simulink model "simulator_prototype_v2"  (R2021b)
(part 8 of 12)

tau_c = ft_11({t1005,t1022,t1089,t1104,t1105,t1108,t1115,t1121,t1158,t1159,t1196,t1205,t1207,t1208,t1210,t1212,t1217,t1218,t1221,t123,t1230,t1235,t1237,t1238,t1288,t1289,t1302,t1303,t1319,t1320,t1336,t1348,t1350,t1351,t1360,t1369,t1378,t1396,t14,t140,t1425,t1435,t1456,t1477,t1488,t15,t1513,t1539,t1544,t1547,t1548,t1553,t1554,t1559,t1564,t1576,t1577,t1578,t1579,t1584,t1585,t1586,t1587,t1591,t1599,t16,t1600,t1602,t1604,t1605,t1606,t1607,t1608,t1609,t1613,t1614,t1615,t1616,t1626,t1627,t1628,t1629,t1631,t1637,t1640,t1641,t1648,t1649,t1659,t1660,t1661,t1666,t1667,t1683,t1686,t1690,t1692,t17,t1700,t1701,t1704,t1705,t1712,t1717,t1738,t1741,t1742,t1750,t1752,t1753,t1754,t1758,t1759,t1775,t1776,t18,t1861,t1874,t1879,t188,t1881,t189,t1896,t19,t1901,t1941,t1959,t1973,t1993,t1994,t2,t20,t201,t202,t2023,t2053,t2060,t2089,t2090,t2098,t2099,t21,t2117,t2120,t2122,t2123,t2125,t2137,t2139,t2140,t2142,t2147,t2149,t2150,t2151,t2152,t2154,t2155,t2159,t2164,t2165,t2166,t2167,t2168,t2174,t2183,t2187,t2193,t2194,t2195,t2199,t22,t2203,t2215,t2219,t2222,t2223,t2239,t2240,t2256,t2257,t2291,t2292,t2293,t2294,t2295,t2297,t2298,t2299,t23,t2301,t2302,t2303,t2304,t2306,t2307,t2308,t2311,t2317,t2320,t2323,t2325,t2326,t2329,t2337,t2338,t2339,t2341,t2343,t2344,t2352,t2353,t2355,t2359,t236,t2360,t2361,t2362,t2363,t2364,t2365,t2366,t2367,t2368,t2369,t237,t2370,t2371,t2378,t2379,t238,t2380,t2384,t2388,t2389,t2391,t2394,t2395,t2397,t2398,t24,t2400,t2401,t2403,t2404,t2405,t241,t2414,t2419,t2421,t2423,t2438,t244,t2448,t2449,t2461,t2471,t2472,t2492,t2493,t2494,t25,t2502,t2510,t2519,t2527,t2530,t2534,t2555,t2556,t2572,t2575,t2583,t2598,t26,t2605,t2606,t2612,t2613,t2618,t2619,t262,t2638,t264,t2651,t2652,t2670,t2671,t2673,t2674,t2675,t2676,t2678,t2680,t2683,t2684,t2685,t2686,t2687,t2689,t2690,t2692,t2693,t2694,t2695,t2696,t2697,t2698,t27,t2700,t2701,t2704,t2705,t2707,t2708,t2709,t2711,t2712,t2713,t2715,t2716,t2717,t2719,t2720,t2721,t2736,t2740,t2744,t2745,t2747,t2748,t2749,t2750,t2754,t2759,t2773,t2774,t2777,t2778,t2779,t2781,t2785,t2786,t2787,t2788,t2797,t28,t2801,t2804,t2813,t2814,t2820,t2831,t2834,t2835,t2838,t2850,t2851,t2937,t2942,t2945,t2946,t2950,t2951,t2953,t2954,t2955,t2956,t2957,t2963,t2964,t2975,t2978,t2979,t2984,t2987,t2990,t2991,t2993,t2994,t2998,t3,t30,t3003,t3004,t3008,t3009,t3015,t3017,t3022,t3027,t3029,t3030,t3036,t3043,t3044,t3045,t3047,t3049,t3050,t3051,t3054,t3055,t3056,t3057,t3063,t3064,t3066,t3067,t3068,t3072,t3073,t3079,t3080,t3081,t3085,t3086,t3087,t3088,t3096,t3097,t31,t3109,t3117,t3118,t3121,t3122,t3128,t3129,t313,t3130,t3131,t3132,t3133,t3134,t3135,t3139,t314,t3140,t3141,t3142,t3144,t3147,t3149,t3152,t3153,t3155,t3156,t3157,t3158,t3159,t3160,t3161,t3162,t3163,t3164,t3166,t3170,t3171,t3172,t3179,t3180,t3184,t3186,t3187,t3188,t3189,t3190,t3191,t3193,t3194,t3196,t3197,t3198,t3199,t32,t3200,t3201,t3204,t3206,t3209,t321,t3210,t3212,t3214,t3218,t3223,t3224,t3225,t3226,t3227,t3228,t3229,t3230,t3231,t3232,t3235,t3245,t3246,t3247,t3249,t3250,t3252,t3253,t3254,t3256,t3258,t3259,t326,t3260,t3261,t3262,t3263,t3264,t3265,t3266,t3269,t3270,t3271,t3272,t3275,t3276,t3277,t328,t3280,t3281,t3283,t3284,t3287,t329,t3290,t3291,t3292,t3293,t3295,t3296,t3297,t3298,t33,t3300,t3302,t3303,t3305,t3306,t3307,t3308,t3309,t331,t3313,t3316,t3318,t3319,t332,t3322,t3323,t3324,t3325,t3326,t3327,t3328,t333,t3330,t3331,t3333,t3334,t3335,t3336,t3337,t3338,t3340,t3341,t3342,t3343,t3344,t3345,t3347,t3348,t3349,t335,t3351,t3353,t3354,t3355,t3357,t3358,t3359,t3360,t3367,t3369,t3373,t3376,t3377,t3379,t338,t3382,t3384,t3385,t3386,t3389,t339,t3392,t3395,t3399,t34,t3405,t3408,t3409,t3410,t3412,t3415,t3417,t3419,t3420,t3421,t3422,t3423,t3424,t3427,t3428,t3429,t3430,t3432,t3433,t3434,t3435,t3436,t3437,t3438,t3440,t3441,t3442,t3443,t3444,t3445,t3446,t3447,t3449,t3450,t3451,t3453,t3455,t3456,t3457,t3458,t346,t3465,t3468,t3470,t3473,t3475,t3477,t3479,t3480,t3481,t3483,t3484,t3489,t3491,t3493,t3498,t35,t350,t3500,t3503,t3505,t3508,t3509,t351,t3510,t3512,t3513,t3515,t3518,t3522,t3524,t3526,t3527,t3528,t3530,t3531,t3532,t3533,t3535,t3539,t354,t3542,t3543,t3544,t3547,t3549,t3550,t3558,t3559,t356,t3560,t3561,t3562,t3563,t3564,t3565,t3567,t3569,t3570,t3571,t3572,t3573,t3576,t3577,t3578,t3579,t358,t3580,t3581,t3582,t3584,t3585,t3586,t3587,t3588,t3589,t359,t3590,t3591,t3593,t3595,t3596,t3597,t3598,t36,t360,t3600,t3603,t3605,t3607,t3609,t3610,t3611,t3612,t3613,t3614,t3615,t3616,t3617,t3618,t3619,t362,t3620,t3621,t3622,t3623,t3624,t3625,t3626,t3627,t3628,t3629,t363,t3630,t3631,t3632,t3633,t3634,t3635,t3636,t3637,t3638,t3639,t364,t3640,t3641,t3643,t3645,t3646,t3647,t3648,t3649,t365,t3650,t3651,t3652,t3653,t3654,t3656,t3657,t3658,t3659,t366,t3660,t3662,t3663,t3664,t3665,t3667,t3669,t3670,t3672,t3673,t3674,t3676,t3677,t3678,t3679,t3680,t3681,t3682,t3683,t3684,t3685,t3686,t3687,t3688,t3689,t3690,t3693,t3694,t3696,t3698,t3699,t3700,t3703,t3705,t3706,t3708,t3709,t371,t3711,t3712,t3713,t3714,t3715,t3716,t3718,t372,t3720,t3723,t3724,t3726,t3728,t3729,t3730,t3731,t3732,t3734,t3735,t3736,t3737,t3741,t3744,t3745,t3746,t3748,t3749,t3751,t3753,t3755,t3756,t3757,t3758,t3759,t3760,t3762,t3763,t3764,t3765,t3766,t3767,t3768,t3769,t3770,t3771,t3772,t3774,t3775,t3776,t3778,t3779,t378,t3782,t3783,t3784,t3788,t3789,t3790,t3791,t3793,t3794,t3795,t3797,t3798,t3799,t38,t380,t3801,t3803,t3804,t3805,t3806,t3811,t3814,t3815,t3816,t3817,t3819,t382,t3821,t3822,t3826,t3827,t3828,t3830,t3833,t3834,t3837,t3838,t3841,t3844,t3845,t3847,t3849,t3850,t3856,t3859,t3860,t3861,t3862,t3863,t3865,t3866,t3868,t3869,t387,t3870,t3871,t3872,t3875,t3876,t3877,t3880,t3882,t3886,t3891,t3892,t3893,t3898,t39,t3901,t3904,t3906,t3908,t3910,t3916,t3918,t3920,t3921,t3922,t3925,t3926,t3927,t3928,t3933,t3934,t3936,t3937,t3939,t3940,t3941,t3942,t3943,t3945,t3946,t3949,t3951,t3953,t3954,t3957,t3958,t3959,t3962,t3963,t3964,t3965,t3967,t3968,t3974,t3976,t3977,t3978,t3980,t3981,t3982,t3983,t3984,t3985,t3992,t3996,t3997,t4,t4002,t4007,t4008,t4009,t4010,t4011,t4012,t4021,t4022,t4025,t4026,t4027,t4028,t4033,t4048,t4052,t4053,t4054,t4058,t4059,t4060,t4061,t4062,t4063,t4065,t4067,t4069,t4070,t4071,t4072,t4073,t4074,t4078,t4079,t4080,t4083,t4084,t410,t4106,t4108,t4109,t4111,t4113,t4118,t4119,t4120,t4121,t4122,t4125,t4127,t4133,t4134,t4141,t4142,t4149,t4150,t4151,t4152,t4154,t4155,t4157,t4160,t4162,t4163,t4166,t4168,t4170,t4173,t4175,t4178,t4179,t4184,t4189,t4190,t4196,t4197,t42,t4200,t4201,t4202,t4203,t4205,t4207,t4208,t4217,t4219,t4220,t4221,t4224,t4227,t4228,t4230,t4231,t4233,t4234,t4235,t4236,t4237,t4238,t4239,t4240,t4242,t4243,t4244,t4245,t4246,t4247,t4249,t4250,t4251,t4252,t4253,t4254,t4255,t4256,t4257,t4259,t4260,t4261,t4262,t4263,t4264,t4266,t4267,t4268,t4274,t4275,t4277,t4278,t4279,t4280,t4281,t4285,t4286,t4287,t4288,t429,t4291,t4292,t4295,t4296,t4297,t4298,t4299,t43,t4304,t4306,t4307,t4308,t4310,t4311,t4313,t4314,t4321,t4322,t4323,t4324,t4326,t4353,t4354,t4355,t4356,t4357,t4359,t4362,t4363,t4367,t4369,t4370,t4373,t4374,t4375,t4376,t4377,t4378,t4379,t4381,t4382,t4383,t4385,t4386,t4387,t4388,t4390,t4395,t4396,t4400,t4402,t4403,t4404,t4405,t4406,t4407,t4409,t4410,t4411,t4412,t4413,t4415,t4421,t4424,t4427,t4428,t4429,t4430,t4431,t4432,t4434,t4435,t4436,t4437,t4438,t4439,t4440,t4441,t4442,t4443,t4444,t4447,t4453,t4458,t4460,t4461,t4464,t4470,t4473,t4474,t4475,t4480,t4481,t4483,t4484,t4486,t4487,t4488,t4489,t4491,t4492,t4496,t4498,t4499,t4500,t4501,t4502,t4504,t4507,t4508,t4510,t4511,t4513,t4514,t4515,t4516,t4517,t4520,t4521,t4522,t4525,t4526,t4528,t4530,t4531,t4532,t4533,t4535,t4536,t4539,t4542,t4543,t4545,t4546,t4549,t4550,t4551,t4552,t4555,t4560,t4562,t4563,t4571,t4572,t4574,t4579,t4581,t4582,t4583,t4584,t4585,t4586,t4587,t4588,t4589,t4591,t4593,t4594,t4595,t4597,t4599,t46,t4602,t4604,t4606,t4607,t4609,t4610,t4611,t4612,t4613,t4614,t4615,t4617,t4618,t4619,t4620,t4621,t4622,t4623,t4624,t4627,t4628,t4629,t4631,t4633,t4640,t4641,t4642,t4644,t4645,t4647,t4649,t4650,t4651,t4652,t4655,t4657,t4658,t4661,t4663,t4664,t4665,t4666,t4667,t4669,t4670,t4672,t4673,t4676,t4678,t4679,t4680,t4682,t4683,t4684,t4685,t4686,t4688,t4699,t47,t4702,t4703,t4704,t4705,t4706,t4708,t4709,t4710,t4711,t4716,t4718,t4719,t4720,t4721,t4723,t4725,t4726,t4727,t4728,t4729,t4732,t4733,t4734,t4735,t4736,t4737,t4738,t4740,t4741,t4742,t4744,t4746,t4749,t4756,t4758,t4759,t4760,t4762,t4764,t4768,t4769,t4770,t4772,t4777,t4780,t4785,t4786,t4787,t4788,t4789,t4790,t4791,t4792,t4795,t4798,t4799,t4800,t4801,t4805,t4809,t4814,t4816,t4817,t4818,t4819,t4822,t4823,t4824,t4826,t4828,t4829,t4832,t4833,t4836,t4839,t4840,t4842,t4843,t4845,t4846,t4847,t4849,t4852,t4856,t4857,t4860,t4863,t4864,t4865,t4866,t4867,t4868,t4869,t4870,t4871,t4872,t4873,t4874,t4875,t4876,t4877,t4880,t4881,t4882,t4883,t4884,t4885,t4886,t4887,t4888,t4890,t4892,t4893,t4894,t4897,t4898,t4899,t4900,t4902,t4905,t4911,t4917,t4921,t4922,t4925,t4927,t4931,t4950,t4952,t4953,t4954,t4961,t4962,t4963,t4965,t4968,t4969,t4973,t4974,t4975,t4976,t4977,t4982,t4983,t4984,t4985,t4986,t4987,t4992,t4994,t4995,t4996,t4998,t5,t50,t5000,t5001,t5002,t5005,t5007,t5010,t5012,t5013,t5014,t5015,t5017,t5021,t5022,t5023,t5025,t5026,t5027,t5028,t5030,t5031,t5032,t5033,t5034,t5035,t5036,t5038,t5039,t5040,t5041,t5042,t5047,t5048,t5049,t5051,t5052,t5053,t5054,t5056,t5058,t5061,t5063,t5064,t5067,t5068,t5069,t5073,t5074,t5076,t5077,t5091,t5092,t5094,t5096,t5105,t5108,t5111,t5113,t5114,t5115,t5116,t5118,t5119,t5121,t5123,t5124,t5126,t5127,t5128,t5130,t5131,t5144,t5145,t5146,t5147,t5148,t5149,t5150,t5151,t5152,t5153,t5155,t5158,t5162,t5164,t5165,t5169,t5184,t5189,t5190,t5191,t5192,t5193,t5195,t5196,t5198,t5201,t5202,t5203,t5204,t5206,t5207,t5208,t5209,t5210,t5211,t5212,t5213,t5214,t5216,t5217,t5218,t5219,t5221,t5222,t5223,t5224,t5225,t5226,t5227,t5228,t5229,t5230,t5231,t5232,t5233,t5234,t5235,t5236,t5237,t5238,t5239,t5240,t5241,t5242,t5243,t5244,t5245,t5246,t5247,t5248,t5249,t5250,t5252,t5254,t5255,t5257,t5260,t5261,t5263,t5265,t5266,t5267,t5269,t5270,t5272,t5273,t5274,t5275,t5276,t5277,t5281,t5282,t5285,t5288,t5289,t5290,t5291,t5293,t5295,t5298,t5299,t5301,t5302,t5303,t5304,t5306,t5307,t5308,t5316,t5317,t5320,t5322,t5325,t5328,t5330,t5331,t5332,t5335,t5337,t5338,t5339,t5340,t5342,t5344,t5345,t5346,t5347,t5348,t5349,t5350,t5356,t5357,t5358,t5361,t5362,t5365,t5369,t5370,t5377,t5379,t5380,t5381,t5383,t5384,t5385,t5386,t5387,t5388,t5389,t5390,t5391,t5392,t5393,t5395,t5396,t5399,t5402,t5403,t5405,t5407,t5408,t5409,t5411,t5412,t5418,t5420,t5427,t5428,t5433,t5434,t5440,t5441,t5443,t5444,t5445,t5446,t5449,t5455,t5458,t5461,t5462,t5465,t5480,t5481,t5482,t5483,t5484,t5485,t5486,t5487,t5488,t5489,t5490,t5491,t5492,t5493,t5494,t5496,t5498,t5499,t5500,t5504,t5505,t5509,t5510,t5514,t5515,t5516,t5517,t5518,t5522,t5523,t5524,t5525,t5531,t5535,t5536,t5537,t5540,t5544,t5547,t5550,t5552,t5553,t5554,t5556,t5557,t5565,t5566,t5571,t5578,t5580,t5595,t56,t5601,t5603,t5605,t5619,t5620,t5626,t5627,t5631,t5639,t5640,t5646,t5661,t5662,t5663,t5670,t5671,t5674,t5675,t5677,t5678,t5679,t5681,t5682,t5684,t5694,t5695,t5699,t5700,t5701,t5702,t5703,t5709,t5717,t5718,t5720,t5721,t5722,t5723,t5724,t5730,t5734,t5750,t5760,t5764,t5769,t5791,t5792,t5794,t58,t5832,t5835,t5839,t5840,t5846,t5852,t5853,t5857,t5864,t5866,t5871,t5876,t5879,t5890,t5891,t59,t5900,t5909,t5911,t5930,t5932,t5941,t5943,t5944,t5951,t5953,t5954,t5977,t5992,t5994,t5995,t6,t60,t6004,t6017,t6018,t6020,t6057,t6058,t6065,t6075,t6095,t6135,t6151,t6153,t6183,t6184,t6185,t6199,t6206,t6207,t6209,t6219,t6221,t6247,t6253,t628,t6317,t6321,t6323,t6339,t6341,t6367,t6375,t638,t640,t6405,t642,t643,t6450,t6484,t6485,t6486,t649,t6493,t6507,t6508,t6511,t6515,t6516,t654,t6543,t6544,t655,t656,t6565,t657,t659,t660,t665,t6658,t6663,t667,t668,t6689,t669,t6691,t6692,t67,t670,t672,t673,t674,t675,t676,t677,t68,t681,t6811,t6812,t6813,t682,t684,t685,t686,t6861,t687,t6892,t6893,t691,t6916,t692,t693,t694,t6980,t6981,t7,t70,t702,t7029,t7039,t7041,t7043,t7051,t7064,t707,t708,t71,t710,t715,t716,t717,t718,t7204,t721,t7219,t722,t7227,t7228,t7229,t7230,t724,t725,t73,t736,t738,t740,t741,t749,t756,t76,t762,t768,t777,t792,t793,t801,t802,t808,t813,t819,t821,t850,t855,t874,t878,t89,t90,t91,t92,t941,t944,t948,t951,t97});
end
function tau_c = ft_11(ct)
t1005 = ct{1};
t1022 = ct{2};
t1089 = ct{3};
t1104 = ct{4};
t1105 = ct{5};
t1108 = ct{6};
t1115 = ct{7};
t1121 = ct{8};
t1158 = ct{9};
t1159 = ct{10};
t1196 = ct{11};
t1205 = ct{12};
t1207 = ct{13};
t1208 = ct{14};
t1210 = ct{15};
t1212 = ct{16};
t1217 = ct{17};
t1218 = ct{18};
t1221 = ct{19};
t123 = ct{20};
t1230 = ct{21};
t1235 = ct{22};
t1237 = ct{23};
t1238 = ct{24};
t1288 = ct{25};
t1289 = ct{26};
t1302 = ct{27};
t1303 = ct{28};
t1319 = ct{29};
t1320 = ct{30};
t1336 = ct{31};
t1348 = ct{32};
t1350 = ct{33};
t1351 = ct{34};
t1360 = ct{35};
t1369 = ct{36};
t1378 = ct{37};
t1396 = ct{38};
t14 = ct{39};
t140 = ct{40};
t1425 = ct{41};
t1435 = ct{42};
t1456 = ct{43};
t1477 = ct{44};
t1488 = ct{45};
t15 = ct{46};
t1513 = ct{47};
t1539 = ct{48};
t1544 = ct{49};
t1547 = ct{50};
t1548 = ct{51};
t1553 = ct{52};
t1554 = ct{53};
t1559 = ct{54};
t1564 = ct{55};
t1576 = ct{56};
t1577 = ct{57};
t1578 = ct{58};
t1579 = ct{59};
t1584 = ct{60};
t1585 = ct{61};
t1586 = ct{62};
t1587 = ct{63};
t1591 = ct{64};
t1599 = ct{65};
t16 = ct{66};
t1600 = ct{67};
t1602 = ct{68};
t1604 = ct{69};
t1605 = ct{70};
t1606 = ct{71};
t1607 = ct{72};
t1608 = ct{73};
t1609 = ct{74};
t1613 = ct{75};
t1614 = ct{76};
t1615 = ct{77};
t1616 = ct{78};
t1626 = ct{79};
t1627 = ct{80};
t1628 = ct{81};
t1629 = ct{82};
t1631 = ct{83};
t1637 = ct{84};
t1640 = ct{85};
t1641 = ct{86};
t1648 = ct{87};
t1649 = ct{88};
t1659 = ct{89};
t1660 = ct{90};
t1661 = ct{91};
t1666 = ct{92};
t1667 = ct{93};
t1683 = ct{94};
t1686 = ct{95};
t1690 = ct{96};
t1692 = ct{97};
t17 = ct{98};
t1700 = ct{99};
t1701 = ct{100};
t1704 = ct{101};
t1705 = ct{102};
t1712 = ct{103};
t1717 = ct{104};
t1738 = ct{105};
t1741 = ct{106};
t1742 = ct{107};
t1750 = ct{108};
t1752 = ct{109};
t1753 = ct{110};
t1754 = ct{111};
t1758 = ct{112};
t1759 = ct{113};
t1775 = ct{114};
t1776 = ct{115};
t18 = ct{116};
t1861 = ct{117};
t1874 = ct{118};
t1879 = ct{119};
t188 = ct{120};
t1881 = ct{121};
t189 = ct{122};
t1896 = ct{123};
t19 = ct{124};
t1901 = ct{125};
t1941 = ct{126};
t1959 = ct{127};
t1973 = ct{128};
t1993 = ct{129};
t1994 = ct{130};
t2 = ct{131};
t20 = ct{132};
t201 = ct{133};
t202 = ct{134};
t2023 = ct{135};
t2053 = ct{136};
t2060 = ct{137};
t2089 = ct{138};
t2090 = ct{139};
t2098 = ct{140};
t2099 = ct{141};
t21 = ct{142};
t2117 = ct{143};
t2120 = ct{144};
t2122 = ct{145};
t2123 = ct{146};
t2125 = ct{147};
t2137 = ct{148};
t2139 = ct{149};
t2140 = ct{150};
t2142 = ct{151};
t2147 = ct{152};
t2149 = ct{153};
t2150 = ct{154};
t2151 = ct{155};
t2152 = ct{156};
t2154 = ct{157};
t2155 = ct{158};
t2159 = ct{159};
t2164 = ct{160};
t2165 = ct{161};
t2166 = ct{162};
t2167 = ct{163};
t2168 = ct{164};
t2174 = ct{165};
t2183 = ct{166};
t2187 = ct{167};
t2193 = ct{168};
t2194 = ct{169};
t2195 = ct{170};
t2199 = ct{171};
t22 = ct{172};
t2203 = ct{173};
t2215 = ct{174};
t2219 = ct{175};
t2222 = ct{176};
t2223 = ct{177};
t2239 = ct{178};
t2240 = ct{179};
t2256 = ct{180};
t2257 = ct{181};
t2291 = ct{182};
t2292 = ct{183};
t2293 = ct{184};
t2294 = ct{185};
t2295 = ct{186};
t2297 = ct{187};
t2298 = ct{188};
t2299 = ct{189};
t23 = ct{190};
t2301 = ct{191};
t2302 = ct{192};
t2303 = ct{193};
t2304 = ct{194};
t2306 = ct{195};
t2307 = ct{196};
t2308 = ct{197};
t2311 = ct{198};
t2317 = ct{199};
t2320 = ct{200};
t2323 = ct{201};
t2325 = ct{202};
t2326 = ct{203};
t2329 = ct{204};
t2337 = ct{205};
t2338 = ct{206};
t2339 = ct{207};
t2341 = ct{208};
t2343 = ct{209};
t2344 = ct{210};
t2352 = ct{211};
t2353 = ct{212};
t2355 = ct{213};
t2359 = ct{214};
t236 = ct{215};
t2360 = ct{216};
t2361 = ct{217};
t2362 = ct{218};
t2363 = ct{219};
t2364 = ct{220};
t2365 = ct{221};
t2366 = ct{222};
t2367 = ct{223};
t2368 = ct{224};
t2369 = ct{225};
t237 = ct{226};
t2370 = ct{227};
t2371 = ct{228};
t2378 = ct{229};
t2379 = ct{230};
t238 = ct{231};
t2380 = ct{232};
t2384 = ct{233};
t2388 = ct{234};
t2389 = ct{235};
t2391 = ct{236};
t2394 = ct{237};
t2395 = ct{238};
t2397 = ct{239};
t2398 = ct{240};
t24 = ct{241};
t2400 = ct{242};
t2401 = ct{243};
t2403 = ct{244};
t2404 = ct{245};
t2405 = ct{246};
t241 = ct{247};
t2414 = ct{248};
t2419 = ct{249};
t2421 = ct{250};
t2423 = ct{251};
t2438 = ct{252};
t244 = ct{253};
t2448 = ct{254};
t2449 = ct{255};
t2461 = ct{256};
t2471 = ct{257};
t2472 = ct{258};
t2492 = ct{259};
t2493 = ct{260};
t2494 = ct{261};
t25 = ct{262};
t2502 = ct{263};
t2510 = ct{264};
t2519 = ct{265};
t2527 = ct{266};
t2530 = ct{267};
t2534 = ct{268};
t2555 = ct{269};
t2556 = ct{270};
t2572 = ct{271};
t2575 = ct{272};
t2583 = ct{273};
t2598 = ct{274};
t26 = ct{275};
t2605 = ct{276};
t2606 = ct{277};
t2612 = ct{278};
t2613 = ct{279};
t2618 = ct{280};
t2619 = ct{281};
t262 = ct{282};
t2638 = ct{283};
t264 = ct{284};
t2651 = ct{285};
t2652 = ct{286};
t2670 = ct{287};
t2671 = ct{288};
t2673 = ct{289};
t2674 = ct{290};
t2675 = ct{291};
t2676 = ct{292};
t2678 = ct{293};
t2680 = ct{294};
t2683 = ct{295};
t2684 = ct{296};
t2685 = ct{297};
t2686 = ct{298};
t2687 = ct{299};
t2689 = ct{300};
t2690 = ct{301};
t2692 = ct{302};
t2693 = ct{303};
t2694 = ct{304};
t2695 = ct{305};
t2696 = ct{306};
t2697 = ct{307};
t2698 = ct{308};
t27 = ct{309};
t2700 = ct{310};
t2701 = ct{311};
t2704 = ct{312};
t2705 = ct{313};
t2707 = ct{314};
t2708 = ct{315};
t2709 = ct{316};
t2711 = ct{317};
t2712 = ct{318};
t2713 = ct{319};
t2715 = ct{320};
t2716 = ct{321};
t2717 = ct{322};
t2719 = ct{323};
t2720 = ct{324};
t2721 = ct{325};
t2736 = ct{326};
t2740 = ct{327};
t2744 = ct{328};
t2745 = ct{329};
t2747 = ct{330};
t2748 = ct{331};
t2749 = ct{332};
t2750 = ct{333};
t2754 = ct{334};
t2759 = ct{335};
t2773 = ct{336};
t2774 = ct{337};
t2777 = ct{338};
t2778 = ct{339};
t2779 = ct{340};
t2781 = ct{341};
t2785 = ct{342};
t2786 = ct{343};
t2787 = ct{344};
t2788 = ct{345};
t2797 = ct{346};
t28 = ct{347};
t2801 = ct{348};
t2804 = ct{349};
t2813 = ct{350};
t2814 = ct{351};
t2820 = ct{352};
t2831 = ct{353};
t2834 = ct{354};
t2835 = ct{355};
t2838 = ct{356};
t2850 = ct{357};
t2851 = ct{358};
t2937 = ct{359};
t2942 = ct{360};
t2945 = ct{361};
t2946 = ct{362};
t2950 = ct{363};
t2951 = ct{364};
t2953 = ct{365};
t2954 = ct{366};
t2955 = ct{367};
t2956 = ct{368};
t2957 = ct{369};
t2963 = ct{370};
t2964 = ct{371};
t2975 = ct{372};
t2978 = ct{373};
t2979 = ct{374};
t2984 = ct{375};
t2987 = ct{376};
t2990 = ct{377};
t2991 = ct{378};
t2993 = ct{379};
t2994 = ct{380};
t2998 = ct{381};
t3 = ct{382};
t30 = ct{383};
t3003 = ct{384};
t3004 = ct{385};
t3008 = ct{386};
t3009 = ct{387};
t3015 = ct{388};
t3017 = ct{389};
t3022 = ct{390};
t3027 = ct{391};
t3029 = ct{392};
t3030 = ct{393};
t3036 = ct{394};
t3043 = ct{395};
t3044 = ct{396};
t3045 = ct{397};
t3047 = ct{398};
t3049 = ct{399};
t3050 = ct{400};
t3051 = ct{401};
t3054 = ct{402};
t3055 = ct{403};
t3056 = ct{404};
t3057 = ct{405};
t3063 = ct{406};
t3064 = ct{407};
t3066 = ct{408};
t3067 = ct{409};
t3068 = ct{410};
t3072 = ct{411};
t3073 = ct{412};
t3079 = ct{413};
t3080 = ct{414};
t3081 = ct{415};
t3085 = ct{416};
t3086 = ct{417};
t3087 = ct{418};
t3088 = ct{419};
t3096 = ct{420};
t3097 = ct{421};
t31 = ct{422};
t3109 = ct{423};
t3117 = ct{424};
t3118 = ct{425};
t3121 = ct{426};
t3122 = ct{427};
t3128 = ct{428};
t3129 = ct{429};
t313 = ct{430};
t3130 = ct{431};
t3131 = ct{432};
t3132 = ct{433};
t3133 = ct{434};
t3134 = ct{435};
t3135 = ct{436};
t3139 = ct{437};
t314 = ct{438};
t3140 = ct{439};
t3141 = ct{440};
t3142 = ct{441};
t3144 = ct{442};
t3147 = ct{443};
t3149 = ct{444};
t3152 = ct{445};
t3153 = ct{446};
t3155 = ct{447};
t3156 = ct{448};
t3157 = ct{449};
t3158 = ct{450};
t3159 = ct{451};
t3160 = ct{452};
t3161 = ct{453};
t3162 = ct{454};
t3163 = ct{455};
t3164 = ct{456};
t3166 = ct{457};
t3170 = ct{458};
t3171 = ct{459};
t3172 = ct{460};
t3179 = ct{461};
t3180 = ct{462};
t3184 = ct{463};
t3186 = ct{464};
t3187 = ct{465};
t3188 = ct{466};
t3189 = ct{467};
t3190 = ct{468};
t3191 = ct{469};
t3193 = ct{470};
t3194 = ct{471};
t3196 = ct{472};
t3197 = ct{473};
t3198 = ct{474};
t3199 = ct{475};
t32 = ct{476};
t3200 = ct{477};
t3201 = ct{478};
t3204 = ct{479};
t3206 = ct{480};
t3209 = ct{481};
t321 = ct{482};
t3210 = ct{483};
t3212 = ct{484};
t3214 = ct{485};
t3218 = ct{486};
t3223 = ct{487};
t3224 = ct{488};
t3225 = ct{489};
t3226 = ct{490};
t3227 = ct{491};
t3228 = ct{492};
t3229 = ct{493};
t3230 = ct{494};
t3231 = ct{495};
t3232 = ct{496};
t3235 = ct{497};
t3245 = ct{498};
t3246 = ct{499};
t3247 = ct{500};
t3249 = ct{501};
t3250 = ct{502};
t3252 = ct{503};
t3253 = ct{504};
t3254 = ct{505};
t3256 = ct{506};
t3258 = ct{507};
t3259 = ct{508};
t326 = ct{509};
t3260 = ct{510};
t3261 = ct{511};
t3262 = ct{512};
t3263 = ct{513};
t3264 = ct{514};
t3265 = ct{515};
t3266 = ct{516};
t3269 = ct{517};
t3270 = ct{518};
t3271 = ct{519};
t3272 = ct{520};
t3275 = ct{521};
t3276 = ct{522};
t3277 = ct{523};
t328 = ct{524};
t3280 = ct{525};
t3281 = ct{526};
t3283 = ct{527};
t3284 = ct{528};
t3287 = ct{529};
t329 = ct{530};
t3290 = ct{531};
t3291 = ct{532};
t3292 = ct{533};
t3293 = ct{534};
t3295 = ct{535};
t3296 = ct{536};
t3297 = ct{537};
t3298 = ct{538};
t33 = ct{539};
t3300 = ct{540};
t3302 = ct{541};
t3303 = ct{542};
t3305 = ct{543};
t3306 = ct{544};
t3307 = ct{545};
t3308 = ct{546};
t3309 = ct{547};
t331 = ct{548};
t3313 = ct{549};
t3316 = ct{550};
t3318 = ct{551};
t3319 = ct{552};
t332 = ct{553};
t3322 = ct{554};
t3323 = ct{555};
t3324 = ct{556};
t3325 = ct{557};
t3326 = ct{558};
t3327 = ct{559};
t3328 = ct{560};
t333 = ct{561};
t3330 = ct{562};
t3331 = ct{563};
t3333 = ct{564};
t3334 = ct{565};
t3335 = ct{566};
t3336 = ct{567};
t3337 = ct{568};
t3338 = ct{569};
t3340 = ct{570};
t3341 = ct{571};
t3342 = ct{572};
t3343 = ct{573};
t3344 = ct{574};
t3345 = ct{575};
t3347 = ct{576};
t3348 = ct{577};
t3349 = ct{578};
t335 = ct{579};
t3351 = ct{580};
t3353 = ct{581};
t3354 = ct{582};
t3355 = ct{583};
t3357 = ct{584};
t3358 = ct{585};
t3359 = ct{586};
t3360 = ct{587};
t3367 = ct{588};
t3369 = ct{589};
t3373 = ct{590};
t3376 = ct{591};
t3377 = ct{592};
t3379 = ct{593};
t338 = ct{594};
t3382 = ct{595};
t3384 = ct{596};
t3385 = ct{597};
t3386 = ct{598};
t3389 = ct{599};
t339 = ct{600};
t3392 = ct{601};
t3395 = ct{602};
t3399 = ct{603};
t34 = ct{604};
t3405 = ct{605};
t3408 = ct{606};
t3409 = ct{607};
t3410 = ct{608};
t3412 = ct{609};
t3415 = ct{610};
t3417 = ct{611};
t3419 = ct{612};
t3420 = ct{613};
t3421 = ct{614};
t3422 = ct{615};
t3423 = ct{616};
t3424 = ct{617};
t3427 = ct{618};
t3428 = ct{619};
t3429 = ct{620};
t3430 = ct{621};
t3432 = ct{622};
t3433 = ct{623};
t3434 = ct{624};
t3435 = ct{625};
t3436 = ct{626};
t3437 = ct{627};
t3438 = ct{628};
t3440 = ct{629};
t3441 = ct{630};
t3442 = ct{631};
t3443 = ct{632};
t3444 = ct{633};
t3445 = ct{634};
t3446 = ct{635};
t3447 = ct{636};
t3449 = ct{637};
t3450 = ct{638};
t3451 = ct{639};
t3453 = ct{640};
t3455 = ct{641};
t3456 = ct{642};
t3457 = ct{643};
t3458 = ct{644};
t346 = ct{645};
t3465 = ct{646};
t3468 = ct{647};
t3470 = ct{648};
t3473 = ct{649};
t3475 = ct{650};
t3477 = ct{651};
t3479 = ct{652};
t3480 = ct{653};
t3481 = ct{654};
t3483 = ct{655};
t3484 = ct{656};
t3489 = ct{657};
t3491 = ct{658};
t3493 = ct{659};
t3498 = ct{660};
t35 = ct{661};
t350 = ct{662};
t3500 = ct{663};
t3503 = ct{664};
t3505 = ct{665};
t3508 = ct{666};
t3509 = ct{667};
t351 = ct{668};
t3510 = ct{669};
t3512 = ct{670};
t3513 = ct{671};
t3515 = ct{672};
t3518 = ct{673};
t3522 = ct{674};
t3524 = ct{675};
t3526 = ct{676};
t3527 = ct{677};
t3528 = ct{678};
t3530 = ct{679};
t3531 = ct{680};
t3532 = ct{681};
t3533 = ct{682};
t3535 = ct{683};
t3539 = ct{684};
t354 = ct{685};
t3542 = ct{686};
t3543 = ct{687};
t3544 = ct{688};
t3547 = ct{689};
t3549 = ct{690};
t3550 = ct{691};
t3558 = ct{692};
t3559 = ct{693};
t356 = ct{694};
t3560 = ct{695};
t3561 = ct{696};
t3562 = ct{697};
t3563 = ct{698};
t3564 = ct{699};
t3565 = ct{700};
t3567 = ct{701};
t3569 = ct{702};
t3570 = ct{703};
t3571 = ct{704};
t3572 = ct{705};
t3573 = ct{706};
t3576 = ct{707};
t3577 = ct{708};
t3578 = ct{709};
t3579 = ct{710};
t358 = ct{711};
t3580 = ct{712};
t3581 = ct{713};
t3582 = ct{714};
t3584 = ct{715};
t3585 = ct{716};
t3586 = ct{717};
t3587 = ct{718};
t3588 = ct{719};
t3589 = ct{720};
t359 = ct{721};
t3590 = ct{722};
t3591 = ct{723};
t3593 = ct{724};
t3595 = ct{725};
t3596 = ct{726};
t3597 = ct{727};
t3598 = ct{728};
t36 = ct{729};
t360 = ct{730};
t3600 = ct{731};
t3603 = ct{732};
t3605 = ct{733};
t3607 = ct{734};
t3609 = ct{735};
t3610 = ct{736};
t3611 = ct{737};
t3612 = ct{738};
t3613 = ct{739};
t3614 = ct{740};
t3615 = ct{741};
t3616 = ct{742};
t3617 = ct{743};
t3618 = ct{744};
t3619 = ct{745};
t362 = ct{746};
t3620 = ct{747};
t3621 = ct{748};
t3622 = ct{749};
t3623 = ct{750};
t3624 = ct{751};
t3625 = ct{752};
t3626 = ct{753};
t3627 = ct{754};
t3628 = ct{755};
t3629 = ct{756};
t363 = ct{757};
t3630 = ct{758};
t3631 = ct{759};
t3632 = ct{760};
t3633 = ct{761};
t3634 = ct{762};
t3635 = ct{763};
t3636 = ct{764};
t3637 = ct{765};
t3638 = ct{766};
t3639 = ct{767};
t364 = ct{768};
t3640 = ct{769};
t3641 = ct{770};
t3643 = ct{771};
t3645 = ct{772};
t3646 = ct{773};
t3647 = ct{774};
t3648 = ct{775};
t3649 = ct{776};
t365 = ct{777};
t3650 = ct{778};
t3651 = ct{779};
t3652 = ct{780};
t3653 = ct{781};
t3654 = ct{782};
t3656 = ct{783};
t3657 = ct{784};
t3658 = ct{785};
t3659 = ct{786};
t366 = ct{787};
t3660 = ct{788};
t3662 = ct{789};
t3663 = ct{790};
t3664 = ct{791};
t3665 = ct{792};
t3667 = ct{793};
t3669 = ct{794};
t3670 = ct{795};
t3672 = ct{796};
t3673 = ct{797};
t3674 = ct{798};
t3676 = ct{799};
t3677 = ct{800};
t3678 = ct{801};
t3679 = ct{802};
t3680 = ct{803};
t3681 = ct{804};
t3682 = ct{805};
t3683 = ct{806};
t3684 = ct{807};
t3685 = ct{808};
t3686 = ct{809};
t3687 = ct{810};
t3688 = ct{811};
t3689 = ct{812};
t3690 = ct{813};
t3693 = ct{814};
t3694 = ct{815};
t3696 = ct{816};
t3698 = ct{817};
t3699 = ct{818};
t3700 = ct{819};
t3703 = ct{820};
t3705 = ct{821};
t3706 = ct{822};
t3708 = ct{823};
t3709 = ct{824};
t371 = ct{825};
t3711 = ct{826};
t3712 = ct{827};
t3713 = ct{828};
t3714 = ct{829};
t3715 = ct{830};
t3716 = ct{831};
t3718 = ct{832};
t372 = ct{833};
t3720 = ct{834};
t3723 = ct{835};
t3724 = ct{836};
t3726 = ct{837};
t3728 = ct{838};
t3729 = ct{839};
t3730 = ct{840};
t3731 = ct{841};
t3732 = ct{842};
t3734 = ct{843};
t3735 = ct{844};
t3736 = ct{845};
t3737 = ct{846};
t3741 = ct{847};
t3744 = ct{848};
t3745 = ct{849};
t3746 = ct{850};
t3748 = ct{851};
t3749 = ct{852};
t3751 = ct{853};
t3753 = ct{854};
t3755 = ct{855};
t3756 = ct{856};
t3757 = ct{857};
t3758 = ct{858};
t3759 = ct{859};
t3760 = ct{860};
t3762 = ct{861};
t3763 = ct{862};
t3764 = ct{863};
t3765 = ct{864};
t3766 = ct{865};
t3767 = ct{866};
t3768 = ct{867};
t3769 = ct{868};
t3770 = ct{869};
t3771 = ct{870};
t3772 = ct{871};
t3774 = ct{872};
t3775 = ct{873};
t3776 = ct{874};
t3778 = ct{875};
t3779 = ct{876};
t378 = ct{877};
t3782 = ct{878};
t3783 = ct{879};
t3784 = ct{880};
t3788 = ct{881};
t3789 = ct{882};
t3790 = ct{883};
t3791 = ct{884};
t3793 = ct{885};
t3794 = ct{886};
t3795 = ct{887};
t3797 = ct{888};
t3798 = ct{889};
t3799 = ct{890};
t38 = ct{891};
t380 = ct{892};
t3801 = ct{893};
t3803 = ct{894};
t3804 = ct{895};
t3805 = ct{896};
t3806 = ct{897};
t3811 = ct{898};
t3814 = ct{899};
t3815 = ct{900};
t3816 = ct{901};
t3817 = ct{902};
t3819 = ct{903};
t382 = ct{904};
t3821 = ct{905};
t3822 = ct{906};
t3826 = ct{907};
t3827 = ct{908};
t3828 = ct{909};
t3830 = ct{910};
t3833 = ct{911};
t3834 = ct{912};
t3837 = ct{913};
t3838 = ct{914};
t3841 = ct{915};
t3844 = ct{916};
t3845 = ct{917};
t3847 = ct{918};
t3849 = ct{919};
t3850 = ct{920};
t3856 = ct{921};
t3859 = ct{922};
t3860 = ct{923};
t3861 = ct{924};
t3862 = ct{925};
t3863 = ct{926};
t3865 = ct{927};
t3866 = ct{928};
t3868 = ct{929};
t3869 = ct{930};
t387 = ct{931};
t3870 = ct{932};
t3871 = ct{933};
t3872 = ct{934};
t3875 = ct{935};
t3876 = ct{936};
t3877 = ct{937};
t3880 = ct{938};
t3882 = ct{939};
t3886 = ct{940};
t3891 = ct{941};
t3892 = ct{942};
t3893 = ct{943};
t3898 = ct{944};
t39 = ct{945};
t3901 = ct{946};
t3904 = ct{947};
t3906 = ct{948};
t3908 = ct{949};
t3910 = ct{950};
t3916 = ct{951};
t3918 = ct{952};
t3920 = ct{953};
t3921 = ct{954};
t3922 = ct{955};
t3925 = ct{956};
t3926 = ct{957};
t3927 = ct{958};
t3928 = ct{959};
t3933 = ct{960};
t3934 = ct{961};
t3936 = ct{962};
t3937 = ct{963};
t3939 = ct{964};
t3940 = ct{965};
t3941 = ct{966};
t3942 = ct{967};
t3943 = ct{968};
t3945 = ct{969};
t3946 = ct{970};
t3949 = ct{971};
t3951 = ct{972};
t3953 = ct{973};
t3954 = ct{974};
t3957 = ct{975};
t3958 = ct{976};
t3959 = ct{977};
t3962 = ct{978};
t3963 = ct{979};
t3964 = ct{980};
t3965 = ct{981};
t3967 = ct{982};
t3968 = ct{983};
t3974 = ct{984};
t3976 = ct{985};
t3977 = ct{986};
t3978 = ct{987};
t3980 = ct{988};
t3981 = ct{989};
t3982 = ct{990};
t3983 = ct{991};
t3984 = ct{992};
t3985 = ct{993};
t3992 = ct{994};
t3996 = ct{995};
t3997 = ct{996};
t4 = ct{997};
t4002 = ct{998};
t4007 = ct{999};
t4008 = ct{1000};
t4009 = ct{1001};
t4010 = ct{1002};
t4011 = ct{1003};
t4012 = ct{1004};
t4021 = ct{1005};
t4022 = ct{1006};
t4025 = ct{1007};
t4026 = ct{1008};
t4027 = ct{1009};
t4028 = ct{1010};
t4033 = ct{1011};
t4048 = ct{1012};
t4052 = ct{1013};
t4053 = ct{1014};
t4054 = ct{1015};
t4058 = ct{1016};
t4059 = ct{1017};
t4060 = ct{1018};
t4061 = ct{1019};
t4062 = ct{1020};
t4063 = ct{1021};
t4065 = ct{1022};
t4067 = ct{1023};
t4069 = ct{1024};
t4070 = ct{1025};
t4071 = ct{1026};
t4072 = ct{1027};
t4073 = ct{1028};
t4074 = ct{1029};
t4078 = ct{1030};
t4079 = ct{1031};
t4080 = ct{1032};
t4083 = ct{1033};
t4084 = ct{1034};
t410 = ct{1035};
t4106 = ct{1036};
t4108 = ct{1037};
t4109 = ct{1038};
t4111 = ct{1039};
t4113 = ct{1040};
t4118 = ct{1041};
t4119 = ct{1042};
t4120 = ct{1043};
t4121 = ct{1044};
t4122 = ct{1045};
t4125 = ct{1046};
t4127 = ct{1047};
t4133 = ct{1048};
t4134 = ct{1049};
t4141 = ct{1050};
t4142 = ct{1051};
t4149 = ct{1052};
t4150 = ct{1053};
t4151 = ct{1054};
t4152 = ct{1055};
t4154 = ct{1056};
t4155 = ct{1057};
t4157 = ct{1058};
t4160 = ct{1059};
t4162 = ct{1060};
t4163 = ct{1061};
t4166 = ct{1062};
t4168 = ct{1063};
t4170 = ct{1064};
t4173 = ct{1065};
t4175 = ct{1066};
t4178 = ct{1067};
t4179 = ct{1068};
t4184 = ct{1069};
t4189 = ct{1070};
t4190 = ct{1071};
t4196 = ct{1072};
t4197 = ct{1073};
t42 = ct{1074};
t4200 = ct{1075};
t4201 = ct{1076};
t4202 = ct{1077};
t4203 = ct{1078};
t4205 = ct{1079};
t4207 = ct{1080};
t4208 = ct{1081};
t4217 = ct{1082};
t4219 = ct{1083};
t4220 = ct{1084};
t4221 = ct{1085};
t4224 = ct{1086};
t4227 = ct{1087};
t4228 = ct{1088};
t4230 = ct{1089};
t4231 = ct{1090};
t4233 = ct{1091};
t4234 = ct{1092};
t4235 = ct{1093};
t4236 = ct{1094};
t4237 = ct{1095};
t4238 = ct{1096};
t4239 = ct{1097};
t4240 = ct{1098};
t4242 = ct{1099};
t4243 = ct{1100};
t4244 = ct{1101};
t4245 = ct{1102};
t4246 = ct{1103};
t4247 = ct{1104};
t4249 = ct{1105};
t4250 = ct{1106};
t4251 = ct{1107};
t4252 = ct{1108};
t4253 = ct{1109};
t4254 = ct{1110};
t4255 = ct{1111};
t4256 = ct{1112};
t4257 = ct{1113};
t4259 = ct{1114};
t4260 = ct{1115};
t4261 = ct{1116};
t4262 = ct{1117};
t4263 = ct{1118};
t4264 = ct{1119};
t4266 = ct{1120};
t4267 = ct{1121};
t4268 = ct{1122};
t4274 = ct{1123};
t4275 = ct{1124};
t4277 = ct{1125};
t4278 = ct{1126};
t4279 = ct{1127};
t4280 = ct{1128};
t4281 = ct{1129};
t4285 = ct{1130};
t4286 = ct{1131};
t4287 = ct{1132};
t4288 = ct{1133};
t429 = ct{1134};
t4291 = ct{1135};
t4292 = ct{1136};
t4295 = ct{1137};
t4296 = ct{1138};
t4297 = ct{1139};
t4298 = ct{1140};
t4299 = ct{1141};
t43 = ct{1142};
t4304 = ct{1143};
t4306 = ct{1144};
t4307 = ct{1145};
t4308 = ct{1146};
t4310 = ct{1147};
t4311 = ct{1148};
t4313 = ct{1149};
t4314 = ct{1150};
t4321 = ct{1151};
t4322 = ct{1152};
t4323 = ct{1153};
t4324 = ct{1154};
t4326 = ct{1155};
t4353 = ct{1156};
t4354 = ct{1157};
t4355 = ct{1158};
t4356 = ct{1159};
t4357 = ct{1160};
t4359 = ct{1161};
t4362 = ct{1162};
t4363 = ct{1163};
t4367 = ct{1164};
t4369 = ct{1165};
t4370 = ct{1166};
t4373 = ct{1167};
t4374 = ct{1168};
t4375 = ct{1169};
t4376 = ct{1170};
t4377 = ct{1171};
t4378 = ct{1172};
t4379 = ct{1173};
t4381 = ct{1174};
t4382 = ct{1175};
t4383 = ct{1176};
t4385 = ct{1177};
t4386 = ct{1178};
t4387 = ct{1179};
t4388 = ct{1180};
t4390 = ct{1181};
t4395 = ct{1182};
t4396 = ct{1183};
t4400 = ct{1184};
t4402 = ct{1185};
t4403 = ct{1186};
t4404 = ct{1187};
t4405 = ct{1188};
t4406 = ct{1189};
t4407 = ct{1190};
t4409 = ct{1191};
t4410 = ct{1192};
t4411 = ct{1193};
t4412 = ct{1194};
t4413 = ct{1195};
t4415 = ct{1196};
t4421 = ct{1197};
t4424 = ct{1198};
t4427 = ct{1199};
t4428 = ct{1200};
t4429 = ct{1201};
t4430 = ct{1202};
t4431 = ct{1203};
t4432 = ct{1204};
t4434 = ct{1205};
t4435 = ct{1206};
t4436 = ct{1207};
t4437 = ct{1208};
t4438 = ct{1209};
t4439 = ct{1210};
t4440 = ct{1211};
t4441 = ct{1212};
t4442 = ct{1213};
t4443 = ct{1214};
t4444 = ct{1215};
t4447 = ct{1216};
t4453 = ct{1217};
t4458 = ct{1218};
t4460 = ct{1219};
t4461 = ct{1220};
t4464 = ct{1221};
t4470 = ct{1222};
t4473 = ct{1223};
t4474 = ct{1224};
t4475 = ct{1225};
t4480 = ct{1226};
t4481 = ct{1227};
t4483 = ct{1228};
t4484 = ct{1229};
t4486 = ct{1230};
t4487 = ct{1231};
t4488 = ct{1232};
t4489 = ct{1233};
t4491 = ct{1234};
t4492 = ct{1235};
t4496 = ct{1236};
t4498 = ct{1237};
t4499 = ct{1238};
t4500 = ct{1239};
t4501 = ct{1240};
t4502 = ct{1241};
t4504 = ct{1242};
t4507 = ct{1243};
t4508 = ct{1244};
t4510 = ct{1245};
t4511 = ct{1246};
t4513 = ct{1247};
t4514 = ct{1248};
t4515 = ct{1249};
t4516 = ct{1250};
t4517 = ct{1251};
t4520 = ct{1252};
t4521 = ct{1253};
t4522 = ct{1254};
t4525 = ct{1255};
t4526 = ct{1256};
t4528 = ct{1257};
t4530 = ct{1258};
t4531 = ct{1259};
t4532 = ct{1260};
t4533 = ct{1261};
t4535 = ct{1262};
t4536 = ct{1263};
t4539 = ct{1264};
t4542 = ct{1265};
t4543 = ct{1266};
t4545 = ct{1267};
t4546 = ct{1268};
t4549 = ct{1269};
t4550 = ct{1270};
t4551 = ct{1271};
t4552 = ct{1272};
t4555 = ct{1273};
t4560 = ct{1274};
t4562 = ct{1275};
t4563 = ct{1276};
t4571 = ct{1277};
t4572 = ct{1278};
t4574 = ct{1279};
t4579 = ct{1280};
t4581 = ct{1281};
t4582 = ct{1282};
t4583 = ct{1283};
t4584 = ct{1284};
t4585 = ct{1285};
t4586 = ct{1286};
t4587 = ct{1287};
t4588 = ct{1288};
t4589 = ct{1289};
t4591 = ct{1290};
t4593 = ct{1291};
t4594 = ct{1292};
t4595 = ct{1293};
t4597 = ct{1294};
t4599 = ct{1295};
t46 = ct{1296};
t4602 = ct{1297};
t4604 = ct{1298};
t4606 = ct{1299};
t4607 = ct{1300};
t4609 = ct{1301};
t4610 = ct{1302};
t4611 = ct{1303};
t4612 = ct{1304};
t4613 = ct{1305};
t4614 = ct{1306};
t4615 = ct{1307};
t4617 = ct{1308};
t4618 = ct{1309};
t4619 = ct{1310};
t4620 = ct{1311};
t4621 = ct{1312};
t4622 = ct{1313};
t4623 = ct{1314};
t4624 = ct{1315};
t4627 = ct{1316};
t4628 = ct{1317};
t4629 = ct{1318};
t4631 = ct{1319};
t4633 = ct{1320};
t4640 = ct{1321};
t4641 = ct{1322};
t4642 = ct{1323};
t4644 = ct{1324};
t4645 = ct{1325};
t4647 = ct{1326};
t4649 = ct{1327};
t4650 = ct{1328};
t4651 = ct{1329};
t4652 = ct{1330};
t4655 = ct{1331};
t4657 = ct{1332};
t4658 = ct{1333};
t4661 = ct{1334};
t4663 = ct{1335};
t4664 = ct{1336};
t4665 = ct{1337};
t4666 = ct{1338};
t4667 = ct{1339};
t4669 = ct{1340};
t4670 = ct{1341};
t4672 = ct{1342};
t4673 = ct{1343};
t4676 = ct{1344};
t4678 = ct{1345};
t4679 = ct{1346};
t4680 = ct{1347};
t4682 = ct{1348};
t4683 = ct{1349};
t4684 = ct{1350};
t4685 = ct{1351};
t4686 = ct{1352};
t4688 = ct{1353};
t4699 = ct{1354};
t47 = ct{1355};
t4702 = ct{1356};
t4703 = ct{1357};
t4704 = ct{1358};
t4705 = ct{1359};
t4706 = ct{1360};
t4708 = ct{1361};
t4709 = ct{1362};
t4710 = ct{1363};
t4711 = ct{1364};
t4716 = ct{1365};
t4718 = ct{1366};
t4719 = ct{1367};
t4720 = ct{1368};
t4721 = ct{1369};
t4723 = ct{1370};
t4725 = ct{1371};
t4726 = ct{1372};
t4727 = ct{1373};
t4728 = ct{1374};
t4729 = ct{1375};
t4732 = ct{1376};
t4733 = ct{1377};
t4734 = ct{1378};
t4735 = ct{1379};
t4736 = ct{1380};
t4737 = ct{1381};
t4738 = ct{1382};
t4740 = ct{1383};
t4741 = ct{1384};
t4742 = ct{1385};
t4744 = ct{1386};
t4746 = ct{1387};
t4749 = ct{1388};
t4756 = ct{1389};
t4758 = ct{1390};
t4759 = ct{1391};
t4760 = ct{1392};
t4762 = ct{1393};
t4764 = ct{1394};
t4768 = ct{1395};
t4769 = ct{1396};
t4770 = ct{1397};
t4772 = ct{1398};
t4777 = ct{1399};
t4780 = ct{1400};
t4785 = ct{1401};
t4786 = ct{1402};
t4787 = ct{1403};
t4788 = ct{1404};
t4789 = ct{1405};
t4790 = ct{1406};
t4791 = ct{1407};
t4792 = ct{1408};
t4795 = ct{1409};
t4798 = ct{1410};
t4799 = ct{1411};
t4800 = ct{1412};
t4801 = ct{1413};
t4805 = ct{1414};
t4809 = ct{1415};
t4814 = ct{1416};
t4816 = ct{1417};
t4817 = ct{1418};
t4818 = ct{1419};
t4819 = ct{1420};
t4822 = ct{1421};
t4823 = ct{1422};
t4824 = ct{1423};
t4826 = ct{1424};
t4828 = ct{1425};
t4829 = ct{1426};
t4832 = ct{1427};
t4833 = ct{1428};
t4836 = ct{1429};
t4839 = ct{1430};
t4840 = ct{1431};
t4842 = ct{1432};
t4843 = ct{1433};
t4845 = ct{1434};
t4846 = ct{1435};
t4847 = ct{1436};
t4849 = ct{1437};
t4852 = ct{1438};
t4856 = ct{1439};
t4857 = ct{1440};
t4860 = ct{1441};
t4863 = ct{1442};
t4864 = ct{1443};
t4865 = ct{1444};
t4866 = ct{1445};
t4867 = ct{1446};
t4868 = ct{1447};
t4869 = ct{1448};
t4870 = ct{1449};
t4871 = ct{1450};
t4872 = ct{1451};
t4873 = ct{1452};
t4874 = ct{1453};
t4875 = ct{1454};
t4876 = ct{1455};
t4877 = ct{1456};
t4880 = ct{1457};
t4881 = ct{1458};
t4882 = ct{1459};
t4883 = ct{1460};
t4884 = ct{1461};
t4885 = ct{1462};
t4886 = ct{1463};
t4887 = ct{1464};
t4888 = ct{1465};
t4890 = ct{1466};
t4892 = ct{1467};
t4893 = ct{1468};
t4894 = ct{1469};
t4897 = ct{1470};
t4898 = ct{1471};
t4899 = ct{1472};
t4900 = ct{1473};
t4902 = ct{1474};
t4905 = ct{1475};
t4911 = ct{1476};
t4917 = ct{1477};
t4921 = ct{1478};
t4922 = ct{1479};
t4925 = ct{1480};
t4927 = ct{1481};
t4931 = ct{1482};
t4950 = ct{1483};
t4952 = ct{1484};
t4953 = ct{1485};
t4954 = ct{1486};
t4961 = ct{1487};
t4962 = ct{1488};
t4963 = ct{1489};
t4965 = ct{1490};
t4968 = ct{1491};
t4969 = ct{1492};
t4973 = ct{1493};
t4974 = ct{1494};
t4975 = ct{1495};
t4976 = ct{1496};
t4977 = ct{1497};
t4982 = ct{1498};
t4983 = ct{1499};
t4984 = ct{1500};
t4985 = ct{1501};
t4986 = ct{1502};
t4987 = ct{1503};
t4992 = ct{1504};
t4994 = ct{1505};
t4995 = ct{1506};
t4996 = ct{1507};
t4998 = ct{1508};
t5 = ct{1509};
t50 = ct{1510};
t5000 = ct{1511};
t5001 = ct{1512};
t5002 = ct{1513};
t5005 = ct{1514};
t5007 = ct{1515};
t5010 = ct{1516};
t5012 = ct{1517};
t5013 = ct{1518};
t5014 = ct{1519};
t5015 = ct{1520};
t5017 = ct{1521};
t5021 = ct{1522};
t5022 = ct{1523};
t5023 = ct{1524};
t5025 = ct{1525};
t5026 = ct{1526};
t5027 = ct{1527};
t5028 = ct{1528};
t5030 = ct{1529};
t5031 = ct{1530};
t5032 = ct{1531};
t5033 = ct{1532};
t5034 = ct{1533};
t5035 = ct{1534};
t5036 = ct{1535};
t5038 = ct{1536};
t5039 = ct{1537};
t5040 = ct{1538};
t5041 = ct{1539};
t5042 = ct{1540};
t5047 = ct{1541};
t5048 = ct{1542};
t5049 = ct{1543};
t5051 = ct{1544};
t5052 = ct{1545};
t5053 = ct{1546};
t5054 = ct{1547};
t5056 = ct{1548};
t5058 = ct{1549};
t5061 = ct{1550};
t5063 = ct{1551};
t5064 = ct{1552};
t5067 = ct{1553};
t5068 = ct{1554};
t5069 = ct{1555};
t5073 = ct{1556};
t5074 = ct{1557};
t5076 = ct{1558};
t5077 = ct{1559};
t5091 = ct{1560};
t5092 = ct{1561};
t5094 = ct{1562};
t5096 = ct{1563};
t5105 = ct{1564};
t5108 = ct{1565};
t5111 = ct{1566};
t5113 = ct{1567};
t5114 = ct{1568};
t5115 = ct{1569};
t5116 = ct{1570};
t5118 = ct{1571};
t5119 = ct{1572};
t5121 = ct{1573};
t5123 = ct{1574};
t5124 = ct{1575};
t5126 = ct{1576};
t5127 = ct{1577};
t5128 = ct{1578};
t5130 = ct{1579};
t5131 = ct{1580};
t5144 = ct{1581};
t5145 = ct{1582};
t5146 = ct{1583};
t5147 = ct{1584};
t5148 = ct{1585};
t5149 = ct{1586};
t5150 = ct{1587};
t5151 = ct{1588};
t5152 = ct{1589};
t5153 = ct{1590};
t5155 = ct{1591};
t5158 = ct{1592};
t5162 = ct{1593};
t5164 = ct{1594};
t5165 = ct{1595};
t5169 = ct{1596};
t5184 = ct{1597};
t5189 = ct{1598};
t5190 = ct{1599};
t5191 = ct{1600};
t5192 = ct{1601};
t5193 = ct{1602};
t5195 = ct{1603};
t5196 = ct{1604};
t5198 = ct{1605};
t5201 = ct{1606};
t5202 = ct{1607};
t5203 = ct{1608};
t5204 = ct{1609};
t5206 = ct{1610};
t5207 = ct{1611};
t5208 = ct{1612};
t5209 = ct{1613};
t5210 = ct{1614};
t5211 = ct{1615};
t5212 = ct{1616};
t5213 = ct{1617};
t5214 = ct{1618};
t5216 = ct{1619};
t5217 = ct{1620};
t5218 = ct{1621};
t5219 = ct{1622};
t5221 = ct{1623};
t5222 = ct{1624};
t5223 = ct{1625};
t5224 = ct{1626};
t5225 = ct{1627};
t5226 = ct{1628};
t5227 = ct{1629};
t5228 = ct{1630};
t5229 = ct{1631};
t5230 = ct{1632};
t5231 = ct{1633};
t5232 = ct{1634};
t5233 = ct{1635};
t5234 = ct{1636};
t5235 = ct{1637};
t5236 = ct{1638};
t5237 = ct{1639};
t5238 = ct{1640};
t5239 = ct{1641};
t5240 = ct{1642};
t5241 = ct{1643};
t5242 = ct{1644};
t5243 = ct{1645};
t5244 = ct{1646};
t5245 = ct{1647};
t5246 = ct{1648};
t5247 = ct{1649};
t5248 = ct{1650};
t5249 = ct{1651};
t5250 = ct{1652};
t5252 = ct{1653};
t5254 = ct{1654};
t5255 = ct{1655};
t5257 = ct{1656};
t5260 = ct{1657};
t5261 = ct{1658};
t5263 = ct{1659};
t5265 = ct{1660};
t5266 = ct{1661};
t5267 = ct{1662};
t5269 = ct{1663};
t5270 = ct{1664};
t5272 = ct{1665};
t5273 = ct{1666};
t5274 = ct{1667};
t5275 = ct{1668};
t5276 = ct{1669};
t5277 = ct{1670};
t5281 = ct{1671};
t5282 = ct{1672};
t5285 = ct{1673};
t5288 = ct{1674};
t5289 = ct{1675};
t5290 = ct{1676};
t5291 = ct{1677};
t5293 = ct{1678};
t5295 = ct{1679};
t5298 = ct{1680};
t5299 = ct{1681};
t5301 = ct{1682};
t5302 = ct{1683};
t5303 = ct{1684};
t5304 = ct{1685};
t5306 = ct{1686};
t5307 = ct{1687};
t5308 = ct{1688};
t5316 = ct{1689};
t5317 = ct{1690};
t5320 = ct{1691};
t5322 = ct{1692};
t5325 = ct{1693};
t5328 = ct{1694};
t5330 = ct{1695};
t5331 = ct{1696};
t5332 = ct{1697};
t5335 = ct{1698};
t5337 = ct{1699};
t5338 = ct{1700};
t5339 = ct{1701};
t5340 = ct{1702};
t5342 = ct{1703};
t5344 = ct{1704};
t5345 = ct{1705};
t5346 = ct{1706};
t5347 = ct{1707};
t5348 = ct{1708};
t5349 = ct{1709};
t5350 = ct{1710};
t5356 = ct{1711};
t5357 = ct{1712};
t5358 = ct{1713};
t5361 = ct{1714};
t5362 = ct{1715};
t5365 = ct{1716};
t5369 = ct{1717};
t5370 = ct{1718};
t5377 = ct{1719};
t5379 = ct{1720};
t5380 = ct{1721};
t5381 = ct{1722};
t5383 = ct{1723};
t5384 = ct{1724};
t5385 = ct{1725};
t5386 = ct{1726};
t5387 = ct{1727};
t5388 = ct{1728};
t5389 = ct{1729};
t5390 = ct{1730};
t5391 = ct{1731};
t5392 = ct{1732};
t5393 = ct{1733};
t5395 = ct{1734};
t5396 = ct{1735};
t5399 = ct{1736};
t5402 = ct{1737};
t5403 = ct{1738};
t5405 = ct{1739};
t5407 = ct{1740};
t5408 = ct{1741};
t5409 = ct{1742};
t5411 = ct{1743};
t5412 = ct{1744};
t5418 = ct{1745};
t5420 = ct{1746};
t5427 = ct{1747};
t5428 = ct{1748};
t5433 = ct{1749};
t5434 = ct{1750};
t5440 = ct{1751};
t5441 = ct{1752};
t5443 = ct{1753};
t5444 = ct{1754};
t5445 = ct{1755};
t5446 = ct{1756};
t5449 = ct{1757};
t5455 = ct{1758};
t5458 = ct{1759};
t5461 = ct{1760};
t5462 = ct{1761};
t5465 = ct{1762};
t5480 = ct{1763};
t5481 = ct{1764};
t5482 = ct{1765};
t5483 = ct{1766};
t5484 = ct{1767};
t5485 = ct{1768};
t5486 = ct{1769};
t5487 = ct{1770};
t5488 = ct{1771};
t5489 = ct{1772};
t5490 = ct{1773};
t5491 = ct{1774};
t5492 = ct{1775};
t5493 = ct{1776};
t5494 = ct{1777};
t5496 = ct{1778};
t5498 = ct{1779};
t5499 = ct{1780};
t5500 = ct{1781};
t5504 = ct{1782};
t5505 = ct{1783};
t5509 = ct{1784};
t5510 = ct{1785};
t5514 = ct{1786};
t5515 = ct{1787};
t5516 = ct{1788};
t5517 = ct{1789};
t5518 = ct{1790};
t5522 = ct{1791};
t5523 = ct{1792};
t5524 = ct{1793};
t5525 = ct{1794};
t5531 = ct{1795};
t5535 = ct{1796};
t5536 = ct{1797};
t5537 = ct{1798};
t5540 = ct{1799};
t5544 = ct{1800};
t5547 = ct{1801};
t5550 = ct{1802};
t5552 = ct{1803};
t5553 = ct{1804};
t5554 = ct{1805};
t5556 = ct{1806};
t5557 = ct{1807};
t5565 = ct{1808};
t5566 = ct{1809};
t5571 = ct{1810};
t5578 = ct{1811};
t5580 = ct{1812};
t5595 = ct{1813};
t56 = ct{1814};
t5601 = ct{1815};
t5603 = ct{1816};
t5605 = ct{1817};
t5619 = ct{1818};
t5620 = ct{1819};
t5626 = ct{1820};
t5627 = ct{1821};
t5631 = ct{1822};
t5639 = ct{1823};
t5640 = ct{1824};
t5646 = ct{1825};
t5661 = ct{1826};
t5662 = ct{1827};
t5663 = ct{1828};
t5670 = ct{1829};
t5671 = ct{1830};
t5674 = ct{1831};
t5675 = ct{1832};
t5677 = ct{1833};
t5678 = ct{1834};
t5679 = ct{1835};
t5681 = ct{1836};
t5682 = ct{1837};
t5684 = ct{1838};
t5694 = ct{1839};
t5695 = ct{1840};
t5699 = ct{1841};
t5700 = ct{1842};
t5701 = ct{1843};
t5702 = ct{1844};
t5703 = ct{1845};
t5709 = ct{1846};
t5717 = ct{1847};
t5718 = ct{1848};
t5720 = ct{1849};
t5721 = ct{1850};
t5722 = ct{1851};
t5723 = ct{1852};
t5724 = ct{1853};
t5730 = ct{1854};
t5734 = ct{1855};
t5750 = ct{1856};
t5760 = ct{1857};
t5764 = ct{1858};
t5769 = ct{1859};
t5791 = ct{1860};
t5792 = ct{1861};
t5794 = ct{1862};
t58 = ct{1863};
t5832 = ct{1864};
t5835 = ct{1865};
t5839 = ct{1866};
t5840 = ct{1867};
t5846 = ct{1868};
t5852 = ct{1869};
t5853 = ct{1870};
t5857 = ct{1871};
t5864 = ct{1872};
t5866 = ct{1873};
t5871 = ct{1874};
t5876 = ct{1875};
t5879 = ct{1876};
t5890 = ct{1877};
t5891 = ct{1878};
t59 = ct{1879};
t5900 = ct{1880};
t5909 = ct{1881};
t5911 = ct{1882};
t5930 = ct{1883};
t5932 = ct{1884};
t5941 = ct{1885};
t5943 = ct{1886};
t5944 = ct{1887};
t5951 = ct{1888};
t5953 = ct{1889};
t5954 = ct{1890};
t5977 = ct{1891};
t5992 = ct{1892};
t5994 = ct{1893};
t5995 = ct{1894};
t6 = ct{1895};
t60 = ct{1896};
t6004 = ct{1897};
t6017 = ct{1898};
t6018 = ct{1899};
t6020 = ct{1900};
t6057 = ct{1901};
t6058 = ct{1902};
t6065 = ct{1903};
t6075 = ct{1904};
t6095 = ct{1905};
t6135 = ct{1906};
t6151 = ct{1907};
t6153 = ct{1908};
t6183 = ct{1909};
t6184 = ct{1910};
t6185 = ct{1911};
t6199 = ct{1912};
t6206 = ct{1913};
t6207 = ct{1914};
t6209 = ct{1915};
t6219 = ct{1916};
t6221 = ct{1917};
t6247 = ct{1918};
t6253 = ct{1919};
t628 = ct{1920};
t6317 = ct{1921};
t6321 = ct{1922};
t6323 = ct{1923};
t6339 = ct{1924};
t6341 = ct{1925};
t6367 = ct{1926};
t6375 = ct{1927};
t638 = ct{1928};
t640 = ct{1929};
t6405 = ct{1930};
t642 = ct{1931};
t643 = ct{1932};
t6450 = ct{1933};
t6484 = ct{1934};
t6485 = ct{1935};
t6486 = ct{1936};
t649 = ct{1937};
t6493 = ct{1938};
t6507 = ct{1939};
t6508 = ct{1940};
t6511 = ct{1941};
t6515 = ct{1942};
t6516 = ct{1943};
t654 = ct{1944};
t6543 = ct{1945};
t6544 = ct{1946};
t655 = ct{1947};
t656 = ct{1948};
t6565 = ct{1949};
t657 = ct{1950};
t659 = ct{1951};
t660 = ct{1952};
t665 = ct{1953};
t6658 = ct{1954};
t6663 = ct{1955};
t667 = ct{1956};
t668 = ct{1957};
t6689 = ct{1958};
t669 = ct{1959};
t6691 = ct{1960};
t6692 = ct{1961};
t67 = ct{1962};
t670 = ct{1963};
t672 = ct{1964};
t673 = ct{1965};
t674 = ct{1966};
t675 = ct{1967};
t676 = ct{1968};
t677 = ct{1969};
t68 = ct{1970};
t681 = ct{1971};
t6811 = ct{1972};
t6812 = ct{1973};
t6813 = ct{1974};
t682 = ct{1975};
t684 = ct{1976};
t685 = ct{1977};
t686 = ct{1978};
t6861 = ct{1979};
t687 = ct{1980};
t6892 = ct{1981};
t6893 = ct{1982};
t691 = ct{1983};
t6916 = ct{1984};
t692 = ct{1985};
t693 = ct{1986};
t694 = ct{1987};
t6980 = ct{1988};
t6981 = ct{1989};
t7 = ct{1990};
t70 = ct{1991};
t702 = ct{1992};
t7029 = ct{1993};
t7039 = ct{1994};
t7041 = ct{1995};
t7043 = ct{1996};
t7051 = ct{1997};
t7064 = ct{1998};
t707 = ct{1999};
t708 = ct{2000};
t71 = ct{2001};
t710 = ct{2002};
t715 = ct{2003};
t716 = ct{2004};
t717 = ct{2005};
t718 = ct{2006};
t7204 = ct{2007};
t721 = ct{2008};
t7219 = ct{2009};
t722 = ct{2010};
t7227 = ct{2011};
t7228 = ct{2012};
t7229 = ct{2013};
t7230 = ct{2014};
t724 = ct{2015};
t725 = ct{2016};
t73 = ct{2017};
t736 = ct{2018};
t738 = ct{2019};
t740 = ct{2020};
t741 = ct{2021};
t749 = ct{2022};
t756 = ct{2023};
t76 = ct{2024};
t762 = ct{2025};
t768 = ct{2026};
t777 = ct{2027};
t792 = ct{2028};
t793 = ct{2029};
t801 = ct{2030};
t802 = ct{2031};
t808 = ct{2032};
t813 = ct{2033};
t819 = ct{2034};
t821 = ct{2035};
t850 = ct{2036};
t855 = ct{2037};
t874 = ct{2038};
t878 = ct{2039};
t89 = ct{2040};
t90 = ct{2041};
t91 = ct{2042};
t92 = ct{2043};
t941 = ct{2044};
t944 = ct{2045};
t948 = ct{2046};
t951 = ct{2047};
t97 = ct{2048};
t5448 = t5263.*(t1896-t3232).*(-9.0e-8);
t5451 = t5263.*(t1896-t3232).*9.0e-8;
t5452 = -t5449;
t5454 = t4865.*(t3951+t18.*(t1861-t3214)).*(-9.3e-7);
t5457 = -t5455;
t5459 = t4865.*(t3951+t18.*(t1861-t3214)).*(-9.0e-8);
t5467 = t3524.*t5290;
t5468 = t3524.*t5291;
t5469 = -t5291.*(t1896-t3232);
t5470 = t3528.*t5291;
t5471 = t3531.*t5290;
t5472 = t3531.*t5291;
t5475 = -t5298.*(t1896-t3232);
t5476 = t3528.*t5298;
t5477 = t5298.*(t1896-t3232);
t5532 = t4324.*t5150;
t5534 = t4324.*t5151;
t5538 = t4326.*t5155;
t5539 = t1207+t1208+t1221+t1235+t2149+t2150+t2151+t2168+t2744+t3389+t3392+t3408+t3696+t3698;
t5541 = t5263.*(t2694-t2701+t3036-t3043).*(-1.02e-6);
t5542 = t5263.*(t2694-t2701+t3036-t3043).*1.02e-6;
t5543 = t5263.*(t2694-t2701+t3036-t3043).*(-9.0e-8);
t5545 = t5263.*(t2694-t2701+t3036-t3043).*9.0e-8;
t5546 = -t5544;
t5551 = -t5547;
t5555 = t3741+t3830+t3837+t3841+t3906;
t5558 = t3359.*t5150.*(t2694-t2701+t3036-t3043).*(-2.889644e-2);
t5559 = t3359.*t5150.*(t2694-t2701+t3036-t3043).*2.889644e-2;
t5560 = t3359.*t5151.*(t2694-t2701+t3036-t3043).*(-2.889644e-2);
t5561 = t3359.*t5151.*(t2694-t2701+t3036-t3043).*2.889644e-2;
t5562 = t5263.*(t3235-t3535).*(-1.02e-6);
t5564 = t5263.*(t3235-t3535).*1.02e-6;
t5567 = t5263.*(t3235-t3535).*(-9.0e-8);
t5569 = -t5565;
t5570 = t5263.*(t3235-t3535).*9.0e-8;
t5572 = t3359.*t3901.*t5155.*2.889644e-2;
t5573 = -t5571;
t5574 = t3992.*t5265.*9.3e-7;
t5576 = t3992.*t5266.*1.02e-6;
t5577 = t3992.*t5265.*9.0e-8;
t5579 = t3992.*t5266.*9.0e-8;
t5581 = -t5299.*(t3235-t3535);
t5582 = t3992.*t5299;
t5592 = t4175.*t4886.*(t2694-t2701+t3036-t3043).*(-1.08769e-2);
t5593 = t4175.*t4886.*(t2694-t2701+t3036-t3043).*1.08769e-2;
t5597 = -t5595;
t5598 = t5291.*(t3908-(t262.*(t46-t47))./9.007199254740992e+15);
t5599 = t4111.*t5291;
t5602 = -t5601;
t5606 = (t4133-t4843).*(t2813-t2835+t18.*(t1456-t2355).*1.02e-6+t23.*(t1456-t2355).*9.0e-8);
t5607 = t2298+t3293+t3570+t3580+t3581+t3595+t3598+t3607;
t5616 = t3323+t3343+t3629+t3637+t4078+t4079;
t5617 = t3628.*t3901.*t5150.*2.889644e-2;
t5621 = -t4134.*t4973.*(t2674-t2676+t3022-t3027);
t5622 = t4134.*t4973.*(t2674-t2676+t3022-t3027);
t5637 = t2397+t3338+t3618+t3626+t3627+t3645+t3647+t3648;
t5638 = t2369+t2423+t3331+t3351+t3561+t3618+t3626+t3647+t3648;
t5658 = t4277.*t5303;
t5660 = t4277.*t5304;
t5664 = t4278.*t5307;
t5666 = t201.*t5640.*8.595599785252598e-1;
t5676 = t50.*t202.*t5640.*9.543032792050485e-17;
t5685 = t3209.*t5540;
t5688 = t2363.*t5639;
t5689 = t2388.*t5639;
t5691 = t2419.*t5639;
t5705 = -t3313.*t5303.*(t2674-t2676+t3022-t3027);
t5706 = t3313.*t5303.*(t2674-t2676+t3022-t3027);
t5707 = -t3313.*t5304.*(t2674-t2676+t3022-t3027);
t5708 = t3313.*t5304.*(t2674-t2676+t3022-t3027);
t5711 = t3313.*t3877.*t5307;
t5725 = -t5724;
t5727 = -t3480.*t5303.*(t2674-t2676+t3022-t3027);
t5728 = -t3480.*t5304.*(t2674-t2676+t3022-t3027);
t5731 = t3480.*t3877.*t5307;
t5732 = t3617.*t3877.*t5303;
t5735 = -t5734;
t5736 = t3051+t3073+t3978+t3983+t4028+t4059;
t5737 = t4355+t5325;
t5751 = t3229.*t5640;
t5752 = t3230.*t5640;
t5754 = t3085+t3086+t4054+t4058+t4061+t4069;
t5755 = t4197+t4619+t4673;
t5759 = -t2363.*(t3067+t3982-t4028+t4053+(t17.*t3229.*(t1861-t3214))./1.0e+8-t17.*t50.*t202.*t2297.*9.543032792050485e-25);
t5761 = t2363.*(t3067+t3982-t4028+t4053+(t17.*t3229.*(t1861-t3214))./1.0e+8-t17.*t50.*t202.*t2297.*9.543032792050485e-25);
t5765 = t3524.*t5639;
t5766 = -t5639.*(t1896-t3232);
t5767 = t3528.*t5639;
t5768 = t3531.*t5639;
t5770 = -t5769;
t5775 = -t5540.*(t2674-t2676+t3022-t3027);
t5779 = t5540.*(t2674-t2676+t3022-t3027);
t5785 = t50.*t189.*t5764.*9.543032792050485e-17;
t5793 = t2297.*t5764;
t5795 = -t5794;
t5804 = (t1896-t3232).*(t3067+t3982-t4028+t4053+(t17.*t3229.*(t1861-t3214))./1.0e+8-t17.*t50.*t202.*t2297.*9.543032792050485e-25);
t5805 = -t3528.*(t3067+t3982-t4028+t4053+(t17.*t3229.*(t1861-t3214))./1.0e+8-t17.*t50.*t202.*t2297.*9.543032792050485e-25);
t5806 = t3904.*t5640;
t5807 = -t5640.*(t1959-t3306+t38.*t1022.*(t855-t878).*2.196325630278387e-1);
t5826 = t4113.*t5639;
t5827 = -t5639.*(t1005+t26.*(t1941-t3308+t39.*t1022.*(t855-t878).*2.196325630278387e-1));
t5828 = t5639.*(t1005+t26.*(t1941-t3308+t39.*t1022.*(t855-t878).*2.196325630278387e-1));
t5855 = -t5150.*(t1196+t1212+t1237+t1238+t2139+t2140+t2159+t2165+t2754+t2814+t2953+t3072+t3405+t3412);
t5859 = -t5151.*(t1196+t1212+t1237+t1238+t2139+t2140+t2159+t2165+t2754+t2814+t2953+t3072+t3405+t3412);
t5860 = t5155.*t5249;
t5861 = t5151.*(t1196+t1212+t1237+t1238+t2139+t2140+t2159+t2165+t2754+t2814+t2953+t3072+t3405+t3412);
t5868 = -t5303.*(t649+t670+t686+t687+t1577+t1578+t1586+t1600+t2303+t2339+t2689+t3030+t3292+t3305);
t5894 = -t3689.*t3877.*(t350+t366-t1205+t1210-t1217-t1218-t2147+t2152+t2154+t2155-t3395-t3399-t3409-t3716+t3723+t32.*t50.*t202.*(t46-t47).*8.687615694748404e-39);
t5896 = t3689.*t3877.*(t350+t366-t1205+t1210-t1217-t1218-t2147+t2152+t2154+t2155-t3395-t3399-t3409-t3716+t3723+t32.*t50.*t202.*(t46-t47).*8.687615694748404e-39);
t5907 = t3617.*t4822.*t5303;
t5908 = t3617.*t4822.*t5304;
t5910 = -t5909;
t5912 = -t5151.*(-t321+t332+t1196+t1212+t1237+t1238+t2139+t2140+t2159+t2165+t2754+t2814+t2953+t3072+t3405+t3412);
t5913 = t5155.*t5303;
et138 = -t2306-t2317+t3144+t3147+t35.*t941.*t948.*(t850-t874).*3.775747223193135e-1;
et139 = t36.*t941.*t948.*(t850-t874).*2.244797987218524e-1;
t5914 = -t3617.*t5307.*(et138+et139);
t5921 = -t3782.*t3877.*(t350+t366-t1205+t1210-t1217-t1218-t2147+t2152+t2154+t2155-t3395-t3399-t3409-t3716+t3723+t32.*t50.*t202.*(t46-t47).*8.687615694748404e-39);
t5922 = t3782.*t3877.*(t350+t366-t1205+t1210-t1217-t1218-t2147+t2152+t2154+t2155-t3395-t3399-t3409-t3716+t3723+t32.*t50.*t202.*(t46-t47).*8.687615694748404e-39);
t5958 = t201.*t5944.*8.595599785252598e-1;
t5965 = -t3877.*t3891.*(t350+t366-t1205+t1210-t1217-t1218-t2147+t2152+t2154+t2155-t3395-t3399-t3409-t3716+t3723+t32.*t50.*t202.*(t46-t47).*8.687615694748404e-39);
t5966 = t3877.*t3891.*(t350+t366-t1205+t1210-t1217-t1218-t2147+t2152+t2154+t2155-t3395-t3399-t3409-t3716+t3723+t32.*t50.*t202.*(t46-t47).*8.687615694748404e-39);
t5969 = t2388.*t5943;
t5970 = t2419.*t5943;
t5974 = t4441+t4443+t4453+t4470;
t5975 = t4665+t5646;
t5984 = t4480+t4484+t4486+t4488;
t5998 = t3229.*t5944;
t5999 = t3230.*t5944;
t6002 = t4684+t5684;
t6006 = t4764+t5677;
t6009 = t50.*t189.*t5995.*9.543032792050485e-17;
t6011 = t3524.*t5943;
t6012 = -t5943.*(t1896-t3232);
t6014 = t3528.*t5943;
t6016 = t3531.*t5943;
t6019 = t2297.*t5995;
t6021 = -t6020;
t6027 = t3805+t3838+t3868+t4286+t4299+t4367;
t6028 = t50.*t189.*t6018.*9.543032792050485e-17;
t6030 = t3047.*t5995;
t6032 = t2297.*t6018;
t6054 = t3047.*t6018;
t6059 = t3904.*t5944;
t6060 = -t5944.*(t1959-t3306+t38.*t1022.*(t855-t878).*2.196325630278387e-1);
et140 = -t2125-t2142+t2745-t2750+t2774+t2785+t2786-t3457+t4002+t32.*(t1941-t3308+t39.*t1022.*(t855-t878).*2.196325630278387e-1).*1.869599668e-7;
et141 = t38.*t1022.*(t855-t878).*1.46680315462752e-4;
t6061 = -t5150.*(et140+et141);
et142 = -t2125-t2142+t2745-t2750+t2774+t2785+t2786-t3457+t4002+t32.*(t1941-t3308+t39.*t1022.*(t855-t878).*2.196325630278387e-1).*1.869599668e-7;
et143 = t38.*t1022.*(t855-t878).*1.46680315462752e-4;
t6062 = t5150.*(et142+et143);
et144 = -t2125-t2142+t2745-t2750+t2774+t2785+t2786-t3457+t4002+t32.*(t1941-t3308+t39.*t1022.*(t855-t878).*2.196325630278387e-1).*1.869599668e-7;
et145 = t38.*t1022.*(t855-t878).*1.46680315462752e-4;
t6063 = -t5151.*(et144+et145);
et146 = -t2125-t2142+t2745-t2750+t2774+t2785+t2786-t3457+t4002+t32.*(t1941-t3308+t39.*t1022.*(t855-t878).*2.196325630278387e-1).*1.869599668e-7;
et147 = t38.*t1022.*(t855-t878).*1.46680315462752e-4;
t6064 = t5151.*(et146+et147);
t6066 = -t6065;
et148 = -t2748-t2749+t2773+t2781-t2788+t3204+t3458+t3997-t4009+t262.*(t46-t47).*2.075672598245148e-23;
et149 = t264.*(t46-t47).*1.875105520197095e-20;
t6067 = -t5155.*(et148+et149);
t6085 = t4113.*t5943;
t6086 = -t5943.*(t1005+t26.*(t1941-t3308+t39.*t1022.*(t855-t878).*2.196325630278387e-1));
t6087 = t5943.*(t1005+t26.*(t1941-t3308+t39.*t1022.*(t855-t878).*2.196325630278387e-1));
t6091 = t5303.*t5509;
t6092 = t5304.*t5509;
t6096 = t5307.*t5510;
t6097 = t3050+t3087+t3088+t3977+t3981+t4060+t4063+t4065+t4070;
t6112 = -t5223.*(t350+t366-t1205+t1210-t1217-t1218-t2147+t2152+t2154+t2155-t3395-t3399-t3409-t3716+t3723+t32.*t50.*t202.*(t46-t47).*8.687615694748404e-39);
t6128 = t3659+t3662+t4402+t4403+t4430+t4431;
et150 = -t2306-t2317+t3144+t3147+t35.*t941.*t948.*(t850-t874).*3.775747223193135e-1;
et151 = t36.*t941.*t948.*(t850-t874).*2.244797987218524e-1;
t6143 = t4134.*(et150+et151).*(t350+t366-t1205+t1210-t1217-t1218-t2147+t2152+t2154+t2155-t3395-t3399-t3409-t3716+t3723+t32.*t50.*t202.*(t46-t47).*8.687615694748404e-39);
t6306 = t3953+t4196+t4288+t4353+t4407+t4585;
t6322 = -t6321;
t6356 = t4973.*t5951;
t6366 = t3877.*t4134.*t5992;
t6387 = -t3209.*(t3856+t4618-t4670+t3789.*(t3235-t3535)+t3793.*(t3235-t3535));
t6388 = t3209.*(t3856+t4618-t4670+t3789.*(t3235-t3535)+t3793.*(t3235-t3535));
t6406 = -t6405;
t6414 = (t1861-t3214).*(t3856+t4618-t4670+t3789.*(t3235-t3535)+t3793.*(t3235-t3535));
t6442 = -t5723.*(t350+t366-t1205+t1210-t1217-t1218-t2147+t2152+t2154+t2155-t3395-t3399-t3409-t3716+t3723+t32.*t50.*t202.*(t46-t47).*8.687615694748404e-39);
t6451 = -t6450;
t6453 = (t2674-t2676+t3022-t3027).*(t3856+t4618-t4670+t3789.*(t3235-t3535)+t3793.*(t3235-t3535));
t6506 = t4435+t4442+t4483+t4487+t4489+t4492;
t6514 = t2320+t2378+t2510+t2534+t2978+t2979+t3893+t4106+t4152+t4155+t4805+t4809;
t6520 = t4886.*t6183;
t6529 = t2388.*t6516;
t6575 = t3524.*t6516;
t6576 = t3531.*t6516;
et152 = t1554+t2361+t2362+t2367+t2414+t3928+t3934+t4160+t4163+t17.*(-t1901+t3122+t3270).*5.68686e-3;
et153 = t350+t366-t1205+t1210-t1217-t1218-t2147+t2152+t2154+t2155-t3395-t3399-t3409-t3716+t3723+t32.*t50.*t202.*(t46-t47).*8.687615694748404e-39;
t6593 = et152.*et153;
t6611 = -t5954.*(t350+t366-t1205+t1210-t1217-t1218-t2147+t2152+t2154+t2155-t3395-t3399-t3409-t3716+t3723+t32.*t50.*t202.*(t46-t47).*8.687615694748404e-39);
t6612 = t5954.*(t350+t366-t1205+t1210-t1217-t1218-t2147+t2152+t2154+t2155-t3395-t3399-t3409-t3716+t3723+t32.*t50.*t202.*(t46-t47).*8.687615694748404e-39);
t6853 = t4166+t4574+t4595+t4658+t5189+t5207;
t6860 = (t2694-t2701+t3036-t3043).*(t1513+t1879+t2598+t2820+t2834+t3117+t3118).*(-t2308+t2378+t2510-t2530-t2975+t2979+t3893+t4106+t4152+t4155+t4805+t4809).*7.26735e-3;
t6913 = t3209.*(t4595+t4658+t5189+t5207-t3468.*(t1005+t26.*(t1941-t3308+t39.*t1022.*(t855-t878).*2.196325630278387e-1))-t3420.*(t1896-t3232));
et154 = t707+t708-t721-t722-t749+t762+t768-t777-t792-t793-t801-t802-t808+t813-t819+t821-t1629+t1637-t1640-t1641-t1659-t1661+t1666+t1667+t1683+t1692+t1705-t1712+t1758+t1759+t1775+t1776+t1973+t1993+t1994+t2023+t2053+t2060-t2089-t2090+t2098+t2099-t14.*t15.*t21.*t50.*t189.*3.670836568391568e-22;
et155 = t16.*t19.*t20.*t50.*t189.*(-3.279367663374749e-19)-t14.*t15.*t17.*t21.*t50.*t189.*7.075931802640439e-19;
et156 = t14.*t17.*t20.*t21.*t50.*t189.*(-1.190170786299927e-18)-t15.*t17.*t19.*t21.*t50.*t189.*1.190170786299927e-18;
et157 = t19.*t20.*t21.*t22.*t50.*t189.*(-3.226512155691387e-19);
t6915 = -t5992.*(et154+et155+et156+et157);
et158 = t707+t708-t721-t722-t749+t762+t768-t777-t792-t793-t801-t802-t808+t813-t819+t821-t1629+t1637-t1640-t1641-t1659-t1661+t1666+t1667+t1683+t1692+t1705-t1712+t1758+t1759+t1775+t1776+t1973+t1993+t1994+t2023+t2053+t2060-t2089-t2090+t2098+t2099-t14.*t15.*t21.*t50.*t189.*3.670836568391568e-22;
et159 = t16.*t19.*t20.*t50.*t189.*(-3.279367663374749e-19)-t14.*t15.*t17.*t21.*t50.*t189.*7.075931802640439e-19;
et160 = t14.*t17.*t20.*t21.*t50.*t189.*(-1.190170786299927e-18)-t15.*t17.*t19.*t21.*t50.*t189.*1.190170786299927e-18;
et161 = t19.*t20.*t21.*t22.*t50.*t189.*(-3.226512155691387e-19);
t6917 = t5992.*(et158+et159+et160+et161);
t6922 = t6565.*(t2674-t2676+t3022-t3027).*(t1488+t1874+t2519+t2740+t2747+t3096+t3097);
t6937 = -(t1861-t3214).*(t4595+t4658+t5189+t5207-t3468.*(t1005+t26.*(t1941-t3308+t39.*t1022.*(t855-t878).*2.196325630278387e-1))-t3420.*(t1896-t3232));
t6978 = -(t2674-t2676+t3022-t3027).*(t4595+t4658+t5189+t5207-t3468.*(t1005+t26.*(t1941-t3308+t39.*t1022.*(t855-t878).*2.196325630278387e-1))-t3420.*(t1896-t3232));
t6979 = (t2674-t2676+t3022-t3027).*(t4595+t4658+t5189+t5207-t3468.*(t1005+t26.*(t1941-t3308+t39.*t1022.*(t855-t878).*2.196325630278387e-1))-t3420.*(t1896-t3232));
t6987 = t50.*t202.*t6981.*9.543032792050485e-17;
t6989 = t2363.*t6980;
t7008 = t1544+t1559+t2320+t2323+t2329+t2341+t2379+t2380+t2510+t2534+t2978+t2979+t3152+t3367+t3893+t3920+t3939+t4106+t4152+t4155+t4805+t4809;
t7025 = t3229.*t6981;
t7026 = t3230.*t6981;
t7028 = t50.*t189.*(t1548+t1564+t2308-t2323+t2326+t2343+t2352+t2353-t2510+t2530+t2975-t2979+t3149+t3369-t3893+t3926+t3936+t4151-t4152-t4805-t4809+t22.*(t944-t3886).*(3.0./5.0e+2)).*(-9.543032792050485e-17);
t7031 = t1547+t2320+t2364+t2378+t2384+t2394+t2395+t2510+t2534+t2978+t2979+t3925+t3927+t3937+t4152+t4155+t4157+t4170+t4805+t4809;
t7044 = -t6980.*(t1896-t3232);
t7045 = t3528.*t6980;
t7049 = -t2297.*(t1553+t2308+t2359+t2365+t2366-t2378+t2389-t2510+t2530+t2975-t2979+t3921+t3933-t3937+t4151-t4152+t4162-t4805-t4809+t22.*(t944-t3886).*3.131399999999998e-4);
t7059 = t50.*t202.*t7043.*6.935255936130809e-19;
t7091 = t2363.*t7064.*7.26735e-3;
t3972 = t18.*t3967;
t3973 = t23.*t3967;
t4013 = t28.*t3996;
t4014 = t34.*t3996;
t4015 = -t4008;
t4016 = -t4010;
t4018 = -t4011;
t4075 = -t4071;
t4076 = -t4073;
t4077 = -t4074;
t4130 = -t4119;
t4226 = t3500+t3509;
t4248 = t3549+t3565;
t4276 = -t4275;
t4315 = t3132.*t3996;
t4316 = -t4311;
t4358 = -t3996.*(t2801-t2850);
t4361 = (t3230.*t3967)./1.0e+8;
t4380 = t18.*t4375;
t4389 = t18.*t4383;
t4391 = t3230.*t3967.*5.7e-7;
t4392 = t3230.*t3967.*1.02e-6;
t4393 = t3230.*t3967.*2.4e-7;
t4394 = t3230.*t3967.*4.0e-8;
t4493 = t3489+t3963;
t4503 = -t4502;
t4505 = -t4504;
t4506 = (t3528.*t3967)./1.0e+8;
t4519 = t3230.*t4224.*9.3e-7;
t4527 = t3230.*t4224.*9.0e-8;
t4537 = -t4533;
t4538 = t18.*t4528;
t4544 = t27.*t4528;
t4547 = -t4542;
t4548 = -t4543;
t4554 = t18.*t4543;
t4556 = t3528.*t3967.*5.7e-7;
t4557 = -t4549;
t4558 = t3528.*t3967.*1.02e-6;
t4559 = -t4551;
t4561 = -t4552;
t4564 = -t4555;
t4566 = t3531.*t3967.*5.7e-7;
t4567 = t27.*t4543;
t4568 = -t4560;
t4569 = t3528.*t3967.*2.4e-7;
t4570 = t3528.*t3967.*4.0e-8;
t4576 = t3531.*t3967.*4.0e-8;
t4577 = -t4571;
t4578 = -t4572;
t4598 = t3688.*t3996;
t4625 = t3788.*t3996;
t4626 = t3789.*t3996;
t4634 = t3528.*t4224.*9.3e-7;
t4635 = t3528.*t4224.*9.0e-8;
t4659 = -t4657;
t4674 = t3863.*t3996;
t4712 = -t4710;
t4713 = -t4711;
t4714 = (t3901.*t3967)./1.0e+8;
t4730 = t18.*t4723;
t4739 = t18.*t4726;
t4743 = -t4736;
t4748 = t18.*t4734;
t4751 = t3901.*t3967.*5.7e-7;
t4752 = t3901.*t3967.*1.02e-6;
t4753 = -t4741;
t4755 = -t4744;
t4757 = -t4746;
t4765 = t3901.*t3967.*2.4e-7;
t4766 = t3904.*t3967.*5.7e-7;
t4767 = t3901.*t3967.*4.0e-8;
t4774 = t3904.*t3967.*4.0e-8;
t4793 = t3229.*t4491.*9.3e-7;
t4794 = t3229.*t4491.*1.02e-6;
t4796 = t3229.*t4491.*9.0e-8;
t4825 = -t4819;
t4835 = t18.*t4828;
t4848 = t18.*t4846;
t4850 = t3957.*t3996.*1.02e-6;
t4851 = t3967.*t3992.*1.02e-6;
t4853 = -t4849;
t4858 = -t4856;
t4859 = -t4857;
t4895 = t3967.*t4113.*5.7e-7;
t4896 = t3967.*t4113.*4.0e-8;
t4904 = t3901.*t4224.*9.3e-7;
t4906 = t3901.*t4224.*9.0e-8;
t4912 = t3524.*t4491.*1.02e-6;
t4913 = t4491.*(t1896-t3232).*(-9.3e-7);
t4914 = t4491.*(t1896-t3232).*(-1.02e-6);
t4916 = t3524.*t4491.*9.0e-8;
t4918 = t4491.*(t1896-t3232).*1.02e-6;
t4919 = t4491.*(t1896-t3232).*(-9.0e-8);
t4924 = t4491.*(t1896-t3232).*9.0e-8;
t4929 = t27.*t4921;
t4932 = t27.*t4927;
t4955 = t3992.*t4224.*9.3e-7;
t4957 = t3992.*t4224.*9.0e-8;
t4970 = -t4247.*(-t2804+t2838+t3109+t23.*(t1456-t2355).*9.3e-7);
t4978 = t3737.*t4510;
t4979 = t3736.*t4514;
t5003 = t3845.*t4510;
t5004 = t3844.*t4514;
t5055 = -t5054;
t5057 = -t5056;
t5059 = t4491.*(t2694-t2701+t3036-t3043).*(-9.3e-7);
t5060 = t4491.*(t2694-t2701+t3036-t3043).*(-1.02e-6);
t5062 = t4491.*(t2694-t2701+t3036-t3043).*1.02e-6;
t5065 = t4491.*(t1959-t3306+t38.*t1022.*(t855-t878).*2.196325630278387e-1).*(-1.02e-6);
t5066 = t4491.*(t2694-t2701+t3036-t3043).*(-9.0e-8);
t5070 = t4491.*(t1959-t3306+t38.*t1022.*(t855-t878).*2.196325630278387e-1).*1.02e-6;
t5071 = t4491.*(t2694-t2701+t3036-t3043).*9.0e-8;
t5072 = t4491.*(t1959-t3306+t38.*t1022.*(t855-t878).*2.196325630278387e-1).*(-9.0e-8);
t5075 = t4491.*(t1959-t3306+t38.*t1022.*(t855-t878).*2.196325630278387e-1).*9.0e-8;
t5097 = t3945.*t4510;
t5098 = t3943.*t4514;
t5103 = t3985.*t4491.*1.02e-6;
t5104 = t3985.*t4491.*9.0e-8;
t5106 = t4491.*(t3235-t3535).*(-9.3e-7);
t5107 = t4491.*(t3235-t3535).*(-1.02e-6);
t5109 = t4491.*(t3235-t3535).*1.02e-6;
t5112 = t4491.*(t3235-t3535).*(-9.0e-8);
t5117 = t4491.*(t3235-t3535).*9.0e-8;
t5156 = t4491.*(t1005+t26.*(t1941-t3308+t39.*t1022.*(t855-t878).*2.196325630278387e-1)).*(-1.02e-6);
t5157 = t4491.*(t1005+t26.*(t1941-t3308+t39.*t1022.*(t855-t878).*2.196325630278387e-1)).*(-9.0e-8);
t5161 = -t5158;
t5166 = -t5162;
t5174 = -t4510.*(-t2804+t2838+t3109+t23.*(t1456-t2355).*9.3e-7);
t5175 = -t4510.*(t2813-t2835+t18.*(t1456-t2355).*1.02e-6+t23.*(t1456-t2355).*9.0e-8);
t5176 = t4125.*t4510;
t5177 = t4122.*t4514;
t5178 = -t4514.*(-t2804+t2838+t3109+t23.*(t1456-t2355).*9.3e-7);
t5179 = t4510.*(-t2804+t2838+t3109+t23.*(t1456-t2355).*9.3e-7);
t5180 = -t4514.*(t2813-t2835+t18.*(t1456-t2355).*1.02e-6+t23.*(t1456-t2355).*9.0e-8);
t5194 = -t5192;
t5215 = -t5211;
t5220 = t3513+t3597+t3609+t3610+t3611;
t5258 = t3224+t3510+t4021+t4022;
t5262 = t3227+t3515+t4025+t4026;
t5268 = -t5267;
t5271 = -t5270;
t5278 = t3967.*t4860.*5.7e-7;
t5279 = -t5275;
t5280 = -t5276;
t5284 = -t5282;
t5286 = t3967.*t4860.*4.0e-8;
t5300 = t3247+t3567+t4083+t4084;
t5314 = t3658+t3720+t3726+t3730+t3731;
t5321 = t3355+t3660+t4141+t4142;
t5333 = -t5331;
t5334 = -t5332;
t5336 = -t5335;
t5351 = t3252+t4375+t4383;
t5353 = t50.*t189.*(-t4007+t4011+t18.*(t1861-t3214).*1.838876e-2+t23.*(t1861-t3214).*9.99471e-3).*(-9.543032792050485e-17);
t5354 = t50.*t189.*(-t4007+t4011+t18.*(t1861-t3214).*1.838876e-2+t23.*(t1861-t3214).*9.99471e-3).*9.543032792050485e-17;
t5359 = -t2297.*(-t4007+t4011+t18.*(t1861-t3214).*1.838876e-2+t23.*(t1861-t3214).*9.99471e-3);
t5360 = t2297.*(-t4007+t4011+t18.*(t1861-t3214).*1.838876e-2+t23.*(t1861-t3214).*9.99471e-3);
t5367 = -t5365;
t5371 = -t5370;
t5374 = t50.*t202.*(t3547.*1.838876e-2+t4071-t4072+t34.*(t1896-t3232).*9.99471e-3).*(-6.935255936130809e-19);
t5375 = t50.*t202.*(t3547.*1.838876e-2+t4071-t4072+t34.*(t1896-t3232).*9.99471e-3).*6.935255936130809e-19;
t5394 = t2363.*(t3547.*1.838876e-2+t4071-t4072+t34.*(t1896-t3232).*9.99471e-3).*(-7.26735e-3);
t5397 = -t5091.*(-t1901+t3122+t3270);
t5413 = t628+t665+t675+t676+t1604+t1605+t1607+t1628+t2302+t3276+t3287+t3291+t3603+t3614;
t5415 = t4491.*(t4127+t33.*(t1959-t3306+t38.*t1022.*(t855-t878).*2.196325630278387e-1)).*(-1.02e-6);
t5416 = t4491.*(t4127+t33.*(t1959-t3306+t38.*t1022.*(t855-t878).*2.196325630278387e-1)).*1.02e-6;
t5417 = t4491.*(t4127+t33.*(t1959-t3306+t38.*t1022.*(t855-t878).*2.196325630278387e-1)).*(-9.0e-8);
t5419 = t4491.*(t4127+t33.*(t1959-t3306+t38.*t1022.*(t855-t878).*2.196325630278387e-1)).*9.0e-8;
t5426 = t58+t59+t5412;
t5429 = t429+t5412;
t5447 = t4491.*t4865.*1.02e-6;
t5453 = t4491.*t4865.*9.0e-8;
t5473 = -t5470;
t5474 = -t5471;
t5503 = -t27.*t2363.*(-t3423+t4543+t3946.*(t1896-t3232).*1.02e-6);
t5506 = t3901.*t4175.*t4651.*1.08769e-2;
t5520 = t4726+t4734;
t5521 = -t3003.*(-t3423+t4543+t3946.*(t1896-t3232).*1.02e-6);
t5526 = -t3057.*(-t3423+t4543+t3946.*(t1896-t3232).*1.02e-6);
t5528 = (t1477-t2502).*(-t3423+t4543+t3946.*(t1896-t3232).*1.02e-6);
t5533 = -t5532;
t5548 = t1205+t1217+t1218+t1230+t2147+t2164+t2166+t2167+t2759+t3395+t3399+t3409+t3716+t3728;
t5575 = -t5572;
t5583 = -t5582;
t5584 = t3271+t3297+t3573+t3605+t4021+t4022;
t5587 = t3275+t3302+t3612+t3615+t4025+t4026;
t5588 = t328+t338+t5539;
t5589 = t351+t363+t5539;
t5594 = t3901.*t4175.*t4897.*1.08769e-2;
t5600 = -t5599;
t5604 = -t5293.*(-t2804+t2838+t3109+t23.*(t1456-t2355).*9.3e-7);
t5608 = t2293+t2304+t3284+t3303+t5218;
t5609 = t2299+t3298+t3591+t3597+t3609+t3610+t3611+t3613;
t5618 = t3322+t3342+t3651+t3656+t4083+t4084;
t5628 = t3877.*t4134.*t4975;
t5632 = t27.*(t1896-t3232).*(-t3423+t4543+t3946.*(t1896-t3232).*1.02e-6);
t5635 = -t27.*t3528.*(-t3423+t4543+t3946.*(t1896-t3232).*1.02e-6);
t5642 = t2398+t3345+t3636+t3640+t3646+t3652+t3653+t3654;
t5643 = t2370+t2494+t3340+t3358+t3564+t3640+t3646+t3653+t3654;
t5659 = -t5658;
t5667 = -t5666;
t5687 = t3210.*t5555;
t5690 = -t5688;
t5693 = -t5691;
t5712 = -t5711;
et162 = -t2306-t2317+t3144+t3147+t35.*t941.*t948.*(t850-t874).*3.775747223193135e-1;
et163 = t36.*t941.*t948.*(t850-t874).*2.244797987218524e-1;
t5726 = -t5091.*(et162+et163);
t5733 = -t5732;
t5739 = t3677+t4833+t4846;
t5740 = -t3985.*(-t3423+t4543+t3946.*(t1896-t3232).*1.02e-6);
t5741 = (t3235-t3535).*(-t3423+t4543+t3946.*(t1896-t3232).*1.02e-6);
t5742 = t3985.*(-t3423+t4543+t3946.*(t1896-t3232).*1.02e-6);
t5744 = -t3992.*(-t3423+t4543+t3946.*(t1896-t3232).*1.02e-6);
t5747 = -t3996.*(-t3423+t4543+t3946.*(t1896-t3232).*1.02e-6);
t5748 = t3992.*(-t3423+t4543+t3946.*(t1896-t3232).*1.02e-6);
t5749 = t3996.*(-t3423+t4543+t3946.*(t1896-t3232).*1.02e-6);
t5753 = -t5751;
t5782 = t3877.*t5555;
t5786 = -t5785;
t5796 = t70+t76+t90+t91+t2675+t2678+t2690+t2695+t3223+t3508+t3579+t3584+t4008+t4010;
t5817 = t3481.*t5755;
t5843 = t360+t364+t365+t371+t2946+t2951+t2954+t2956+t3348+t3650+t3700+t3711+t4118+t4121;
t5854 = t3066+t3212+t4033+t4052+t4357+t4359;
t5858 = t3901.*t4175.*t5412.*1.08769e-2;
t5862 = -t5860;
t5867 = t3882.*t5755;
t5897 = -t4814.*(-t3423+t4543+t3946.*(t1896-t3232).*1.02e-6);
t5899 = t4814.*(-t3423+t4543+t3946.*(t1896-t3232).*1.02e-6);
t5901 = (t4127+t33.*(t1959-t3306+t38.*t1022.*(t855-t878).*2.196325630278387e-1)).*(-t3423+t4543+t3946.*(t1896-t3232).*1.02e-6);
t5903 = (-t4007+t4011+t18.*(t1861-t3214).*1.838876e-2+t23.*(t1861-t3214).*9.99471e-3).*(t2694-t2701+t3036-t3043).*(t1513+t1879+t2598+t2820+t2834+t3117+t3118).*(-7.26735e-3);
t5904 = (-t4007+t4011+t18.*(t1861-t3214).*1.838876e-2+t23.*(t1861-t3214).*9.99471e-3).*(t2694-t2701+t3036-t3043).*(t1513+t1879+t2598+t2820+t2834+t3117+t3118).*7.26735e-3;
t5915 = -t3996.*(t3081-t3086+t4048-t4061+t4067+t17.*t3229.*(t1861-t3214).*4.0e-8);
t5916 = t3996.*(t3081-t3086+t4048-t4061+t4067+t17.*t3229.*(t1861-t3214).*4.0e-8);
t5923 = t4080.*t5755;
t5933 = -(t3547.*1.33637554986e-4+t4119-t4120+t34.*(t1896-t3232).*7.26350557185e-5).*(t2674-t2676+t3022-t3027).*(t1488+t1874+t2519+t2740+t2747+t3096+t3097);
t5950 = -t4651.*(t350+t366-t1205+t1210-t1217-t1218-t2147+t2152+t2154+t2155-t3395-t3399-t3409-t3716+t3723+t32.*t50.*t202.*(t46-t47).*8.687615694748404e-39);
t5952 = t4651.*(t350+t366-t1205+t1210-t1217-t1218-t2147+t2152+t2154+t2155-t3395-t3399-t3409-t3716+t3723+t32.*t50.*t202.*(t46-t47).*8.687615694748404e-39);
t5961 = t3877.*t4134.*t5539;
t5971 = -t5970;
t5991 = -t4897.*(t350+t366-t1205+t1210-t1217-t1218-t2147+t2152+t2154+t2155-t3395-t3399-t3409-t3716+t3723+t32.*t50.*t202.*(t46-t47).*8.687615694748404e-39);
t5996 = t2363.*t5974;
t6000 = -t5998;
t6010 = -t6009;
t6015 = -t6011;
t6031 = -t6030;
t6034 = -t6032;
t6038 = t3253+t3264+t4381+t4385+t4390+t4395;
t6049 = -t5974.*(t1896-t3232);
t6050 = t3528.*t5974;
t6051 = t4822.*t5755;
t6076 = t3210.*t6027;
t6101 = t5737.*(t2674-t2676+t3022-t3027).*(t1488+t1874+t2519+t2740+t2747+t3096+t3097);
t6136 = -t3996.*(t4474+t4481-t4484-t4488);
t6137 = t3996.*(t4474+t4481-t4484-t4488);
t6144 = -t3481.*(t4510.*(t2813-t2835+t18.*(t1456-t2355).*1.02e-6+t23.*(t1456-t2355).*9.0e-8)+t4514.*(-t2804+t2838+t3109+t23.*(t1456-t2355).*9.3e-7)+t3132.*(t3235-t3535));
t6147 = t17.*(t1861-t3214).*(t4510.*(t2813-t2835+t18.*(t1456-t2355).*1.02e-6+t23.*(t1456-t2355).*9.0e-8)+t4514.*(-t2804+t2838+t3109+t23.*(t1456-t2355).*9.3e-7)+t3132.*(t3235-t3535));
t6156 = t50.*t189.*t6128.*9.543032792050485e-17;
t6162 = t3057.*t6097;
t6169 = t2297.*t6128;
t6198 = t3047.*t6128;
t6200 = t3877.*t6027;
t6205 = t667+t672+t673+t691+t1591+t1602+t1626+t1627+t2301+t2675+t2678+t2690+t2695+t3277+t3280+t3296+t3572+t3579+t3584+t3593+t4008+t4010;
t6232 = -(t4610+t2363.*(t3547.*1.838876e-2+t4071-t4072+t34.*(t1896-t3232).*9.99471e-3).*7.26735e-3).*(t2674-t2676+t3022-t3027).*(t1488+t1874+t2519+t2740+t2747+t3096+t3097);
t6238 = -t3882.*(t4510.*(t2813-t2835+t18.*(t1456-t2355).*1.02e-6+t23.*(t1456-t2355).*9.0e-8)+t4514.*(-t2804+t2838+t3109+t23.*(t1456-t2355).*9.3e-7)+t3132.*(t3235-t3535));
t6257 = -t3942.*(t4510.*(t2813-t2835+t18.*(t1456-t2355).*1.02e-6+t23.*(t1456-t2355).*9.0e-8)+t4514.*(-t2804+t2838+t3109+t23.*(t1456-t2355).*9.3e-7)+t3132.*(t3235-t3535));
t6278 = t710+t717+t718+t756+t1690+t1738+t1752+t1753+t2400+t2705+t2711+t2713+t2716+t3325+t3327+t3341+t3620+t3625+t3630+t3638+t4073+t4074;
t6293 = -t4080.*(t4510.*(t2813-t2835+t18.*(t1456-t2355).*1.02e-6+t23.*(t1456-t2355).*9.0e-8)+t4514.*(-t2804+t2838+t3109+t23.*(t1456-t2355).*9.3e-7)+t3132.*(t3235-t3535));
t6302 = -t3385.*(t4555+t4571-t18.*t2363.*t3047.*9.0e-8-t23.*t2363.*t3047.*9.3e-7+t18.*t3946.*(t1896-t3232).*9.0e-8+t23.*t3946.*(t1896-t3232).*9.3e-7);
t6303 = t3385.*(t4555+t4571-t18.*t2363.*t3047.*9.0e-8-t23.*t2363.*t3047.*9.3e-7+t18.*t3946.*(t1896-t3232).*9.0e-8+t23.*t3946.*(t1896-t3232).*9.3e-7);
t6313 = t4740+t4749+t4756+t4768;
t6326 = t3859+t4621+t4622+t4624+t4670;
t6343 = -t6097.*(t3235-t3535);
t6344 = t3992.*t6097;
et164 = t707+t708-t721-t722-t749+t762+t768-t777-t792-t793-t801-t802-t808+t813-t819+t821-t1629+t1637-t1640-t1641-t1659-t1661+t1666+t1667+t1683+t1692+t1705-t1712+t1758+t1759+t1775+t1776+t1973+t1993+t1994+t2023+t2053+t2060-t2089-t2090+t2098+t2099-t14.*t15.*t21.*t50.*t189.*3.670836568391568e-22;
tau_c = ft_12({et164,t1005,t1022,t1089,t1104,t1105,t1108,t1115,t1121,t1158,t1159,t1196,t1205,t1210,t1212,t1217,t1218,t123,t1237,t1238,t1288,t1289,t1302,t1303,t1319,t1320,t1336,t1348,t1350,t1351,t1360,t1369,t1378,t1396,t14,t140,t1425,t1435,t1456,t1477,t1488,t15,t1513,t1539,t1554,t1576,t1577,t1578,t1579,t1584,t1585,t1586,t1587,t1599,t16,t1600,t1604,t1605,t1606,t1607,t1608,t1609,t1613,t1614,t1615,t1616,t1628,t1629,t1631,t1637,t1640,t1641,t1648,t1649,t1659,t1660,t1661,t1666,t1667,t1683,t1686,t1690,t1692,t17,t1700,t1701,t1704,t1705,t1712,t1717,t1741,t1742,t1750,t1754,t1758,t1759,t1775,t1776,t18,t1861,t1874,t1879,t188,t1881,t189,t1896,t19,t1901,t1941,t1959,t1973,t1993,t1994,t2,t20,t201,t202,t2023,t2053,t2060,t2089,t2090,t2098,t2099,t21,t2117,t2120,t2122,t2123,t2137,t2139,t2140,t2147,t2152,t2154,t2155,t2159,t2165,t2174,t2183,t2187,t2193,t2194,t2195,t2199,t22,t2203,t2215,t2219,t2222,t2223,t2239,t2240,t2256,t2257,t2291,t2292,t2294,t2295,t2297,t23,t2302,t2303,t2306,t2307,t2308,t2311,t2317,t2325,t2337,t2338,t2339,t2344,t2355,t236,t2360,t2361,t2362,t2363,t2367,t2368,t237,t2371,t2378,t238,t2388,t2391,t24,t2401,t2403,t2404,t2405,t241,t2414,t2419,t2421,t2438,t244,t2448,t2449,t2461,t2471,t2472,t2492,t2493,t25,t2502,t2510,t2519,t2527,t2530,t2555,t2556,t2572,t2575,t2583,t2598,t26,t2605,t2606,t2612,t2613,t2618,t2619,t262,t2638,t264,t2651,t2652,t2670,t2671,t2673,t2674,t2676,t2680,t2683,t2684,t2685,t2686,t2687,t2689,t2692,t2693,t2694,t2695,t2696,t2697,t2698,t27,t2700,t2701,t2704,t2707,t2708,t2709,t2712,t2715,t2716,t2717,t2719,t2720,t2721,t2736,t2740,t2747,t2754,t2777,t2778,t2779,t2787,t2797,t28,t2801,t2804,t2813,t2814,t2820,t2831,t2834,t2835,t2838,t2850,t2851,t2937,t2942,t2945,t2950,t2953,t2955,t2957,t2963,t2964,t2975,t2979,t2984,t2987,t2990,t2991,t2993,t2994,t2998,t3,t30,t3003,t3004,t3008,t3009,t3015,t3017,t3022,t3027,t3029,t3030,t3036,t3043,t3044,t3045,t3047,t3049,t3054,t3055,t3056,t3057,t3063,t3064,t3068,t3072,t3079,t3080,t3096,t3097,t31,t3109,t3117,t3118,t3121,t3122,t3128,t3129,t313,t3130,t3131,t3132,t3133,t3134,t3135,t3139,t314,t3140,t3141,t3142,t3144,t3147,t3153,t3155,t3156,t3157,t3158,t3159,t3160,t3161,t3162,t3163,t3164,t3166,t3170,t3171,t3172,t3179,t3180,t3184,t3186,t3187,t3188,t3189,t3190,t3191,t3193,t3194,t3196,t3197,t3198,t3199,t32,t3200,t3201,t3206,t3209,t321,t3210,t3214,t3218,t3225,t3226,t3228,t3229,t3230,t3231,t3232,t3235,t3245,t3246,t3249,t3250,t3254,t3256,t3258,t3259,t326,t3260,t3261,t3262,t3263,t3265,t3266,t3269,t3270,t3272,t3276,t3281,t3283,t329,t3290,t3291,t3292,t3295,t3296,t33,t3300,t3305,t3306,t3307,t3308,t3309,t331,t3313,t3316,t3318,t3319,t332,t3324,t3326,t3327,t3328,t333,t3330,t3333,t3334,t3335,t3336,t3337,t3341,t3344,t3347,t3349,t335,t3353,t3354,t3357,t3359,t3360,t3373,t3376,t3377,t3379,t3382,t3384,t3385,t3386,t339,t3395,t3399,t34,t3405,t3409,t3410,t3412,t3415,t3417,t3419,t3420,t3421,t3422,t3423,t3424,t3427,t3428,t3429,t3430,t3432,t3433,t3434,t3435,t3436,t3437,t3438,t3440,t3441,t3442,t3443,t3444,t3445,t3446,t3447,t3449,t3450,t3451,t3453,t3455,t3456,t346,t3465,t3468,t3470,t3473,t3475,t3477,t3479,t3480,t3481,t3483,t3484,t3491,t3493,t3498,t35,t350,t3503,t3505,t3512,t3518,t3522,t3524,t3526,t3527,t3528,t3530,t3531,t3532,t3533,t3535,t3539,t354,t3542,t3543,t3544,t3547,t3550,t3558,t3559,t356,t3560,t3562,t3563,t3569,t3570,t3571,t3576,t3577,t3578,t358,t3582,t3585,t3586,t3587,t3588,t3589,t359,t3590,t3593,t3596,t36,t3600,t3603,t3616,t3617,t3618,t3619,t362,t3620,t3621,t3622,t3623,t3624,t3628,t3631,t3632,t3633,t3634,t3635,t3637,t3638,t3639,t3641,t3643,t3649,t3657,t366,t3663,t3664,t3665,t3667,t3669,t3670,t3672,t3673,t3674,t3676,t3678,t3679,t3680,t3681,t3682,t3683,t3684,t3685,t3686,t3687,t3689,t3690,t3693,t3694,t3699,t3703,t3705,t3706,t3708,t3709,t3712,t3713,t3714,t3715,t3716,t3718,t372,t3723,t3724,t3729,t3732,t3734,t3735,t3736,t3737,t3744,t3745,t3746,t3748,t3749,t3751,t3753,t3755,t3756,t3757,t3758,t3759,t3760,t3762,t3763,t3764,t3765,t3766,t3767,t3768,t3769,t3770,t3771,t3772,t3774,t3775,t3776,t3778,t3779,t378,t3782,t3783,t3784,t3790,t3791,t3794,t3795,t3797,t3798,t3799,t38,t380,t3801,t3803,t3804,t3806,t3811,t3814,t3815,t3816,t3817,t3819,t382,t3821,t3822,t3826,t3827,t3828,t3833,t3834,t3844,t3845,t3847,t3849,t3850,t3860,t3861,t3862,t3863,t3865,t3866,t3869,t387,t3870,t3871,t3872,t3875,t3876,t3877,t3880,t3882,t3891,t3892,t3893,t3898,t39,t3901,t3904,t3910,t3916,t3918,t3922,t3928,t3934,t3940,t3941,t3942,t3943,t3945,t3946,t3949,t3951,t3954,t3957,t3958,t3959,t3962,t3964,t3965,t3967,t3968,t3972,t3973,t3974,t3976,t3980,t3984,t3985,t3992,t3996,t4,t4007,t4011,t4012,t4013,t4014,t4015,t4016,t4018,t4027,t4062,t4071,t4072,t4075,t4076,t4077,t4080,t410,t4106,t4108,t4109,t4113,t4119,t4120,t4122,t4125,t4127,t4130,t4133,t4134,t4149,t4150,t4152,t4154,t4155,t4160,t4163,t4168,t4173,t4175,t4178,t4179,t4184,t4189,t4190,t4196,t42,t4200,t4201,t4202,t4203,t4205,t4207,t4208,t4217,t4219,t4220,t4221,t4226,t4227,t4228,t4230,t4231,t4233,t4234,t4235,t4236,t4237,t4238,t4239,t4240,t4242,t4243,t4244,t4245,t4246,t4247,t4248,t4249,t4250,t4251,t4252,t4253,t4254,t4255,t4256,t4257,t4259,t4260,t4261,t4262,t4263,t4264,t4266,t4267,t4268,t4274,t4276,t4277,t4279,t4280,t4281,t4285,t4287,t429,t4291,t4292,t4295,t4296,t4297,t4298,t43,t4304,t4306,t4307,t4308,t4310,t4311,t4313,t4314,t4315,t4316,t4321,t4322,t4323,t4324,t4354,t4356,t4358,t4361,t4362,t4363,t4369,t4370,t4373,t4374,t4376,t4377,t4378,t4379,t4380,t4382,t4386,t4387,t4388,t4389,t4391,t4392,t4393,t4394,t4396,t4400,t4404,t4405,t4406,t4409,t4410,t4411,t4412,t4413,t4415,t4421,t4424,t4427,t4428,t4429,t4432,t4434,t4436,t4437,t4438,t4439,t4440,t4444,t4447,t4458,t4460,t4461,t4464,t4473,t4475,t4491,t4496,t4498,t4499,t4500,t4501,t4503,t4504,t4505,t4506,t4507,t4508,t4510,t4511,t4513,t4514,t4515,t4516,t4517,t4519,t4520,t4521,t4522,t4525,t4526,t4527,t4528,t4530,t4531,t4532,t4535,t4536,t4537,t4538,t4539,t4543,t4545,t4546,t4547,t4548,t4550,t4552,t4554,t4555,t4556,t4557,t4558,t4559,t4560,t4561,t4562,t4563,t4564,t4566,t4567,t4568,t4569,t4570,t4571,t4572,t4576,t4577,t4578,t4579,t4581,t4582,t4583,t4584,t4586,t4587,t4588,t4589,t4591,t4593,t4594,t4595,t4597,t4598,t4599,t46,t4602,t4604,t4606,t4607,t4609,t4610,t4611,t4612,t4613,t4614,t4615,t4617,t4620,t4623,t4625,t4626,t4627,t4628,t4629,t4631,t4633,t4634,t4635,t4640,t4641,t4642,t4644,t4645,t4647,t4649,t4650,t4651,t4652,t4655,t4658,t4659,t4661,t4663,t4664,t4666,t4667,t4669,t4672,t4674,t4676,t4678,t4679,t4680,t4682,t4683,t4685,t4686,t4688,t4699,t47,t4702,t4703,t4704,t4705,t4706,t4708,t4709,t4712,t4713,t4714,t4716,t4718,t4719,t4720,t4721,t4725,t4727,t4728,t4729,t4732,t4733,t4735,t4737,t4738,t4739,t4741,t4742,t4743,t4744,t4748,t4751,t4752,t4753,t4755,t4757,t4758,t4759,t4760,t4762,t4765,t4766,t4767,t4769,t4770,t4772,t4774,t4777,t4780,t4785,t4786,t4787,t4788,t4789,t4790,t4791,t4792,t4793,t4794,t4795,t4796,t4798,t4799,t4800,t4801,t4805,t4809,t4814,t4816,t4817,t4818,t4819,t4822,t4823,t4824,t4825,t4826,t4829,t4832,t4833,t4835,t4836,t4839,t4840,t4842,t4843,t4845,t4847,t4848,t4849,t4850,t4851,t4852,t4853,t4856,t4857,t4858,t4859,t4860,t4863,t4864,t4865,t4866,t4867,t4868,t4869,t4870,t4871,t4872,t4873,t4874,t4875,t4876,t4877,t4880,t4881,t4882,t4883,t4884,t4885,t4886,t4887,t4888,t4890,t4892,t4893,t4894,t4895,t4896,t4897,t4898,t4899,t4900,t4902,t4904,t4905,t4906,t4911,t4912,t4913,t4914,t4916,t4917,t4918,t4919,t4921,t4922,t4924,t4925,t4927,t4929,t4931,t4932,t4950,t4952,t4953,t4954,t4955,t4957,t4961,t4962,t4963,t4965,t4968,t4969,t4970,t4973,t4974,t4975,t4976,t4977,t4978,t4979,t4982,t4983,t4984,t4985,t4986,t4987,t4992,t4994,t4995,t4996,t4998,t5,t50,t5000,t5001,t5002,t5003,t5004,t5005,t5007,t5010,t5012,t5013,t5014,t5015,t5017,t5021,t5022,t5023,t5025,t5026,t5027,t5028,t5030,t5031,t5032,t5033,t5034,t5035,t5036,t5038,t5039,t5040,t5041,t5042,t5047,t5048,t5049,t5051,t5052,t5053,t5054,t5055,t5056,t5057,t5058,t5059,t5061,t5062,t5063,t5064,t5066,t5067,t5068,t5069,t5070,t5071,t5073,t5074,t5075,t5076,t5077,t5092,t5094,t5096,t5097,t5098,t5103,t5104,t5105,t5106,t5108,t5109,t5111,t5112,t5113,t5114,t5115,t5116,t5117,t5118,t5119,t5121,t5123,t5124,t5126,t5127,t5128,t5130,t5131,t5144,t5145,t5146,t5147,t5148,t5149,t5150,t5151,t5152,t5153,t5155,t5156,t5157,t5158,t5161,t5162,t5164,t5165,t5166,t5169,t5175,t5176,t5177,t5178,t5179,t5180,t5184,t5189,t5190,t5191,t5192,t5193,t5194,t5195,t5196,t5198,t5201,t5202,t5203,t5204,t5206,t5207,t5208,t5209,t5210,t5212,t5213,t5214,t5215,t5216,t5217,t5219,t5220,t5221,t5222,t5223,t5224,t5225,t5226,t5227,t5228,t5229,t5230,t5231,t5232,t5233,t5234,t5235,t5236,t5237,t5238,t5239,t5240,t5241,t5242,t5243,t5244,t5245,t5246,t5247,t5248,t5250,t5252,t5254,t5255,t5257,t5258,t5260,t5261,t5262,t5268,t5269,t5270,t5271,t5272,t5273,t5274,t5275,t5276,t5277,t5278,t5279,t5280,t5281,t5282,t5284,t5285,t5286,t5288,t5289,t5291,t5293,t5295,t5300,t5301,t5302,t5304,t5306,t5307,t5308,t5314,t5316,t5317,t5320,t5321,t5322,t5328,t5330,t5331,t5332,t5333,t5335,t5336,t5337,t5338,t5339,t5340,t5342,t5344,t5345,t5346,t5347,t5348,t5349,t5350,t5351,t5354,t5356,t5357,t5358,t5359,t5360,t5361,t5362,t5365,t5367,t5369,t5370,t5371,t5375,t5377,t5379,t5380,t5381,t5383,t5384,t5385,t5386,t5387,t5388,t5389,t5390,t5391,t5392,t5393,t5394,t5395,t5396,t5397,t5399,t5402,t5403,t5405,t5407,t5408,t5409,t5411,t5412,t5413,t5416,t5418,t5419,t5420,t5426,t5427,t5428,t5429,t5433,t5434,t5440,t5441,t5443,t5444,t5445,t5446,t5447,t5448,t5449,t5451,t5452,t5453,t5454,t5455,t5457,t5458,t5459,t5461,t5462,t5465,t5467,t5468,t5469,t5472,t5473,t5474,t5476,t5477,t5480,t5481,t5482,t5483,t5484,t5485,t5486,t5487,t5488,t5489,t5490,t5491,t5492,t5493,t5494,t5496,t5498,t5499,t5500,t5503,t5504,t5505,t5506,t5509,t5514,t5515,t5516,t5517,t5518,t5520,t5521,t5522,t5523,t5524,t5525,t5526,t5528,t5531,t5532,t5533,t5534,t5535,t5536,t5537,t5538,t5539,t5541,t5542,t5543,t5544,t5545,t5546,t5547,t5548,t5550,t5551,t5552,t5553,t5554,t5556,t5557,t5558,t5559,t5561,t5564,t5566,t5569,t5570,t5573,t5574,t5575,t5576,t5577,t5578,t5579,t5580,t5581,t5582,t5583,t5584,t5587,t5588,t5589,t5592,t5593,t5594,t5595,t5597,t5598,t56,t5600,t5601,t5602,t5603,t5604,t5605,t5606,t5609,t5617,t5618,t5619,t5620,t5621,t5622,t5626,t5627,t5628,t5631,t5632,t5635,t5639,t5640,t5642,t5643,t5658,t5659,t5660,t5661,t5662,t5663,t5664,t5666,t5667,t5670,t5671,t5674,t5675,t5676,t5678,t5679,t5681,t5682,t5685,t5687,t5689,t5690,t5691,t5693,t5694,t5695,t5699,t5700,t5701,t5702,t5703,t5705,t5706,t5707,t5708,t5709,t5711,t5712,t5717,t5718,t5720,t5721,t5722,t5723,t5725,t5726,t5727,t5728,t5730,t5731,t5733,t5735,t5737,t5739,t5740,t5741,t5742,t5748,t5749,t5750,t5751,t5752,t5753,t5760,t5761,t5764,t5765,t5766,t5767,t5768,t5770,t5775,t5779,t5782,t5785,t5786,t5791,t5792,t5793,t5794,t5796,t58,t5804,t5805,t5806,t5807,t5817,t5826,t5827,t5828,t5832,t5835,t5839,t5840,t5843,t5846,t5852,t5853,t5854,t5855,t5857,t5858,t5859,t5860,t5861,t5862,t5864,t5866,t5867,t5868,t5871,t5876,t5879,t5890,t5891,t5894,t5896,t5899,t59,t5900,t5901,t5904,t5907,t5908,t5910,t5911,t5912,t5913,t5914,t5916,t5922,t5923,t5930,t5932,t5933,t5941,t5943,t5944,t5951,t5952,t5953,t5954,t5958,t5961,t5966,t5969,t5970,t5975,t5977,t5991,t5992,t5994,t5996,t5998,t5999,t6,t60,t6000,t6002,t6004,t6009,t6010,t6012,t6014,t6015,t6016,t6017,t6018,t6019,t6020,t6021,t6028,t6030,t6031,t6034,t6038,t6049,t6050,t6051,t6054,t6057,t6058,t6059,t6060,t6062,t6064,t6066,t6067,t6075,t6076,t6085,t6087,t6091,t6092,t6095,t6096,t6101,t6112,t6135,t6137,t6143,t6144,t6147,t6151,t6153,t6156,t6162,t6169,t6183,t6184,t6185,t6198,t6199,t6200,t6206,t6207,t6209,t6219,t6221,t6232,t6238,t6247,t6253,t6257,t6293,t6302,t6303,t6313,t6317,t6321,t6322,t6323,t6339,t6341,t6343,t6344,t6356,t6366,t6367,t6375,t638,t6387,t6388,t640,t6406,t6414,t642,t643,t6442,t6450,t6451,t6453,t6484,t6485,t6486,t649,t6493,t6506,t6507,t6508,t6511,t6515,t6520,t6529,t654,t6543,t6544,t655,t656,t6565,t657,t6575,t6576,t659,t6593,t660,t6611,t6612,t6658,t6663,t667,t668,t6689,t669,t6691,t6692,t67,t670,t674,t677,t68,t681,t6811,t6812,t6813,t682,t684,t685,t686,t6860,t6861,t687,t6892,t6893,t6913,t6916,t6917,t692,t6922,t693,t6937,t694,t6979,t6980,t6987,t6989,t7,t702,t7025,t7026,t7028,t7029,t7039,t7041,t7044,t7045,t7049,t7051,t7059,t707,t708,t7091,t71,t710,t715,t716,t7204,t721,t7219,t722,t7227,t7228,t7229,t7230,t724,t725,t73,t736,t738,t740,t741,t749,t762,t768,t777,t792,t793,t801,t802,t808,t813,t819,t821,t850,t855,t874,t878,t89,t92,t941,t948,t951,t97});
end
function tau_c = ft_12(ct)
et164 = ct{1};
t1005 = ct{2};
t1022 = ct{3};
t1089 = ct{4};
t1104 = ct{5};
t1105 = ct{6};
t1108 = ct{7};
t1115 = ct{8};
t1121 = ct{9};
t1158 = ct{10};
t1159 = ct{11};
t1196 = ct{12};
t1205 = ct{13};
t1210 = ct{14};
t1212 = ct{15};
t1217 = ct{16};
t1218 = ct{17};
t123 = ct{18};
t1237 = ct{19};
t1238 = ct{20};
t1288 = ct{21};
t1289 = ct{22};
t1302 = ct{23};
t1303 = ct{24};
t1319 = ct{25};
t1320 = ct{26};
t1336 = ct{27};
t1348 = ct{28};
t1350 = ct{29};
t1351 = ct{30};
t1360 = ct{31};
t1369 = ct{32};
t1378 = ct{33};
t1396 = ct{34};
t14 = ct{35};
t140 = ct{36};
t1425 = ct{37};
t1435 = ct{38};
t1456 = ct{39};
t1477 = ct{40};
t1488 = ct{41};
t15 = ct{42};
t1513 = ct{43};
t1539 = ct{44};
t1554 = ct{45};
t1576 = ct{46};
t1577 = ct{47};
t1578 = ct{48};
t1579 = ct{49};
t1584 = ct{50};
t1585 = ct{51};
t1586 = ct{52};
t1587 = ct{53};
t1599 = ct{54};
t16 = ct{55};
t1600 = ct{56};
t1604 = ct{57};
t1605 = ct{58};
t1606 = ct{59};
t1607 = ct{60};
t1608 = ct{61};
t1609 = ct{62};
t1613 = ct{63};
t1614 = ct{64};
t1615 = ct{65};
t1616 = ct{66};
t1628 = ct{67};
t1629 = ct{68};
t1631 = ct{69};
t1637 = ct{70};
t1640 = ct{71};
t1641 = ct{72};
t1648 = ct{73};
t1649 = ct{74};
t1659 = ct{75};
t1660 = ct{76};
t1661 = ct{77};
t1666 = ct{78};
t1667 = ct{79};
t1683 = ct{80};
t1686 = ct{81};
t1690 = ct{82};
t1692 = ct{83};
t17 = ct{84};
t1700 = ct{85};
t1701 = ct{86};
t1704 = ct{87};
t1705 = ct{88};
t1712 = ct{89};
t1717 = ct{90};
t1741 = ct{91};
t1742 = ct{92};
t1750 = ct{93};
t1754 = ct{94};
t1758 = ct{95};
t1759 = ct{96};
t1775 = ct{97};
t1776 = ct{98};
t18 = ct{99};
t1861 = ct{100};
t1874 = ct{101};
t1879 = ct{102};
t188 = ct{103};
t1881 = ct{104};
t189 = ct{105};
t1896 = ct{106};
t19 = ct{107};
t1901 = ct{108};
t1941 = ct{109};
t1959 = ct{110};
t1973 = ct{111};
t1993 = ct{112};
t1994 = ct{113};
t2 = ct{114};
t20 = ct{115};
t201 = ct{116};
t202 = ct{117};
t2023 = ct{118};
t2053 = ct{119};
t2060 = ct{120};
t2089 = ct{121};
t2090 = ct{122};
t2098 = ct{123};
t2099 = ct{124};
t21 = ct{125};
t2117 = ct{126};
t2120 = ct{127};
t2122 = ct{128};
t2123 = ct{129};
t2137 = ct{130};
t2139 = ct{131};
t2140 = ct{132};
t2147 = ct{133};
t2152 = ct{134};
t2154 = ct{135};
t2155 = ct{136};
t2159 = ct{137};
t2165 = ct{138};
t2174 = ct{139};
t2183 = ct{140};
t2187 = ct{141};
t2193 = ct{142};
t2194 = ct{143};
t2195 = ct{144};
t2199 = ct{145};
t22 = ct{146};
t2203 = ct{147};
t2215 = ct{148};
t2219 = ct{149};
t2222 = ct{150};
t2223 = ct{151};
t2239 = ct{152};
t2240 = ct{153};
t2256 = ct{154};
t2257 = ct{155};
t2291 = ct{156};
t2292 = ct{157};
t2294 = ct{158};
t2295 = ct{159};
t2297 = ct{160};
t23 = ct{161};
t2302 = ct{162};
t2303 = ct{163};
t2306 = ct{164};
t2307 = ct{165};
t2308 = ct{166};
t2311 = ct{167};
t2317 = ct{168};
t2325 = ct{169};
t2337 = ct{170};
t2338 = ct{171};
t2339 = ct{172};
t2344 = ct{173};
t2355 = ct{174};
t236 = ct{175};
t2360 = ct{176};
t2361 = ct{177};
t2362 = ct{178};
t2363 = ct{179};
t2367 = ct{180};
t2368 = ct{181};
t237 = ct{182};
t2371 = ct{183};
t2378 = ct{184};
t238 = ct{185};
t2388 = ct{186};
t2391 = ct{187};
t24 = ct{188};
t2401 = ct{189};
t2403 = ct{190};
t2404 = ct{191};
t2405 = ct{192};
t241 = ct{193};
t2414 = ct{194};
t2419 = ct{195};
t2421 = ct{196};
t2438 = ct{197};
t244 = ct{198};
t2448 = ct{199};
t2449 = ct{200};
t2461 = ct{201};
t2471 = ct{202};
t2472 = ct{203};
t2492 = ct{204};
t2493 = ct{205};
t25 = ct{206};
t2502 = ct{207};
t2510 = ct{208};
t2519 = ct{209};
t2527 = ct{210};
t2530 = ct{211};
t2555 = ct{212};
t2556 = ct{213};
t2572 = ct{214};
t2575 = ct{215};
t2583 = ct{216};
t2598 = ct{217};
t26 = ct{218};
t2605 = ct{219};
t2606 = ct{220};
t2612 = ct{221};
t2613 = ct{222};
t2618 = ct{223};
t2619 = ct{224};
t262 = ct{225};
t2638 = ct{226};
t264 = ct{227};
t2651 = ct{228};
t2652 = ct{229};
t2670 = ct{230};
t2671 = ct{231};
t2673 = ct{232};
t2674 = ct{233};
t2676 = ct{234};
t2680 = ct{235};
t2683 = ct{236};
t2684 = ct{237};
t2685 = ct{238};
t2686 = ct{239};
t2687 = ct{240};
t2689 = ct{241};
t2692 = ct{242};
t2693 = ct{243};
t2694 = ct{244};
t2695 = ct{245};
t2696 = ct{246};
t2697 = ct{247};
t2698 = ct{248};
t27 = ct{249};
t2700 = ct{250};
t2701 = ct{251};
t2704 = ct{252};
t2707 = ct{253};
t2708 = ct{254};
t2709 = ct{255};
t2712 = ct{256};
t2715 = ct{257};
t2716 = ct{258};
t2717 = ct{259};
t2719 = ct{260};
t2720 = ct{261};
t2721 = ct{262};
t2736 = ct{263};
t2740 = ct{264};
t2747 = ct{265};
t2754 = ct{266};
t2777 = ct{267};
t2778 = ct{268};
t2779 = ct{269};
t2787 = ct{270};
t2797 = ct{271};
t28 = ct{272};
t2801 = ct{273};
t2804 = ct{274};
t2813 = ct{275};
t2814 = ct{276};
t2820 = ct{277};
t2831 = ct{278};
t2834 = ct{279};
t2835 = ct{280};
t2838 = ct{281};
t2850 = ct{282};
t2851 = ct{283};
t2937 = ct{284};
t2942 = ct{285};
t2945 = ct{286};
t2950 = ct{287};
t2953 = ct{288};
t2955 = ct{289};
t2957 = ct{290};
t2963 = ct{291};
t2964 = ct{292};
t2975 = ct{293};
t2979 = ct{294};
t2984 = ct{295};
t2987 = ct{296};
t2990 = ct{297};
t2991 = ct{298};
t2993 = ct{299};
t2994 = ct{300};
t2998 = ct{301};
t3 = ct{302};
t30 = ct{303};
t3003 = ct{304};
t3004 = ct{305};
t3008 = ct{306};
t3009 = ct{307};
t3015 = ct{308};
t3017 = ct{309};
t3022 = ct{310};
t3027 = ct{311};
t3029 = ct{312};
t3030 = ct{313};
t3036 = ct{314};
t3043 = ct{315};
t3044 = ct{316};
t3045 = ct{317};
t3047 = ct{318};
t3049 = ct{319};
t3054 = ct{320};
t3055 = ct{321};
t3056 = ct{322};
t3057 = ct{323};
t3063 = ct{324};
t3064 = ct{325};
t3068 = ct{326};
t3072 = ct{327};
t3079 = ct{328};
t3080 = ct{329};
t3096 = ct{330};
t3097 = ct{331};
t31 = ct{332};
t3109 = ct{333};
t3117 = ct{334};
t3118 = ct{335};
t3121 = ct{336};
t3122 = ct{337};
t3128 = ct{338};
t3129 = ct{339};
t313 = ct{340};
t3130 = ct{341};
t3131 = ct{342};
t3132 = ct{343};
t3133 = ct{344};
t3134 = ct{345};
t3135 = ct{346};
t3139 = ct{347};
t314 = ct{348};
t3140 = ct{349};
t3141 = ct{350};
t3142 = ct{351};
t3144 = ct{352};
t3147 = ct{353};
t3153 = ct{354};
t3155 = ct{355};
t3156 = ct{356};
t3157 = ct{357};
t3158 = ct{358};
t3159 = ct{359};
t3160 = ct{360};
t3161 = ct{361};
t3162 = ct{362};
t3163 = ct{363};
t3164 = ct{364};
t3166 = ct{365};
t3170 = ct{366};
t3171 = ct{367};
t3172 = ct{368};
t3179 = ct{369};
t3180 = ct{370};
t3184 = ct{371};
t3186 = ct{372};
t3187 = ct{373};
t3188 = ct{374};
t3189 = ct{375};
t3190 = ct{376};
t3191 = ct{377};
t3193 = ct{378};
t3194 = ct{379};
t3196 = ct{380};
t3197 = ct{381};
t3198 = ct{382};
t3199 = ct{383};
t32 = ct{384};
t3200 = ct{385};
t3201 = ct{386};
t3206 = ct{387};
t3209 = ct{388};
t321 = ct{389};
t3210 = ct{390};
t3214 = ct{391};
t3218 = ct{392};
t3225 = ct{393};
t3226 = ct{394};
t3228 = ct{395};
t3229 = ct{396};
t3230 = ct{397};
t3231 = ct{398};
t3232 = ct{399};
t3235 = ct{400};
t3245 = ct{401};
t3246 = ct{402};
t3249 = ct{403};
t3250 = ct{404};
t3254 = ct{405};
t3256 = ct{406};
t3258 = ct{407};
t3259 = ct{408};
t326 = ct{409};
t3260 = ct{410};
t3261 = ct{411};
t3262 = ct{412};
t3263 = ct{413};
t3265 = ct{414};
t3266 = ct{415};
t3269 = ct{416};
t3270 = ct{417};
t3272 = ct{418};
t3276 = ct{419};
t3281 = ct{420};
t3283 = ct{421};
t329 = ct{422};
t3290 = ct{423};
t3291 = ct{424};
t3292 = ct{425};
t3295 = ct{426};
t3296 = ct{427};
t33 = ct{428};
t3300 = ct{429};
t3305 = ct{430};
t3306 = ct{431};
t3307 = ct{432};
t3308 = ct{433};
t3309 = ct{434};
t331 = ct{435};
t3313 = ct{436};
t3316 = ct{437};
t3318 = ct{438};
t3319 = ct{439};
t332 = ct{440};
t3324 = ct{441};
t3326 = ct{442};
t3327 = ct{443};
t3328 = ct{444};
t333 = ct{445};
t3330 = ct{446};
t3333 = ct{447};
t3334 = ct{448};
t3335 = ct{449};
t3336 = ct{450};
t3337 = ct{451};
t3341 = ct{452};
t3344 = ct{453};
t3347 = ct{454};
t3349 = ct{455};
t335 = ct{456};
t3353 = ct{457};
t3354 = ct{458};
t3357 = ct{459};
t3359 = ct{460};
t3360 = ct{461};
t3373 = ct{462};
t3376 = ct{463};
t3377 = ct{464};
t3379 = ct{465};
t3382 = ct{466};
t3384 = ct{467};
t3385 = ct{468};
t3386 = ct{469};
t339 = ct{470};
t3395 = ct{471};
t3399 = ct{472};
t34 = ct{473};
t3405 = ct{474};
t3409 = ct{475};
t3410 = ct{476};
t3412 = ct{477};
t3415 = ct{478};
t3417 = ct{479};
t3419 = ct{480};
t3420 = ct{481};
t3421 = ct{482};
t3422 = ct{483};
t3423 = ct{484};
t3424 = ct{485};
t3427 = ct{486};
t3428 = ct{487};
t3429 = ct{488};
t3430 = ct{489};
t3432 = ct{490};
t3433 = ct{491};
t3434 = ct{492};
t3435 = ct{493};
t3436 = ct{494};
t3437 = ct{495};
t3438 = ct{496};
t3440 = ct{497};
t3441 = ct{498};
t3442 = ct{499};
t3443 = ct{500};
t3444 = ct{501};
t3445 = ct{502};
t3446 = ct{503};
t3447 = ct{504};
t3449 = ct{505};
t3450 = ct{506};
t3451 = ct{507};
t3453 = ct{508};
t3455 = ct{509};
t3456 = ct{510};
t346 = ct{511};
t3465 = ct{512};
t3468 = ct{513};
t3470 = ct{514};
t3473 = ct{515};
t3475 = ct{516};
t3477 = ct{517};
t3479 = ct{518};
t3480 = ct{519};
t3481 = ct{520};
t3483 = ct{521};
t3484 = ct{522};
t3491 = ct{523};
t3493 = ct{524};
t3498 = ct{525};
t35 = ct{526};
t350 = ct{527};
t3503 = ct{528};
t3505 = ct{529};
t3512 = ct{530};
t3518 = ct{531};
t3522 = ct{532};
t3524 = ct{533};
t3526 = ct{534};
t3527 = ct{535};
t3528 = ct{536};
t3530 = ct{537};
t3531 = ct{538};
t3532 = ct{539};
t3533 = ct{540};
t3535 = ct{541};
t3539 = ct{542};
t354 = ct{543};
t3542 = ct{544};
t3543 = ct{545};
t3544 = ct{546};
t3547 = ct{547};
t3550 = ct{548};
t3558 = ct{549};
t3559 = ct{550};
t356 = ct{551};
t3560 = ct{552};
t3562 = ct{553};
t3563 = ct{554};
t3569 = ct{555};
t3570 = ct{556};
t3571 = ct{557};
t3576 = ct{558};
t3577 = ct{559};
t3578 = ct{560};
t358 = ct{561};
t3582 = ct{562};
t3585 = ct{563};
t3586 = ct{564};
t3587 = ct{565};
t3588 = ct{566};
t3589 = ct{567};
t359 = ct{568};
t3590 = ct{569};
t3593 = ct{570};
t3596 = ct{571};
t36 = ct{572};
t3600 = ct{573};
t3603 = ct{574};
t3616 = ct{575};
t3617 = ct{576};
t3618 = ct{577};
t3619 = ct{578};
t362 = ct{579};
t3620 = ct{580};
t3621 = ct{581};
t3622 = ct{582};
t3623 = ct{583};
t3624 = ct{584};
t3628 = ct{585};
t3631 = ct{586};
t3632 = ct{587};
t3633 = ct{588};
t3634 = ct{589};
t3635 = ct{590};
t3637 = ct{591};
t3638 = ct{592};
t3639 = ct{593};
t3641 = ct{594};
t3643 = ct{595};
t3649 = ct{596};
t3657 = ct{597};
t366 = ct{598};
t3663 = ct{599};
t3664 = ct{600};
t3665 = ct{601};
t3667 = ct{602};
t3669 = ct{603};
t3670 = ct{604};
t3672 = ct{605};
t3673 = ct{606};
t3674 = ct{607};
t3676 = ct{608};
t3678 = ct{609};
t3679 = ct{610};
t3680 = ct{611};
t3681 = ct{612};
t3682 = ct{613};
t3683 = ct{614};
t3684 = ct{615};
t3685 = ct{616};
t3686 = ct{617};
t3687 = ct{618};
t3689 = ct{619};
t3690 = ct{620};
t3693 = ct{621};
t3694 = ct{622};
t3699 = ct{623};
t3703 = ct{624};
t3705 = ct{625};
t3706 = ct{626};
t3708 = ct{627};
t3709 = ct{628};
t3712 = ct{629};
t3713 = ct{630};
t3714 = ct{631};
t3715 = ct{632};
t3716 = ct{633};
t3718 = ct{634};
t372 = ct{635};
t3723 = ct{636};
t3724 = ct{637};
t3729 = ct{638};
t3732 = ct{639};
t3734 = ct{640};
t3735 = ct{641};
t3736 = ct{642};
t3737 = ct{643};
t3744 = ct{644};
t3745 = ct{645};
t3746 = ct{646};
t3748 = ct{647};
t3749 = ct{648};
t3751 = ct{649};
t3753 = ct{650};
t3755 = ct{651};
t3756 = ct{652};
t3757 = ct{653};
t3758 = ct{654};
t3759 = ct{655};
t3760 = ct{656};
t3762 = ct{657};
t3763 = ct{658};
t3764 = ct{659};
t3765 = ct{660};
t3766 = ct{661};
t3767 = ct{662};
t3768 = ct{663};
t3769 = ct{664};
t3770 = ct{665};
t3771 = ct{666};
t3772 = ct{667};
t3774 = ct{668};
t3775 = ct{669};
t3776 = ct{670};
t3778 = ct{671};
t3779 = ct{672};
t378 = ct{673};
t3782 = ct{674};
t3783 = ct{675};
t3784 = ct{676};
t3790 = ct{677};
t3791 = ct{678};
t3794 = ct{679};
t3795 = ct{680};
t3797 = ct{681};
t3798 = ct{682};
t3799 = ct{683};
t38 = ct{684};
t380 = ct{685};
t3801 = ct{686};
t3803 = ct{687};
t3804 = ct{688};
t3806 = ct{689};
t3811 = ct{690};
t3814 = ct{691};
t3815 = ct{692};
t3816 = ct{693};
t3817 = ct{694};
t3819 = ct{695};
t382 = ct{696};
t3821 = ct{697};
t3822 = ct{698};
t3826 = ct{699};
t3827 = ct{700};
t3828 = ct{701};
t3833 = ct{702};
t3834 = ct{703};
t3844 = ct{704};
t3845 = ct{705};
t3847 = ct{706};
t3849 = ct{707};
t3850 = ct{708};
t3860 = ct{709};
t3861 = ct{710};
t3862 = ct{711};
t3863 = ct{712};
t3865 = ct{713};
t3866 = ct{714};
t3869 = ct{715};
t387 = ct{716};
t3870 = ct{717};
t3871 = ct{718};
t3872 = ct{719};
t3875 = ct{720};
t3876 = ct{721};
t3877 = ct{722};
t3880 = ct{723};
t3882 = ct{724};
t3891 = ct{725};
t3892 = ct{726};
t3893 = ct{727};
t3898 = ct{728};
t39 = ct{729};
t3901 = ct{730};
t3904 = ct{731};
t3910 = ct{732};
t3916 = ct{733};
t3918 = ct{734};
t3922 = ct{735};
t3928 = ct{736};
t3934 = ct{737};
t3940 = ct{738};
t3941 = ct{739};
t3942 = ct{740};
t3943 = ct{741};
t3945 = ct{742};
t3946 = ct{743};
t3949 = ct{744};
t3951 = ct{745};
t3954 = ct{746};
t3957 = ct{747};
t3958 = ct{748};
t3959 = ct{749};
t3962 = ct{750};
t3964 = ct{751};
t3965 = ct{752};
t3967 = ct{753};
t3968 = ct{754};
t3972 = ct{755};
t3973 = ct{756};
t3974 = ct{757};
t3976 = ct{758};
t3980 = ct{759};
t3984 = ct{760};
t3985 = ct{761};
t3992 = ct{762};
t3996 = ct{763};
t4 = ct{764};
t4007 = ct{765};
t4011 = ct{766};
t4012 = ct{767};
t4013 = ct{768};
t4014 = ct{769};
t4015 = ct{770};
t4016 = ct{771};
t4018 = ct{772};
t4027 = ct{773};
t4062 = ct{774};
t4071 = ct{775};
t4072 = ct{776};
t4075 = ct{777};
t4076 = ct{778};
t4077 = ct{779};
t4080 = ct{780};
t410 = ct{781};
t4106 = ct{782};
t4108 = ct{783};
t4109 = ct{784};
t4113 = ct{785};
t4119 = ct{786};
t4120 = ct{787};
t4122 = ct{788};
t4125 = ct{789};
t4127 = ct{790};
t4130 = ct{791};
t4133 = ct{792};
t4134 = ct{793};
t4149 = ct{794};
t4150 = ct{795};
t4152 = ct{796};
t4154 = ct{797};
t4155 = ct{798};
t4160 = ct{799};
t4163 = ct{800};
t4168 = ct{801};
t4173 = ct{802};
t4175 = ct{803};
t4178 = ct{804};
t4179 = ct{805};
t4184 = ct{806};
t4189 = ct{807};
t4190 = ct{808};
t4196 = ct{809};
t42 = ct{810};
t4200 = ct{811};
t4201 = ct{812};
t4202 = ct{813};
t4203 = ct{814};
t4205 = ct{815};
t4207 = ct{816};
t4208 = ct{817};
t4217 = ct{818};
t4219 = ct{819};
t4220 = ct{820};
t4221 = ct{821};
t4226 = ct{822};
t4227 = ct{823};
t4228 = ct{824};
t4230 = ct{825};
t4231 = ct{826};
t4233 = ct{827};
t4234 = ct{828};
t4235 = ct{829};
t4236 = ct{830};
t4237 = ct{831};
t4238 = ct{832};
t4239 = ct{833};
t4240 = ct{834};
t4242 = ct{835};
t4243 = ct{836};
t4244 = ct{837};
t4245 = ct{838};
t4246 = ct{839};
t4247 = ct{840};
t4248 = ct{841};
t4249 = ct{842};
t4250 = ct{843};
t4251 = ct{844};
t4252 = ct{845};
t4253 = ct{846};
t4254 = ct{847};
t4255 = ct{848};
t4256 = ct{849};
t4257 = ct{850};
t4259 = ct{851};
t4260 = ct{852};
t4261 = ct{853};
t4262 = ct{854};
t4263 = ct{855};
t4264 = ct{856};
t4266 = ct{857};
t4267 = ct{858};
t4268 = ct{859};
t4274 = ct{860};
t4276 = ct{861};
t4277 = ct{862};
t4279 = ct{863};
t4280 = ct{864};
t4281 = ct{865};
t4285 = ct{866};
t4287 = ct{867};
t429 = ct{868};
t4291 = ct{869};
t4292 = ct{870};
t4295 = ct{871};
t4296 = ct{872};
t4297 = ct{873};
t4298 = ct{874};
t43 = ct{875};
t4304 = ct{876};
t4306 = ct{877};
t4307 = ct{878};
t4308 = ct{879};
t4310 = ct{880};
t4311 = ct{881};
t4313 = ct{882};
t4314 = ct{883};
t4315 = ct{884};
t4316 = ct{885};
t4321 = ct{886};
t4322 = ct{887};
t4323 = ct{888};
t4324 = ct{889};
t4354 = ct{890};
t4356 = ct{891};
t4358 = ct{892};
t4361 = ct{893};
t4362 = ct{894};
t4363 = ct{895};
t4369 = ct{896};
t4370 = ct{897};
t4373 = ct{898};
t4374 = ct{899};
t4376 = ct{900};
t4377 = ct{901};
t4378 = ct{902};
t4379 = ct{903};
t4380 = ct{904};
t4382 = ct{905};
t4386 = ct{906};
t4387 = ct{907};
t4388 = ct{908};
t4389 = ct{909};
t4391 = ct{910};
t4392 = ct{911};
t4393 = ct{912};
t4394 = ct{913};
t4396 = ct{914};
t4400 = ct{915};
t4404 = ct{916};
t4405 = ct{917};
t4406 = ct{918};
t4409 = ct{919};
t4410 = ct{920};
t4411 = ct{921};
t4412 = ct{922};
t4413 = ct{923};
t4415 = ct{924};
t4421 = ct{925};
t4424 = ct{926};
t4427 = ct{927};
t4428 = ct{928};
t4429 = ct{929};
t4432 = ct{930};
t4434 = ct{931};
t4436 = ct{932};
t4437 = ct{933};
t4438 = ct{934};
t4439 = ct{935};
t4440 = ct{936};
t4444 = ct{937};
t4447 = ct{938};
t4458 = ct{939};
t4460 = ct{940};
t4461 = ct{941};
t4464 = ct{942};
t4473 = ct{943};
t4475 = ct{944};
t4491 = ct{945};
t4496 = ct{946};
t4498 = ct{947};
t4499 = ct{948};
t4500 = ct{949};
t4501 = ct{950};
t4503 = ct{951};
t4504 = ct{952};
t4505 = ct{953};
t4506 = ct{954};
t4507 = ct{955};
t4508 = ct{956};
t4510 = ct{957};
t4511 = ct{958};
t4513 = ct{959};
t4514 = ct{960};
t4515 = ct{961};
t4516 = ct{962};
t4517 = ct{963};
t4519 = ct{964};
t4520 = ct{965};
t4521 = ct{966};
t4522 = ct{967};
t4525 = ct{968};
t4526 = ct{969};
t4527 = ct{970};
t4528 = ct{971};
t4530 = ct{972};
t4531 = ct{973};
t4532 = ct{974};
t4535 = ct{975};
t4536 = ct{976};
t4537 = ct{977};
t4538 = ct{978};
t4539 = ct{979};
t4543 = ct{980};
t4545 = ct{981};
t4546 = ct{982};
t4547 = ct{983};
t4548 = ct{984};
t4550 = ct{985};
t4552 = ct{986};
t4554 = ct{987};
t4555 = ct{988};
t4556 = ct{989};
t4557 = ct{990};
t4558 = ct{991};
t4559 = ct{992};
t4560 = ct{993};
t4561 = ct{994};
t4562 = ct{995};
t4563 = ct{996};
t4564 = ct{997};
t4566 = ct{998};
t4567 = ct{999};
t4568 = ct{1000};
t4569 = ct{1001};
t4570 = ct{1002};
t4571 = ct{1003};
t4572 = ct{1004};
t4576 = ct{1005};
t4577 = ct{1006};
t4578 = ct{1007};
t4579 = ct{1008};
t4581 = ct{1009};
t4582 = ct{1010};
t4583 = ct{1011};
t4584 = ct{1012};
t4586 = ct{1013};
t4587 = ct{1014};
t4588 = ct{1015};
t4589 = ct{1016};
t4591 = ct{1017};
t4593 = ct{1018};
t4594 = ct{1019};
t4595 = ct{1020};
t4597 = ct{1021};
t4598 = ct{1022};
t4599 = ct{1023};
t46 = ct{1024};
t4602 = ct{1025};
t4604 = ct{1026};
t4606 = ct{1027};
t4607 = ct{1028};
t4609 = ct{1029};
t4610 = ct{1030};
t4611 = ct{1031};
t4612 = ct{1032};
t4613 = ct{1033};
t4614 = ct{1034};
t4615 = ct{1035};
t4617 = ct{1036};
t4620 = ct{1037};
t4623 = ct{1038};
t4625 = ct{1039};
t4626 = ct{1040};
t4627 = ct{1041};
t4628 = ct{1042};
t4629 = ct{1043};
t4631 = ct{1044};
t4633 = ct{1045};
t4634 = ct{1046};
t4635 = ct{1047};
t4640 = ct{1048};
t4641 = ct{1049};
t4642 = ct{1050};
t4644 = ct{1051};
t4645 = ct{1052};
t4647 = ct{1053};
t4649 = ct{1054};
t4650 = ct{1055};
t4651 = ct{1056};
t4652 = ct{1057};
t4655 = ct{1058};
t4658 = ct{1059};
t4659 = ct{1060};
t4661 = ct{1061};
t4663 = ct{1062};
t4664 = ct{1063};
t4666 = ct{1064};
t4667 = ct{1065};
t4669 = ct{1066};
t4672 = ct{1067};
t4674 = ct{1068};
t4676 = ct{1069};
t4678 = ct{1070};
t4679 = ct{1071};
t4680 = ct{1072};
t4682 = ct{1073};
t4683 = ct{1074};
t4685 = ct{1075};
t4686 = ct{1076};
t4688 = ct{1077};
t4699 = ct{1078};
t47 = ct{1079};
t4702 = ct{1080};
t4703 = ct{1081};
t4704 = ct{1082};
t4705 = ct{1083};
t4706 = ct{1084};
t4708 = ct{1085};
t4709 = ct{1086};
t4712 = ct{1087};
t4713 = ct{1088};
t4714 = ct{1089};
t4716 = ct{1090};
t4718 = ct{1091};
t4719 = ct{1092};
t4720 = ct{1093};
t4721 = ct{1094};
t4725 = ct{1095};
t4727 = ct{1096};
t4728 = ct{1097};
t4729 = ct{1098};
t4732 = ct{1099};
t4733 = ct{1100};
t4735 = ct{1101};
t4737 = ct{1102};
t4738 = ct{1103};
t4739 = ct{1104};
t4741 = ct{1105};
t4742 = ct{1106};
t4743 = ct{1107};
t4744 = ct{1108};
t4748 = ct{1109};
t4751 = ct{1110};
t4752 = ct{1111};
t4753 = ct{1112};
t4755 = ct{1113};
t4757 = ct{1114};
t4758 = ct{1115};
t4759 = ct{1116};
t4760 = ct{1117};
t4762 = ct{1118};
t4765 = ct{1119};
t4766 = ct{1120};
t4767 = ct{1121};
t4769 = ct{1122};
t4770 = ct{1123};
t4772 = ct{1124};
t4774 = ct{1125};
t4777 = ct{1126};
t4780 = ct{1127};
t4785 = ct{1128};
t4786 = ct{1129};
t4787 = ct{1130};
t4788 = ct{1131};
t4789 = ct{1132};
t4790 = ct{1133};
t4791 = ct{1134};
t4792 = ct{1135};
t4793 = ct{1136};
t4794 = ct{1137};
t4795 = ct{1138};
t4796 = ct{1139};
t4798 = ct{1140};
t4799 = ct{1141};
t4800 = ct{1142};
t4801 = ct{1143};
t4805 = ct{1144};
t4809 = ct{1145};
t4814 = ct{1146};
t4816 = ct{1147};
t4817 = ct{1148};
t4818 = ct{1149};
t4819 = ct{1150};
t4822 = ct{1151};
t4823 = ct{1152};
t4824 = ct{1153};
t4825 = ct{1154};
t4826 = ct{1155};
t4829 = ct{1156};
t4832 = ct{1157};
t4833 = ct{1158};
t4835 = ct{1159};
t4836 = ct{1160};
t4839 = ct{1161};
t4840 = ct{1162};
t4842 = ct{1163};
t4843 = ct{1164};
t4845 = ct{1165};
t4847 = ct{1166};
t4848 = ct{1167};
t4849 = ct{1168};
t4850 = ct{1169};
t4851 = ct{1170};
t4852 = ct{1171};
t4853 = ct{1172};
t4856 = ct{1173};
t4857 = ct{1174};
t4858 = ct{1175};
t4859 = ct{1176};
t4860 = ct{1177};
t4863 = ct{1178};
t4864 = ct{1179};
t4865 = ct{1180};
t4866 = ct{1181};
t4867 = ct{1182};
t4868 = ct{1183};
t4869 = ct{1184};
t4870 = ct{1185};
t4871 = ct{1186};
t4872 = ct{1187};
t4873 = ct{1188};
t4874 = ct{1189};
t4875 = ct{1190};
t4876 = ct{1191};
t4877 = ct{1192};
t4880 = ct{1193};
t4881 = ct{1194};
t4882 = ct{1195};
t4883 = ct{1196};
t4884 = ct{1197};
t4885 = ct{1198};
t4886 = ct{1199};
t4887 = ct{1200};
t4888 = ct{1201};
t4890 = ct{1202};
t4892 = ct{1203};
t4893 = ct{1204};
t4894 = ct{1205};
t4895 = ct{1206};
t4896 = ct{1207};
t4897 = ct{1208};
t4898 = ct{1209};
t4899 = ct{1210};
t4900 = ct{1211};
t4902 = ct{1212};
t4904 = ct{1213};
t4905 = ct{1214};
t4906 = ct{1215};
t4911 = ct{1216};
t4912 = ct{1217};
t4913 = ct{1218};
t4914 = ct{1219};
t4916 = ct{1220};
t4917 = ct{1221};
t4918 = ct{1222};
t4919 = ct{1223};
t4921 = ct{1224};
t4922 = ct{1225};
t4924 = ct{1226};
t4925 = ct{1227};
t4927 = ct{1228};
t4929 = ct{1229};
t4931 = ct{1230};
t4932 = ct{1231};
t4950 = ct{1232};
t4952 = ct{1233};
t4953 = ct{1234};
t4954 = ct{1235};
t4955 = ct{1236};
t4957 = ct{1237};
t4961 = ct{1238};
t4962 = ct{1239};
t4963 = ct{1240};
t4965 = ct{1241};
t4968 = ct{1242};
t4969 = ct{1243};
t4970 = ct{1244};
t4973 = ct{1245};
t4974 = ct{1246};
t4975 = ct{1247};
t4976 = ct{1248};
t4977 = ct{1249};
t4978 = ct{1250};
t4979 = ct{1251};
t4982 = ct{1252};
t4983 = ct{1253};
t4984 = ct{1254};
t4985 = ct{1255};
t4986 = ct{1256};
t4987 = ct{1257};
t4992 = ct{1258};
t4994 = ct{1259};
t4995 = ct{1260};
t4996 = ct{1261};
t4998 = ct{1262};
t5 = ct{1263};
t50 = ct{1264};
t5000 = ct{1265};
t5001 = ct{1266};
t5002 = ct{1267};
t5003 = ct{1268};
t5004 = ct{1269};
t5005 = ct{1270};
t5007 = ct{1271};
t5010 = ct{1272};
t5012 = ct{1273};
t5013 = ct{1274};
t5014 = ct{1275};
t5015 = ct{1276};
t5017 = ct{1277};
t5021 = ct{1278};
t5022 = ct{1279};
t5023 = ct{1280};
t5025 = ct{1281};
t5026 = ct{1282};
t5027 = ct{1283};
t5028 = ct{1284};
t5030 = ct{1285};
t5031 = ct{1286};
t5032 = ct{1287};
t5033 = ct{1288};
t5034 = ct{1289};
t5035 = ct{1290};
t5036 = ct{1291};
t5038 = ct{1292};
t5039 = ct{1293};
t5040 = ct{1294};
t5041 = ct{1295};
t5042 = ct{1296};
t5047 = ct{1297};
t5048 = ct{1298};
t5049 = ct{1299};
t5051 = ct{1300};
t5052 = ct{1301};
t5053 = ct{1302};
t5054 = ct{1303};
t5055 = ct{1304};
t5056 = ct{1305};
t5057 = ct{1306};
t5058 = ct{1307};
t5059 = ct{1308};
t5061 = ct{1309};
t5062 = ct{1310};
t5063 = ct{1311};
t5064 = ct{1312};
t5066 = ct{1313};
t5067 = ct{1314};
t5068 = ct{1315};
t5069 = ct{1316};
t5070 = ct{1317};
t5071 = ct{1318};
t5073 = ct{1319};
t5074 = ct{1320};
t5075 = ct{1321};
t5076 = ct{1322};
t5077 = ct{1323};
t5092 = ct{1324};
t5094 = ct{1325};
t5096 = ct{1326};
t5097 = ct{1327};
t5098 = ct{1328};
t5103 = ct{1329};
t5104 = ct{1330};
t5105 = ct{1331};
t5106 = ct{1332};
t5108 = ct{1333};
t5109 = ct{1334};
t5111 = ct{1335};
t5112 = ct{1336};
t5113 = ct{1337};
t5114 = ct{1338};
t5115 = ct{1339};
t5116 = ct{1340};
t5117 = ct{1341};
t5118 = ct{1342};
t5119 = ct{1343};
t5121 = ct{1344};
t5123 = ct{1345};
t5124 = ct{1346};
t5126 = ct{1347};
t5127 = ct{1348};
t5128 = ct{1349};
t5130 = ct{1350};
t5131 = ct{1351};
t5144 = ct{1352};
t5145 = ct{1353};
t5146 = ct{1354};
t5147 = ct{1355};
t5148 = ct{1356};
t5149 = ct{1357};
t5150 = ct{1358};
t5151 = ct{1359};
t5152 = ct{1360};
t5153 = ct{1361};
t5155 = ct{1362};
t5156 = ct{1363};
t5157 = ct{1364};
t5158 = ct{1365};
t5161 = ct{1366};
t5162 = ct{1367};
t5164 = ct{1368};
t5165 = ct{1369};
t5166 = ct{1370};
t5169 = ct{1371};
t5175 = ct{1372};
t5176 = ct{1373};
t5177 = ct{1374};
t5178 = ct{1375};
t5179 = ct{1376};
t5180 = ct{1377};
t5184 = ct{1378};
t5189 = ct{1379};
t5190 = ct{1380};
t5191 = ct{1381};
t5192 = ct{1382};
t5193 = ct{1383};
t5194 = ct{1384};
t5195 = ct{1385};
t5196 = ct{1386};
t5198 = ct{1387};
t5201 = ct{1388};
t5202 = ct{1389};
t5203 = ct{1390};
t5204 = ct{1391};
t5206 = ct{1392};
t5207 = ct{1393};
t5208 = ct{1394};
t5209 = ct{1395};
t5210 = ct{1396};
t5212 = ct{1397};
t5213 = ct{1398};
t5214 = ct{1399};
t5215 = ct{1400};
t5216 = ct{1401};
t5217 = ct{1402};
t5219 = ct{1403};
t5220 = ct{1404};
t5221 = ct{1405};
t5222 = ct{1406};
t5223 = ct{1407};
t5224 = ct{1408};
t5225 = ct{1409};
t5226 = ct{1410};
t5227 = ct{1411};
t5228 = ct{1412};
t5229 = ct{1413};
t5230 = ct{1414};
t5231 = ct{1415};
t5232 = ct{1416};
t5233 = ct{1417};
t5234 = ct{1418};
t5235 = ct{1419};
t5236 = ct{1420};
t5237 = ct{1421};
t5238 = ct{1422};
t5239 = ct{1423};
t5240 = ct{1424};
t5241 = ct{1425};
t5242 = ct{1426};
t5243 = ct{1427};
t5244 = ct{1428};
t5245 = ct{1429};
t5246 = ct{1430};
t5247 = ct{1431};
t5248 = ct{1432};
t5250 = ct{1433};
t5252 = ct{1434};
t5254 = ct{1435};
t5255 = ct{1436};
t5257 = ct{1437};
t5258 = ct{1438};
t5260 = ct{1439};
t5261 = ct{1440};
t5262 = ct{1441};
t5268 = ct{1442};
t5269 = ct{1443};
t5270 = ct{1444};
t5271 = ct{1445};
t5272 = ct{1446};
t5273 = ct{1447};
t5274 = ct{1448};
t5275 = ct{1449};
t5276 = ct{1450};
t5277 = ct{1451};
t5278 = ct{1452};
t5279 = ct{1453};
t5280 = ct{1454};
t5281 = ct{1455};
t5282 = ct{1456};
t5284 = ct{1457};
t5285 = ct{1458};
t5286 = ct{1459};
t5288 = ct{1460};
t5289 = ct{1461};
t5291 = ct{1462};
t5293 = ct{1463};
t5295 = ct{1464};
t5300 = ct{1465};
t5301 = ct{1466};
t5302 = ct{1467};
t5304 = ct{1468};
t5306 = ct{1469};
t5307 = ct{1470};
t5308 = ct{1471};
t5314 = ct{1472};
t5316 = ct{1473};
t5317 = ct{1474};
t5320 = ct{1475};
t5321 = ct{1476};
t5322 = ct{1477};
t5328 = ct{1478};
t5330 = ct{1479};
t5331 = ct{1480};
t5332 = ct{1481};
t5333 = ct{1482};
t5335 = ct{1483};
t5336 = ct{1484};
t5337 = ct{1485};
t5338 = ct{1486};
t5339 = ct{1487};
t5340 = ct{1488};
t5342 = ct{1489};
t5344 = ct{1490};
t5345 = ct{1491};
t5346 = ct{1492};
t5347 = ct{1493};
t5348 = ct{1494};
t5349 = ct{1495};
t5350 = ct{1496};
t5351 = ct{1497};
t5354 = ct{1498};
t5356 = ct{1499};
t5357 = ct{1500};
t5358 = ct{1501};
t5359 = ct{1502};
t5360 = ct{1503};
t5361 = ct{1504};
t5362 = ct{1505};
t5365 = ct{1506};
t5367 = ct{1507};
t5369 = ct{1508};
t5370 = ct{1509};
t5371 = ct{1510};
t5375 = ct{1511};
t5377 = ct{1512};
t5379 = ct{1513};
t5380 = ct{1514};
t5381 = ct{1515};
t5383 = ct{1516};
t5384 = ct{1517};
t5385 = ct{1518};
t5386 = ct{1519};
t5387 = ct{1520};
t5388 = ct{1521};
t5389 = ct{1522};
t5390 = ct{1523};
t5391 = ct{1524};
t5392 = ct{1525};
t5393 = ct{1526};
t5394 = ct{1527};
t5395 = ct{1528};
t5396 = ct{1529};
t5397 = ct{1530};
t5399 = ct{1531};
t5402 = ct{1532};
t5403 = ct{1533};
t5405 = ct{1534};
t5407 = ct{1535};
t5408 = ct{1536};
t5409 = ct{1537};
t5411 = ct{1538};
t5412 = ct{1539};
t5413 = ct{1540};
t5416 = ct{1541};
t5418 = ct{1542};
t5419 = ct{1543};
t5420 = ct{1544};
t5426 = ct{1545};
t5427 = ct{1546};
t5428 = ct{1547};
t5429 = ct{1548};
t5433 = ct{1549};
t5434 = ct{1550};
t5440 = ct{1551};
t5441 = ct{1552};
t5443 = ct{1553};
t5444 = ct{1554};
t5445 = ct{1555};
t5446 = ct{1556};
t5447 = ct{1557};
t5448 = ct{1558};
t5449 = ct{1559};
t5451 = ct{1560};
t5452 = ct{1561};
t5453 = ct{1562};
t5454 = ct{1563};
t5455 = ct{1564};
t5457 = ct{1565};
t5458 = ct{1566};
t5459 = ct{1567};
t5461 = ct{1568};
t5462 = ct{1569};
t5465 = ct{1570};
t5467 = ct{1571};
t5468 = ct{1572};
t5469 = ct{1573};
t5472 = ct{1574};
t5473 = ct{1575};
t5474 = ct{1576};
t5476 = ct{1577};
t5477 = ct{1578};
t5480 = ct{1579};
t5481 = ct{1580};
t5482 = ct{1581};
t5483 = ct{1582};
t5484 = ct{1583};
t5485 = ct{1584};
t5486 = ct{1585};
t5487 = ct{1586};
t5488 = ct{1587};
t5489 = ct{1588};
t5490 = ct{1589};
t5491 = ct{1590};
t5492 = ct{1591};
t5493 = ct{1592};
t5494 = ct{1593};
t5496 = ct{1594};
t5498 = ct{1595};
t5499 = ct{1596};
t5500 = ct{1597};
t5503 = ct{1598};
t5504 = ct{1599};
t5505 = ct{1600};
t5506 = ct{1601};
t5509 = ct{1602};
t5514 = ct{1603};
t5515 = ct{1604};
t5516 = ct{1605};
t5517 = ct{1606};
t5518 = ct{1607};
t5520 = ct{1608};
t5521 = ct{1609};
t5522 = ct{1610};
t5523 = ct{1611};
t5524 = ct{1612};
t5525 = ct{1613};
t5526 = ct{1614};
t5528 = ct{1615};
t5531 = ct{1616};
t5532 = ct{1617};
t5533 = ct{1618};
t5534 = ct{1619};
t5535 = ct{1620};
t5536 = ct{1621};
t5537 = ct{1622};
t5538 = ct{1623};
t5539 = ct{1624};
t5541 = ct{1625};
t5542 = ct{1626};
t5543 = ct{1627};
t5544 = ct{1628};
t5545 = ct{1629};
t5546 = ct{1630};
t5547 = ct{1631};
t5548 = ct{1632};
t5550 = ct{1633};
t5551 = ct{1634};
t5552 = ct{1635};
t5553 = ct{1636};
t5554 = ct{1637};
t5556 = ct{1638};
t5557 = ct{1639};
t5558 = ct{1640};
t5559 = ct{1641};
t5561 = ct{1642};
t5564 = ct{1643};
t5566 = ct{1644};
t5569 = ct{1645};
t5570 = ct{1646};
t5573 = ct{1647};
t5574 = ct{1648};
t5575 = ct{1649};
t5576 = ct{1650};
t5577 = ct{1651};
t5578 = ct{1652};
t5579 = ct{1653};
t5580 = ct{1654};
t5581 = ct{1655};
t5582 = ct{1656};
t5583 = ct{1657};
t5584 = ct{1658};
t5587 = ct{1659};
t5588 = ct{1660};
t5589 = ct{1661};
t5592 = ct{1662};
t5593 = ct{1663};
t5594 = ct{1664};
t5595 = ct{1665};
t5597 = ct{1666};
t5598 = ct{1667};
t56 = ct{1668};
t5600 = ct{1669};
t5601 = ct{1670};
t5602 = ct{1671};
t5603 = ct{1672};
t5604 = ct{1673};
t5605 = ct{1674};
t5606 = ct{1675};
t5609 = ct{1676};
t5617 = ct{1677};
t5618 = ct{1678};
t5619 = ct{1679};
t5620 = ct{1680};
t5621 = ct{1681};
t5622 = ct{1682};
t5626 = ct{1683};
t5627 = ct{1684};
t5628 = ct{1685};
t5631 = ct{1686};
t5632 = ct{1687};
t5635 = ct{1688};
t5639 = ct{1689};
t5640 = ct{1690};
t5642 = ct{1691};
t5643 = ct{1692};
t5658 = ct{1693};
t5659 = ct{1694};
t5660 = ct{1695};
t5661 = ct{1696};
t5662 = ct{1697};
t5663 = ct{1698};
t5664 = ct{1699};
t5666 = ct{1700};
t5667 = ct{1701};
t5670 = ct{1702};
t5671 = ct{1703};
t5674 = ct{1704};
t5675 = ct{1705};
t5676 = ct{1706};
t5678 = ct{1707};
t5679 = ct{1708};
t5681 = ct{1709};
t5682 = ct{1710};
t5685 = ct{1711};
t5687 = ct{1712};
t5689 = ct{1713};
t5690 = ct{1714};
t5691 = ct{1715};
t5693 = ct{1716};
t5694 = ct{1717};
t5695 = ct{1718};
t5699 = ct{1719};
t5700 = ct{1720};
t5701 = ct{1721};
t5702 = ct{1722};
t5703 = ct{1723};
t5705 = ct{1724};
t5706 = ct{1725};
t5707 = ct{1726};
t5708 = ct{1727};
t5709 = ct{1728};
t5711 = ct{1729};
t5712 = ct{1730};
t5717 = ct{1731};
t5718 = ct{1732};
t5720 = ct{1733};
t5721 = ct{1734};
t5722 = ct{1735};
t5723 = ct{1736};
t5725 = ct{1737};
t5726 = ct{1738};
t5727 = ct{1739};
t5728 = ct{1740};
t5730 = ct{1741};
t5731 = ct{1742};
t5733 = ct{1743};
t5735 = ct{1744};
t5737 = ct{1745};
t5739 = ct{1746};
t5740 = ct{1747};
t5741 = ct{1748};
t5742 = ct{1749};
t5748 = ct{1750};
t5749 = ct{1751};
t5750 = ct{1752};
t5751 = ct{1753};
t5752 = ct{1754};
t5753 = ct{1755};
t5760 = ct{1756};
t5761 = ct{1757};
t5764 = ct{1758};
t5765 = ct{1759};
t5766 = ct{1760};
t5767 = ct{1761};
t5768 = ct{1762};
t5770 = ct{1763};
t5775 = ct{1764};
t5779 = ct{1765};
t5782 = ct{1766};
t5785 = ct{1767};
t5786 = ct{1768};
t5791 = ct{1769};
t5792 = ct{1770};
t5793 = ct{1771};
t5794 = ct{1772};
t5796 = ct{1773};
t58 = ct{1774};
t5804 = ct{1775};
t5805 = ct{1776};
t5806 = ct{1777};
t5807 = ct{1778};
t5817 = ct{1779};
t5826 = ct{1780};
t5827 = ct{1781};
t5828 = ct{1782};
t5832 = ct{1783};
t5835 = ct{1784};
t5839 = ct{1785};
t5840 = ct{1786};
t5843 = ct{1787};
t5846 = ct{1788};
t5852 = ct{1789};
t5853 = ct{1790};
t5854 = ct{1791};
t5855 = ct{1792};
t5857 = ct{1793};
t5858 = ct{1794};
t5859 = ct{1795};
t5860 = ct{1796};
t5861 = ct{1797};
t5862 = ct{1798};
t5864 = ct{1799};
t5866 = ct{1800};
t5867 = ct{1801};
t5868 = ct{1802};
t5871 = ct{1803};
t5876 = ct{1804};
t5879 = ct{1805};
t5890 = ct{1806};
t5891 = ct{1807};
t5894 = ct{1808};
t5896 = ct{1809};
t5899 = ct{1810};
t59 = ct{1811};
t5900 = ct{1812};
t5901 = ct{1813};
t5904 = ct{1814};
t5907 = ct{1815};
t5908 = ct{1816};
t5910 = ct{1817};
t5911 = ct{1818};
t5912 = ct{1819};
t5913 = ct{1820};
t5914 = ct{1821};
t5916 = ct{1822};
t5922 = ct{1823};
t5923 = ct{1824};
t5930 = ct{1825};
t5932 = ct{1826};
t5933 = ct{1827};
t5941 = ct{1828};
t5943 = ct{1829};
t5944 = ct{1830};
t5951 = ct{1831};
t5952 = ct{1832};
t5953 = ct{1833};
t5954 = ct{1834};
t5958 = ct{1835};
t5961 = ct{1836};
t5966 = ct{1837};
t5969 = ct{1838};
t5970 = ct{1839};
t5975 = ct{1840};
t5977 = ct{1841};
t5991 = ct{1842};
t5992 = ct{1843};
t5994 = ct{1844};
t5996 = ct{1845};
t5998 = ct{1846};
t5999 = ct{1847};
t6 = ct{1848};
t60 = ct{1849};
t6000 = ct{1850};
t6002 = ct{1851};
t6004 = ct{1852};
t6009 = ct{1853};
t6010 = ct{1854};
t6012 = ct{1855};
t6014 = ct{1856};
t6015 = ct{1857};
t6016 = ct{1858};
t6017 = ct{1859};
t6018 = ct{1860};
t6019 = ct{1861};
t6020 = ct{1862};
t6021 = ct{1863};
t6028 = ct{1864};
t6030 = ct{1865};
t6031 = ct{1866};
t6034 = ct{1867};
t6038 = ct{1868};
t6049 = ct{1869};
t6050 = ct{1870};
t6051 = ct{1871};
t6054 = ct{1872};
t6057 = ct{1873};
t6058 = ct{1874};
t6059 = ct{1875};
t6060 = ct{1876};
t6062 = ct{1877};
t6064 = ct{1878};
t6066 = ct{1879};
t6067 = ct{1880};
t6075 = ct{1881};
t6076 = ct{1882};
t6085 = ct{1883};
t6087 = ct{1884};
t6091 = ct{1885};
t6092 = ct{1886};
t6095 = ct{1887};
t6096 = ct{1888};
t6101 = ct{1889};
t6112 = ct{1890};
t6135 = ct{1891};
t6137 = ct{1892};
t6143 = ct{1893};
t6144 = ct{1894};
t6147 = ct{1895};
t6151 = ct{1896};
t6153 = ct{1897};
t6156 = ct{1898};
t6162 = ct{1899};
t6169 = ct{1900};
t6183 = ct{1901};
t6184 = ct{1902};
t6185 = ct{1903};
t6198 = ct{1904};
t6199 = ct{1905};
t6200 = ct{1906};
t6206 = ct{1907};
t6207 = ct{1908};
t6209 = ct{1909};
t6219 = ct{1910};
t6221 = ct{1911};
t6232 = ct{1912};
t6238 = ct{1913};
t6247 = ct{1914};
t6253 = ct{1915};
t6257 = ct{1916};
t6293 = ct{1917};
t6302 = ct{1918};
t6303 = ct{1919};
t6313 = ct{1920};
t6317 = ct{1921};
t6321 = ct{1922};
t6322 = ct{1923};
t6323 = ct{1924};
t6339 = ct{1925};
t6341 = ct{1926};
t6343 = ct{1927};
t6344 = ct{1928};
t6356 = ct{1929};
t6366 = ct{1930};
t6367 = ct{1931};
t6375 = ct{1932};
t638 = ct{1933};
t6387 = ct{1934};
t6388 = ct{1935};
t640 = ct{1936};
t6406 = ct{1937};
t6414 = ct{1938};
t642 = ct{1939};
t643 = ct{1940};
t6442 = ct{1941};
t6450 = ct{1942};
t6451 = ct{1943};
t6453 = ct{1944};
t6484 = ct{1945};
t6485 = ct{1946};
t6486 = ct{1947};
t649 = ct{1948};
t6493 = ct{1949};
t6506 = ct{1950};
t6507 = ct{1951};
t6508 = ct{1952};
t6511 = ct{1953};
t6515 = ct{1954};
t6520 = ct{1955};
t6529 = ct{1956};
t654 = ct{1957};
t6543 = ct{1958};
t6544 = ct{1959};
t655 = ct{1960};
t656 = ct{1961};
t6565 = ct{1962};
t657 = ct{1963};
t6575 = ct{1964};
t6576 = ct{1965};
t659 = ct{1966};
t6593 = ct{1967};
t660 = ct{1968};
t6611 = ct{1969};
t6612 = ct{1970};
t6658 = ct{1971};
t6663 = ct{1972};
t667 = ct{1973};
t668 = ct{1974};
t6689 = ct{1975};
t669 = ct{1976};
t6691 = ct{1977};
t6692 = ct{1978};
t67 = ct{1979};
t670 = ct{1980};
t674 = ct{1981};
t677 = ct{1982};
t68 = ct{1983};
t681 = ct{1984};
t6811 = ct{1985};
t6812 = ct{1986};
t6813 = ct{1987};
t682 = ct{1988};
t684 = ct{1989};
t685 = ct{1990};
t686 = ct{1991};
t6860 = ct{1992};
t6861 = ct{1993};
t687 = ct{1994};
t6892 = ct{1995};
t6893 = ct{1996};
t6913 = ct{1997};
t6916 = ct{1998};
t6917 = ct{1999};
t692 = ct{2000};
t6922 = ct{2001};
t693 = ct{2002};
t6937 = ct{2003};
t694 = ct{2004};
t6979 = ct{2005};
t6980 = ct{2006};
t6987 = ct{2007};
t6989 = ct{2008};
t7 = ct{2009};
t702 = ct{2010};
t7025 = ct{2011};
t7026 = ct{2012};
t7028 = ct{2013};
t7029 = ct{2014};
t7039 = ct{2015};
t7041 = ct{2016};
t7044 = ct{2017};
t7045 = ct{2018};
t7049 = ct{2019};
t7051 = ct{2020};
t7059 = ct{2021};
t707 = ct{2022};
t708 = ct{2023};
t7091 = ct{2024};
t71 = ct{2025};
t710 = ct{2026};
t715 = ct{2027};
t716 = ct{2028};
t7204 = ct{2029};
t721 = ct{2030};
t7219 = ct{2031};
t722 = ct{2032};
t7227 = ct{2033};
t7228 = ct{2034};
t7229 = ct{2035};
t7230 = ct{2036};
t724 = ct{2037};
t725 = ct{2038};
t73 = ct{2039};
t736 = ct{2040};
t738 = ct{2041};
t740 = ct{2042};
t741 = ct{2043};
t749 = ct{2044};
t762 = ct{2045};
t768 = ct{2046};
t777 = ct{2047};
t792 = ct{2048};
t793 = ct{2049};
t801 = ct{2050};
t802 = ct{2051};
t808 = ct{2052};
t813 = ct{2053};
t819 = ct{2054};
t821 = ct{2055};
t850 = ct{2056};
t855 = ct{2057};
t874 = ct{2058};
t878 = ct{2059};
t89 = ct{2060};
t92 = ct{2061};
t941 = ct{2062};
t948 = ct{2063};
t951 = ct{2064};
t97 = ct{2065};
et165 = t16.*t19.*t20.*t50.*t189.*(-3.279367663374749e-19)-t14.*t15.*t17.*t21.*t50.*t189.*7.075931802640439e-19;
et166 = t14.*t17.*t20.*t21.*t50.*t189.*(-1.190170786299927e-18)-t15.*t17.*t19.*t21.*t50.*t189.*1.190170786299927e-18;
et167 = t19.*t20.*t21.*t22.*t50.*t189.*(-3.226512155691387e-19);
t6365 = -t4975.*(et164+et165+et166+et167);
t6378 = -t3210.*(t3959+t4200-t4287+t4409+t3996.*(t2801-t2850)+t3992.*(t335-t1539-t2831+t2851));
t6407 = -t3483.*(t3959+t4200-t4287+t4409+t3996.*(t2801-t2850)+t3992.*(t335-t1539-t2831+t2851));
t6426 = t5975.*(t2694-t2701+t3036-t3043).*(t1513+t1879+t2598+t2820+t2834+t3117+t3118).*7.26735e-3;
t6431 = -t4780.*(t4510.*(t2813-t2835+t18.*(t1456-t2355).*1.02e-6+t23.*(t1456-t2355).*9.0e-8)+t4514.*(-t2804+t2838+t3109+t23.*(t1456-t2355).*9.3e-7)+t3132.*(t3235-t3535));
t6440 = -t4822.*(t4510.*(t2813-t2835+t18.*(t1456-t2355).*1.02e-6+t23.*(t1456-t2355).*9.0e-8)+t4514.*(-t2804+t2838+t3109+t23.*(t1456-t2355).*9.3e-7)+t3132.*(t3235-t3535));
t6441 = t4822.*(t4510.*(t2813-t2835+t18.*(t1456-t2355).*1.02e-6+t23.*(t1456-t2355).*9.0e-8)+t4514.*(-t2804+t2838+t3109+t23.*(t1456-t2355).*9.3e-7)+t3132.*(t3235-t3535));
t6452 = -t3877.*(t3959+t4200-t4287+t4409+t3996.*(t2801-t2850)+t3992.*(t335-t1539-t2831+t2851));
t6481 = -t4514.*(t4555+t4571-t18.*t2363.*t3047.*9.0e-8-t23.*t2363.*t3047.*9.3e-7+t18.*t3946.*(t1896-t3232).*9.0e-8+t23.*t3946.*(t1896-t3232).*9.3e-7);
et168 = t1288+t1289+t1302+t1303-t1319-t1320+t1336-t1348+t1350+t1351-t1360+t1369-t1378+t1396-t1425+t1435-t2174+t2183-t2187+t2193-t2194-t2195+t2199-t2203-t2215+t2219-t2222-t2223+t2239+t2240-t2256-t2257+t2555+t2556+t2572+t2583-t2605-t2606+t2612+t2613-t2618-t2619+t2651+t2652;
et169 = t24.*t25.*t26.*t50.*t202.*(-3.566935413776081e-21);
et170 = t30.*t31.*t32.*t50.*t202.*(-3.992732227073824e-24);
et171 = t24.*t25.*t32.*t33.*t50.*t202.*(-3.509445006623964e-21);
et172 = t27.*t30.*t31.*t32.*t50.*t202.*(-7.696420262413979e-21);
t6497 = -t4651.*(et168+et169+et170+et171+et172);
et173 = t1288+t1289+t1302+t1303-t1319-t1320+t1336-t1348+t1350+t1351-t1360+t1369-t1378+t1396-t1425+t1435-t2174+t2183-t2187+t2193-t2194-t2195+t2199-t2203-t2215+t2219-t2222-t2223+t2239+t2240-t2256-t2257+t2555+t2556+t2572+t2583-t2605-t2606+t2612+t2613-t2618-t2619+t2651+t2652;
et174 = t24.*t25.*t26.*t50.*t202.*(-3.566935413776081e-21);
et175 = t30.*t31.*t32.*t50.*t202.*(-3.992732227073824e-24);
et176 = t24.*t25.*t32.*t33.*t50.*t202.*(-3.509445006623964e-21);
et177 = t27.*t30.*t31.*t32.*t50.*t202.*(-7.696420262413979e-21);
t6498 = t4651.*(et173+et174+et175+et176+et177);
t6521 = -t6520;
et178 = t1288+t1289+t1302+t1303-t1319-t1320+t1336-t1348+t1350+t1351-t1360+t1369-t1378+t1396-t1425+t1435-t2174+t2183-t2187+t2193-t2194-t2195+t2199-t2203-t2215+t2219-t2222-t2223+t2239+t2240-t2256-t2257+t2555+t2556+t2572+t2583-t2605-t2606+t2612+t2613-t2618-t2619+t2651+t2652;
et179 = t24.*t25.*t26.*t50.*t202.*(-3.566935413776081e-21);
et180 = t30.*t31.*t32.*t50.*t202.*(-3.992732227073824e-24);
et181 = t24.*t25.*t32.*t33.*t50.*t202.*(-3.509445006623964e-21);
et182 = t27.*t30.*t31.*t32.*t50.*t202.*(-7.696420262413979e-21);
t6528 = -t4897.*(et178+et179+et180+et181+et182);
t6530 = -t6529;
t6533 = t3057.*t6506;
t6566 = t2736+t2797+t2937+t2942+t3004+t3008+t3965+t4190+t4208+t4217+t4892+t4894;
et183 = t707+t708-t721-t722-t749+t762+t768-t777-t792-t793-t801-t802-t808+t813-t819+t821-t1629+t1637-t1640-t1641-t1659-t1661+t1666+t1667+t1683+t1692+t1705-t1712+t1758+t1759+t1775+t1776+t1973+t1993+t1994+t2023+t2053+t2060-t2089-t2090+t2098+t2099-t14.*t15.*t21.*t50.*t189.*3.670836568391568e-22;
et184 = t16.*t19.*t20.*t50.*t189.*(-3.279367663374749e-19)-t14.*t15.*t17.*t21.*t50.*t189.*7.075931802640439e-19;
et185 = t14.*t17.*t20.*t21.*t50.*t189.*(-1.190170786299927e-18)-t15.*t17.*t19.*t21.*t50.*t189.*1.190170786299927e-18;
et186 = t19.*t20.*t21.*t22.*t50.*t189.*(-3.226512155691387e-19);
t6584 = -t5539.*(et183+et184+et185+et186);
t6632 = -t6506.*(t3235-t3535);
t6633 = t3992.*t6506;
t6634 = t6506.*(t3235-t3535);
t6646 = t3333+t3441+t4881+t4888+t5118+t5124;
et187 = t1288+t1289+t1302+t1303-t1319-t1320+t1336-t1348+t1350+t1351-t1360+t1369-t1378+t1396-t1425+t1435-t2174+t2183-t2187+t2193-t2194-t2195+t2199-t2203-t2215+t2219-t2222-t2223+t2239+t2240-t2256-t2257+t2555+t2556+t2572+t2583-t2605-t2606+t2612+t2613-t2618-t2619+t2651+t2652;
et188 = t24.*t25.*t26.*t50.*t202.*(-3.566935413776081e-21);
et189 = t30.*t31.*t32.*t50.*t202.*(-3.992732227073824e-24);
et190 = t24.*t25.*t32.*t33.*t50.*t202.*(-3.509445006623964e-21);
et191 = t27.*t30.*t31.*t32.*t50.*t202.*(-7.696420262413979e-21);
t6752 = -t5412.*(et187+et188+et189+et190+et191);
t6873 = -t2363.*(t3156+t3157+t3376-t4255-t4256-t4499+t4504+t3524.*(t1861-t3214).*6.2e-7+t3481.*(t1896-t3232).*6.2e-7-(t17.*(t1861-t3214).*(t1896-t3232))./1.0e+8-(t17.*t2297.*t2363)./1.0e+8-(t17.*t3483.*t3528)./1.0e+8);
t6924 = -t6922;
t6927 = (t1896-t3232).*(t3156+t3157+t3376-t4255-t4256-t4499+t4504+t3524.*(t1861-t3214).*6.2e-7+t3481.*(t1896-t3232).*6.2e-7-(t17.*(t1861-t3214).*(t1896-t3232))./1.0e+8-(t17.*t2297.*t2363)./1.0e+8-(t17.*t3483.*t3528)./1.0e+8);
t6928 = -t3528.*(t3156+t3157+t3376-t4255-t4256-t4499+t4504+t3524.*(t1861-t3214).*6.2e-7+t3481.*(t1896-t3232).*6.2e-7-(t17.*(t1861-t3214).*(t1896-t3232))./1.0e+8-(t17.*t2297.*t2363)./1.0e+8-(t17.*t3483.*t3528)./1.0e+8);
t6954 = -t3057.*(t5232-t5274+t5275+t3901.*(t17.*((t237.*(t42-t43))./9.007199254740992e+15+t21.*(-t1881+t3121+t3269))+t22.*(-t1901+t3122+t3270)).*1.02e-6);
t6955 = t3057.*(t5232-t5274+t5275+t3901.*(t17.*((t237.*(t42-t43))./9.007199254740992e+15+t21.*(-t1881+t3121+t3269))+t22.*(-t1901+t3122+t3270)).*1.02e-6);
t6975 = t5213+t5752+t5767;
t6988 = -t6987;
t6990 = -t6989;
t7012 = (t3235-t3535).*(t5232-t5274+t5275+t3901.*(t17.*((t237.*(t42-t43))./9.007199254740992e+15+t21.*(-t1881+t3121+t3269))+t22.*(-t1901+t3122+t3270)).*1.02e-6);
t7015 = -t3992.*(t5232-t5274+t5275+t3901.*(t17.*((t237.*(t42-t43))./9.007199254740992e+15+t21.*(-t1881+t3121+t3269))+t22.*(-t1901+t3122+t3270)).*1.02e-6);
t7027 = -t7025;
t7042 = t1599+t1704+t2360+t2391+t2404+t2405+t2438+t2472+t2575+t2638+t2984+t2987+t3179+t3384+t3916+t3954+t3964+t4150+t4179+t4184+t4863+t4864;
t7054 = -t3882.*(-t5209+t5751+t5639.*(t1896-t3232));
t7055 = t3882.*(-t5209+t5751+t5639.*(t1896-t3232));
t7062 = -t7059;
t7065 = t1613+t2360+t2448+t2449+t2461+t2471+t2492+t2575+t2638+t2984+t2987+t3949+t3958+t3962+t4178+t4179+t4184+t4189+t4863+t4864;
t7107 = -t4822.*(-t5209+t5751+t5639.*(t1896-t3232));
t7181 = t5472+t5999+t6014;
t7193 = t3162+t3163+t3249+t3382+t4604+t4606+t4607+t4609+t4866+t4867+t5094+t5096;
t7279 = -t2363.*(-t5165+t5219+t5270-t5272+t4865.*(t1861-t3214).*6.2e-7+t3901.*(t951+t16.*(-t1881+t3121+t3269)).*6.2e-7+t4080.*(t2694-t2701+t3036-t3043).*6.2e-7+(t4780.*(t2694-t2701+t3036-t3043))./1.0e+8);
t7280 = t2363.*(-t5165+t5219+t5270-t5272+t4865.*(t1861-t3214).*6.2e-7+t3901.*(t951+t16.*(-t1881+t3121+t3269)).*6.2e-7+t4080.*(t2694-t2701+t3036-t3043).*6.2e-7+(t4780.*(t2694-t2701+t3036-t3043))./1.0e+8);
t7291 = (t1896-t3232).*(-t5165+t5219+t5270-t5272+t4865.*(t1861-t3214).*6.2e-7+t3901.*(t951+t16.*(-t1881+t3121+t3269)).*6.2e-7+t4080.*(t2694-t2701+t3036-t3043).*6.2e-7+(t4780.*(t2694-t2701+t3036-t3043))./1.0e+8);
t7292 = -t3528.*(-t5165+t5219+t5270-t5272+t4865.*(t1861-t3214).*6.2e-7+t3901.*(t951+t16.*(-t1881+t3121+t3269)).*6.2e-7+t4080.*(t2694-t2701+t3036-t3043).*6.2e-7+(t4780.*(t2694-t2701+t3036-t3043))./1.0e+8);
t7294 = t3528.*(-t5165+t5219+t5270-t5272+t4865.*(t1861-t3214).*6.2e-7+t3901.*(t951+t16.*(-t1881+t3121+t3269)).*6.2e-7+t4080.*(t2694-t2701+t3036-t3043).*6.2e-7+(t4780.*(t2694-t2701+t3036-t3043))./1.0e+8);
t7723 = t5369+t5806+t5826+t6153+t7026+t7045;
et192 = t3015-t3068+t4415-t4461+t3481.*(t1959-t3306+t38.*t1022.*(t855-t878).*2.196325630278387e-1).*9.840000000000001e-6;
et193 = t3230.*((t237.*(t42-t43))./9.007199254740992e+15+t21.*(-t1881+t3121+t3269)).*9.840000000000001e-6;
t7731 = -t3209.*(t5370+t5827+t7025+t5640.*(t1959-t3306+t38.*t1022.*(t855-t878).*2.196325630278387e-1)+t6980.*(t1896-t3232)+t3524.*(et192+et193));
et194 = t3015-t3068+t4415-t4461+t3481.*(t1959-t3306+t38.*t1022.*(t855-t878).*2.196325630278387e-1).*9.840000000000001e-6;
et195 = t3230.*((t237.*(t42-t43))./9.007199254740992e+15+t21.*(-t1881+t3121+t3269)).*9.840000000000001e-6;
t7732 = t3209.*(t5370+t5827+t7025+t5640.*(t1959-t3306+t38.*t1022.*(t855-t878).*2.196325630278387e-1)+t6980.*(t1896-t3232)+t3524.*(et194+et195));
et196 = t3015-t3068+t4415-t4461+t3481.*(t1959-t3306+t38.*t1022.*(t855-t878).*2.196325630278387e-1).*9.840000000000001e-6;
et197 = t3230.*((t237.*(t42-t43))./9.007199254740992e+15+t21.*(-t1881+t3121+t3269)).*9.840000000000001e-6;
t7734 = (t2674-t2676+t3022-t3027).*(t5370+t5827+t7025+t5640.*(t1959-t3306+t38.*t1022.*(t855-t878).*2.196325630278387e-1)+t6980.*(t1896-t3232)+t3524.*(et196+et197));
t7790 = t5598+t6059+t6085+t6576+t7227+t7230;
t4034 = t3972.*9.99471e-3;
t4035 = t3973.*9.99471e-3;
t4036 = t3972.*1.838876e-2;
t4037 = t3973.*1.838876e-2;
t4086 = t4014.*1.838876e-2;
t4089 = t4013.*9.99471e-3;
t4090 = t4014.*9.99471e-3;
t4091 = t4013.*1.838876e-2;
t4145 = t4013.*1.33637554986e-4;
t4146 = t4014.*1.33637554986e-4;
t4147 = t4013.*7.26350557185e-5;
t4148 = t4014.*7.26350557185e-5;
t4320 = -t4315;
t4397 = -t4393;
t4398 = -t4394;
t4494 = t3491+t3973;
t4495 = t3503+t3972;
t4523 = -t4519;
t4529 = t3230.*t4226.*1.02e-6;
t4534 = -t4527;
t4540 = t3230.*t4226.*9.0e-8;
t4541 = t3543+t4014;
t4553 = t3550+t4013;
t4565 = -t4556;
t4575 = -t4570;
t4580 = -t4576;
t4600 = -t4598;
t4636 = t3528.*t4226.*1.02e-6;
t4638 = t3528.*t4226.*9.0e-8;
t4677 = -t4674;
t4715 = -t4714;
t4761 = -t4751;
t4763 = -t4752;
t4771 = -t4765;
t4773 = -t4767;
t4775 = -t4774;
t4807 = t3230.*(t3493-t3972).*(-9.3e-7);
t4808 = t3230.*(t3493-t3972).*(-1.02e-6);
t4812 = t3230.*(t3493-t3972).*(-9.0e-8);
t4854 = -t4850;
t4855 = -t4851;
t4907 = t3901.*t4226.*1.02e-6;
t4909 = t3901.*t4226.*9.0e-8;
t4915 = -t4912;
t4920 = -t4916;
t4923 = t27.*t4914;
t4926 = t27.*t4918;
t4928 = t27.*t4919;
t4930 = t27.*t4924;
t4937 = t3528.*(t3493-t3972).*(-9.3e-7);
t4938 = t3528.*(t3493-t3972).*(-1.02e-6);
t4941 = t3528.*(t3493-t3972).*9.3e-7;
t4942 = t3531.*(t3493-t3972).*(-1.02e-6);
t4943 = t3528.*(t3493-t3972).*(-9.0e-8);
t4946 = t3528.*(t3493-t3972).*9.0e-8;
t4947 = t3531.*(t3493-t3972).*(-9.0e-8);
t4956 = -t4955;
t4958 = t3992.*t4226.*1.02e-6;
t4959 = -t4957;
t4960 = t3992.*t4226.*9.0e-8;
t4971 = -t4248.*(t2813-t2835+t18.*(t1456-t2355).*1.02e-6+t23.*(t1456-t2355).*9.0e-8);
t4972 = t4248.*(t2813-t2835+t18.*(t1456-t2355).*1.02e-6+t23.*(t1456-t2355).*9.0e-8);
t4981 = -t3737.*(t3544-t4013);
t5008 = -t3845.*(t3544-t4013);
t5082 = t3901.*(t3493-t3972).*(-9.3e-7);
t5083 = t3901.*(t3493-t3972).*(-1.02e-6);
t5085 = t3904.*(t3493-t3972).*(-1.02e-6);
t5086 = t3901.*(t3493-t3972).*9.3e-7;
t5087 = t3901.*(t3493-t3972).*(-9.0e-8);
t5088 = t3904.*(t3493-t3972).*(-9.0e-8);
t5089 = t3901.*(t3493-t3972).*9.0e-8;
t5099 = -t5097;
t5100 = -t5098;
t5102 = -t3945.*(t3544-t4013);
t5135 = t3992.*(t3493-t3972).*(-9.3e-7);
t5137 = t3992.*(t3493-t3972).*(-1.02e-6);
t5138 = t3992.*(t3493-t3972).*9.3e-7;
t5139 = t3992.*(t3493-t3972).*(-9.0e-8);
t5141 = t3996.*(t3493-t3972).*(-1.02e-6);
t5142 = t3992.*(t3493-t3972).*9.0e-8;
t5143 = t3996.*(t3493-t3972).*(-9.0e-8);
t5172 = t4113.*(t3493-t3972).*(-1.02e-6);
t5173 = t4113.*(t3493-t3972).*(-9.0e-8);
t5185 = (t3544-t4013).*(-t2804+t2838+t3109+t23.*(t1456-t2355).*9.3e-7);
t5186 = (t3544-t4013).*(t2813-t2835+t18.*(t1456-t2355).*1.02e-6+t23.*(t1456-t2355).*9.0e-8);
t5187 = -t4125.*(t3544-t4013);
t5283 = -t5278;
t5287 = -t5286;
t5309 = t50.*t189.*t5258.*9.543032792050485e-17;
t5311 = t50.*t189.*t5262.*9.543032792050485e-17;
t5323 = t3577+t3578+t4007+t4018;
t5326 = t50.*t202.*t5300.*6.935255936130809e-19;
t5329 = t3218+t4354+t4361;
t5341 = t3623+t3624+t4072+t4075;
t5352 = t3259+t4370+t4392;
t5366 = t3699+t3703+t4120+t4130;
t5400 = t27.*t2363.*t5351;
t5414 = t3003.*t5351;
t5423 = t4814.*(t3493-t3972).*(-1.02e-6);
t5424 = t4814.*(t3493-t3972).*(-9.0e-8);
t5430 = t3377+t4498+t4506;
t5432 = t3057.*t5351;
t5435 = -t5351.*(t1477-t2502);
t5437 = t56+t73+t5413;
t5438 = t5351.*(t1477-t2502);
t5442 = t71+t97+t5413;
t5450 = -t5447;
t5456 = -t5453;
t5464 = t4860.*(t3493-t3972).*(-1.02e-6);
t5466 = t4860.*(t3493-t3972).*(-9.0e-8);
t5478 = t3423+t4528+t4548;
t5479 = t3427+t4521+t4558;
t5507 = -t5506;
t5511 = -t27.*t5351.*(t1896-t3232);
t5512 = t27.*t3528.*t5351;
t5513 = t27.*t5351.*(t1896-t3232);
t5530 = -t5528;
t5563 = -t2363.*(t4714+(t3942.*(t2694-t2701+t3036-t3043))./1.0e+8);
t5568 = t2363.*(t4714+(t3942.*(t2694-t2701+t3036-t3043))./1.0e+8);
t5585 = t27.*t2363.*t5520;
t5590 = t326+t339+t5548;
t5591 = t362+t380+t5548;
t5596 = -t5594;
t5610 = t2294+t2325+t3295+t3309+t5220;
t5615 = t3003.*t5520;
t5623 = -t3057.*(t4752+t3942.*(t2694-t2701+t3036-t3043).*1.02e-6);
t5624 = t3057.*t5520;
t5625 = -t5520.*(t1477-t2502);
t5629 = -t5628;
t5636 = -t5632;
t5641 = t2297.*t5584;
t5644 = t2297.*t5587;
t5648 = t3985.*t5351;
t5649 = -t5351.*(t3235-t3535);
t5651 = t3992.*t5351;
t5653 = t5351.*(t3235-t3535);
t5655 = t3996.*t5351;
t5665 = t2297.*t5609;
t5680 = t2363.*t5618.*7.26735e-3;
t5686 = t50.*t202.*t5643.*6.935255936130809e-19;
t5696 = (t4714+(t3942.*(t2694-t2701+t3036-t3043))./1.0e+8).*(t1896-t3232);
t5697 = -t3528.*(t4714+(t3942.*(t2694-t2701+t3036-t3043))./1.0e+8);
t5698 = t3528.*(t4714+(t3942.*(t2694-t2701+t3036-t3043))./1.0e+8);
t5704 = t2363.*t5642.*7.26735e-3;
t5714 = -t27.*t5520.*(t1896-t3232);
t5715 = t27.*t3528.*t5520;
t5756 = t4202+t4626+t4672;
t5757 = t4404+t5354;
t5762 = t27.*t2363.*t5739;
t5771 = t3003.*t5739;
t5772 = t3985.*t5520;
t5773 = (t4752+t3942.*(t2694-t2701+t3036-t3043).*1.02e-6).*(t3235-t3535);
t5774 = -t5520.*(t3235-t3535);
t5776 = -t3992.*(t4752+t3942.*(t2694-t2701+t3036-t3043).*1.02e-6);
t5777 = t3992.*t5520;
t5778 = t5520.*(t3235-t3535);
t5780 = t3996.*t5520;
t5783 = t4434+t5375;
t5787 = t3057.*t5739;
t5788 = -t5739.*(t1477-t2502);
t5789 = t4587+t5360;
t5798 = t58+t59+t5796;
t5799 = t429+t5796;
t5802 = t4611+t5394;
t5808 = t3732.*t5426.*(t2694-t2701+t3036-t3043).*(-1.08769e-2);
t5809 = t3732.*t5429.*(t2694-t2701+t3036-t3043).*(-1.08769e-2);
t5812 = t3732.*t3901.*(t410-t5413).*(-1.08769e-2);
t5813 = t3732.*t3901.*(t410-t5413).*1.08769e-2;
t5814 = -t27.*t5739.*(t1896-t3232);
t5815 = t27.*t3528.*t5739;
t5816 = t27.*t5739.*(t1896-t3232);
t5818 = -t5817;
t5820 = t3784.*t5426.*(t2694-t2701+t3036-t3043).*(-1.08769e-2);
t5821 = t3784.*t5429.*(t2694-t2701+t3036-t3043).*(-1.08769e-2);
t5824 = t3784.*t3901.*(t410-t5413).*(-1.08769e-2);
t5825 = t3784.*t3901.*(t410-t5413).*1.08769e-2;
t5829 = t4814.*t5351;
t5830 = -t5351.*(t4127+t33.*(t1959-t3306+t38.*t1022.*(t855-t878).*2.196325630278387e-1));
t5831 = t5351.*(t4127+t33.*(t1959-t3306+t38.*t1022.*(t855-t878).*2.196325630278387e-1));
t5833 = t3901.*t5220.*(t1513+t1879+t2598+t2820+t2834+t3117+t3118).*(-7.26735e-3);
t5836 = t5258.*(t2694-t2701+t3036-t3043).*(t1513+t1879+t2598+t2820+t2834+t3117+t3118).*7.26735e-3;
t5838 = t3901.*t5262.*(t1513+t1879+t2598+t2820+t2834+t3117+t3118).*(-7.26735e-3);
t5842 = t4716.*t5426;
t5845 = t4716.*t5429;
t5850 = -t3877.*t5314.*(t1488+t1874+t2519+t2740+t2747+t3096+t3097);
t5851 = (t410-t5413).*(t3410-t3708+t3714+t26.*t50.*t202.*(t46-t47).*8.687615694748404e-39);
t5863 = t4175.*t5413.*(t2694-t2701+t3036-t3043).*(-1.08769e-2);
t5865 = -t3877.*t5321.*(t1488+t1874+t2519+t2740+t2747+t3096+t3097);
t5870 = -t5867;
t5873 = t3901.*t4175.*t5426.*1.08769e-2;
t5877 = t3985.*t5739;
t5878 = -t5739.*(t3235-t3535);
t5881 = t3992.*t5739;
t5882 = t5739.*(t3235-t3535);
t5883 = t3996.*t5739;
t5884 = t331+t333+t5843;
t5887 = -t3689.*t5588.*(t2674-t2676+t3022-t3027);
t5888 = t356+t372+t5843;
t5889 = -t3689.*t5589.*(t2674-t2676+t3022-t3027);
t5902 = -t5901;
t5917 = -t3782.*t5588.*(t2674-t2676+t3022-t3027);
t5918 = -t3782.*t5589.*(t2674-t2676+t3022-t3027);
t5924 = -t5923;
t5926 = t2363.*t5854;
t5927 = t2388.*t5854;
t5929 = t2419.*t5854;
t5935 = t4973.*t5426;
t5937 = t4973.*t5429;
t5940 = -t4975.*(t410-t5413);
t5945 = t4649.*t5588;
t5947 = t4649.*t5589;
t5956 = t4814.*t5520;
t5957 = -t5520.*(t4127+t33.*(t1959-t3306+t38.*t1022.*(t855-t878).*2.196325630278387e-1));
t5959 = -t3891.*t5588.*(t2674-t2676+t3022-t3027);
t5960 = -t3891.*t5589.*(t2674-t2676+t3022-t3027);
t5963 = -t5961;
t5967 = -t4134.*t5548.*(t2674-t2676+t3022-t3027);
t5968 = t4134.*t5548.*(t2674-t2676+t3022-t3027);
t5972 = t3877.*t4134.*t5588;
t5978 = t3524.*t5854;
t5979 = -t5854.*(t1896-t3232);
t5980 = t3528.*t5854;
t5981 = t3531.*t5854;
t5986 = t4886.*t5588;
t5988 = t4886.*t5589;
t5997 = -t5996;
t6001 = t3153+t3373+t4251+t4252+t4501+t4503;
t6008 = t3159+t3434+t4254+t4261+t4522+t4557;
t6035 = t3260+t3262+t4369+t4379+t4388+t4391;
t6039 = t3258+t3265+t4380+t4386+t4389+t4396;
t6040 = t4306+t5175+t5178;
t6042 = t4113.*t5854;
t6043 = -t5854.*(t1005+t26.*(t1941-t3308+t39.*t1022.*(t855-t878).*2.196325630278387e-1));
t6046 = t4814.*t5739;
t6047 = -t5739.*(t4127+t33.*(t1959-t3306+t38.*t1022.*(t855-t878).*2.196325630278387e-1));
t6088 = t4460+t4464+t4708+t4712;
t6100 = t5224.*t5588;
t6103 = -t6101;
t6104 = t5224.*t5589;
t6119 = t3385.*t6038;
t6138 = t4134.*t4822.*t5588;
t6140 = t4134.*t4822.*t5589;
t6150 = -t6147;
t6160 = t5426.*t5486;
t6161 = t5429.*t5486;
t6163 = -t6162;
t6165 = t638+t654+t655+t657+t1576+t1579+t1584+t1585+t2291+t2311+t2671+t2683+t2684+t2696+t3029+t3226+t3281+t3300+t3512+t3576+t3588+t4015+t4016;
t6167 = -t5485.*(t410-t5413);
t6168 = t5485.*(t410-t5413);
t6173 = t3422+t3443+t4526+t4532+t4547+t4570;
t6175 = t3436+t3437+t4530+t4536+t4561+t4569;
t6176 = t3430+t3445+t4539+t4545+t4564+t4577;
t6177 = t3429+t3446+t4538+t4546+t4563+t4578;
t6189 = t3447+t3455+t4550+t4567+t4583+t4586;
t6201 = t692+t693+t702+t738+t1614+t1631+t1648+t1649+t2344+t2421+t2698+t2707+t2717+t2719+t3044+t3246+t3328+t3347+t3562+t3622+t3634+t4076+t4077;
t6202 = (t5359+t4108.*(t1861-t3214)).*(t2694-t2701+t3036-t3043).*(t1513+t1879+t2598+t2820+t2834+t3117+t3118).*(-7.26735e-3);
t6210 = -t33.*t2363.*(t3424-t3437+t4552+t4556+t3942.*(t1896-t3232).*5.7e-7+t3946.*(t1896-t3232).*4.0e-8);
t6211 = t33.*t2363.*(t3424-t3437+t4552+t4556+t3942.*(t1896-t3232).*5.7e-7+t3946.*(t1896-t3232).*4.0e-8);
t6223 = t3901.*t5796.*(t1513+t1879+t2598+t2820+t2834+t3117+t3118).*(-7.26735e-3);
t6224 = t3901.*t5796.*(t1513+t1879+t2598+t2820+t2834+t3117+t3118).*7.26735e-3;
t6244 = -t2998.*(t3424-t3437+t4552+t4556+t3942.*(t1896-t3232).*5.7e-7+t3946.*(t1896-t3232).*4.0e-8);
t6245 = t5426.*t5548;
t6248 = t5429.*t5548;
t6251 = -t5539.*(t410-t5413);
t6267 = -t3057.*(t3424-t3437+t4552+t4556+t3942.*(t1896-t3232).*5.7e-7+t3946.*(t1896-t3232).*4.0e-8);
t6271 = (t1477-t2502).*(t3424-t3437+t4552+t4556+t3942.*(t1896-t3232).*5.7e-7+t3946.*(t1896-t3232).*4.0e-8);
t6279 = -t2297.*(t642+t643-t667+t674+t1587+t1606+t1608+t1609+t2295+t2671+t2683+t2684-t2695+t3272+t3290-t3296+t3576+t3582+t3588-t3593+t4015+t4016);
